simulink model "SIM_EXO_DAL_MN"  (R2021b)
(part 16 of 24)

t3493 = ct{698};
t3496 = ct{699};
t3498 = ct{700};
t3499 = ct{701};
t3500 = ct{702};
t3501 = ct{703};
t3504 = ct{704};
t3506 = ct{705};
t3507 = ct{706};
t3510 = ct{707};
t3511 = ct{708};
t3513 = ct{709};
t3514 = ct{710};
t3515 = ct{711};
t3517 = ct{712};
t3518 = ct{713};
t3521 = ct{714};
t3522 = ct{715};
t3523 = ct{716};
t3526 = ct{717};
t3530 = ct{718};
t3531 = ct{719};
t3532 = ct{720};
t3535 = ct{721};
t3536 = ct{722};
t3539 = ct{723};
t3540 = ct{724};
t3542 = ct{725};
t3543 = ct{726};
t3547 = ct{727};
t3554 = ct{728};
t3556 = ct{729};
t3557 = ct{730};
t356 = ct{731};
t3562 = ct{732};
t3568 = ct{733};
t3569 = ct{734};
t357 = ct{735};
t3571 = ct{736};
t3574 = ct{737};
t3577 = ct{738};
t3578 = ct{739};
t358 = ct{740};
t3582 = ct{741};
t3583 = ct{742};
t3584 = ct{743};
t3585 = ct{744};
t3592 = ct{745};
t3593 = ct{746};
t3605 = ct{747};
t3606 = ct{748};
t3607 = ct{749};
t361 = ct{750};
t3610 = ct{751};
t3611 = ct{752};
t3612 = ct{753};
t3618 = ct{754};
t3634 = ct{755};
t3635 = ct{756};
t3637 = ct{757};
t3642 = ct{758};
t3644 = ct{759};
t3656 = ct{760};
t3658 = ct{761};
t3659 = ct{762};
t3662 = ct{763};
t3666 = ct{764};
t3667 = ct{765};
t3668 = ct{766};
t3673 = ct{767};
t3678 = ct{768};
t3682 = ct{769};
t3694 = ct{770};
t3702 = ct{771};
t3706 = ct{772};
t3708 = ct{773};
t371 = ct{774};
t3719 = ct{775};
t372 = ct{776};
t3725 = ct{777};
t3726 = ct{778};
t373 = ct{779};
t3732 = ct{780};
t3733 = ct{781};
t3734 = ct{782};
t3738 = ct{783};
t374 = ct{784};
t3743 = ct{785};
t3746 = ct{786};
t3753 = ct{787};
t3755 = ct{788};
t3757 = ct{789};
t3759 = ct{790};
t3761 = ct{791};
t3763 = ct{792};
t3765 = ct{793};
t3767 = ct{794};
t377 = ct{795};
t3772 = ct{796};
t378 = ct{797};
t3783 = ct{798};
t3785 = ct{799};
t3788 = ct{800};
t379 = ct{801};
t3792 = ct{802};
t3819 = ct{803};
t3821 = ct{804};
t3822 = ct{805};
t3824 = ct{806};
t3831 = ct{807};
t3843 = ct{808};
t3845 = ct{809};
t3851 = ct{810};
t3852 = ct{811};
t3863 = ct{812};
t3869 = ct{813};
t3871 = ct{814};
t3873 = ct{815};
t3874 = ct{816};
t3875 = ct{817};
t3876 = ct{818};
t3882 = ct{819};
t3884 = ct{820};
t3889 = ct{821};
t3890 = ct{822};
t3891 = ct{823};
t3907 = ct{824};
t391 = ct{825};
t3910 = ct{826};
t3913 = ct{827};
t3921 = ct{828};
t3922 = ct{829};
t3923 = ct{830};
t3944 = ct{831};
t395 = ct{832};
t3951 = ct{833};
t3954 = ct{834};
t3956 = ct{835};
t3957 = ct{836};
t3959 = ct{837};
t3960 = ct{838};
t3968 = ct{839};
t3969 = ct{840};
t3971 = ct{841};
t3972 = ct{842};
t3976 = ct{843};
t3978 = ct{844};
t3979 = ct{845};
t3992 = ct{846};
t3993 = ct{847};
t3995 = ct{848};
t3997 = ct{849};
t4 = ct{850};
t4000 = ct{851};
t4004 = ct{852};
t401 = ct{853};
t4010 = ct{854};
t4011 = ct{855};
t4014 = ct{856};
t4015 = ct{857};
t402 = ct{858};
t403 = ct{859};
t406 = ct{860};
t4089 = ct{861};
t4099 = ct{862};
t410 = ct{863};
t4100 = ct{864};
t4103 = ct{865};
t4108 = ct{866};
t411 = ct{867};
t4113 = ct{868};
t4115 = ct{869};
t4118 = ct{870};
t4119 = ct{871};
t4121 = ct{872};
t4123 = ct{873};
t4126 = ct{874};
t413 = ct{875};
t4132 = ct{876};
t4134 = ct{877};
t4138 = ct{878};
t414 = ct{879};
t4143 = ct{880};
t4146 = ct{881};
t4148 = ct{882};
t4152 = ct{883};
t4153 = ct{884};
t4158 = ct{885};
t4166 = ct{886};
t4173 = ct{887};
t4178 = ct{888};
t4179 = ct{889};
t418 = ct{890};
t4181 = ct{891};
t4183 = ct{892};
t4185 = ct{893};
t4190 = ct{894};
t4196 = ct{895};
t4197 = ct{896};
t4206 = ct{897};
t4208 = ct{898};
t4210 = ct{899};
t4217 = ct{900};
t422 = ct{901};
t4221 = ct{902};
t4223 = ct{903};
t4226 = ct{904};
t4228 = ct{905};
t423 = ct{906};
t4230 = ct{907};
t4232 = ct{908};
t4234 = ct{909};
t424 = ct{910};
t4243 = ct{911};
t4249 = ct{912};
t425 = ct{913};
t4251 = ct{914};
t4254 = ct{915};
t4255 = ct{916};
t4259 = ct{917};
t4261 = ct{918};
t4263 = ct{919};
t427 = ct{920};
t4274 = ct{921};
t4276 = ct{922};
t4278 = ct{923};
t4279 = ct{924};
t428 = ct{925};
t4285 = ct{926};
t4286 = ct{927};
t429 = ct{928};
t4293 = ct{929};
t4298 = ct{930};
t4301 = ct{931};
t4304 = ct{932};
t4306 = ct{933};
t431 = ct{934};
t4317 = ct{935};
t4318 = ct{936};
t432 = ct{937};
t4327 = ct{938};
t4329 = ct{939};
t433 = ct{940};
t4332 = ct{941};
t4335 = ct{942};
t4337 = ct{943};
t4339 = ct{944};
t434 = ct{945};
t4342 = ct{946};
t4344 = ct{947};
t4345 = ct{948};
t4347 = ct{949};
t4348 = ct{950};
t4349 = ct{951};
t435 = ct{952};
t4350 = ct{953};
t436 = ct{954};
t4369 = ct{955};
t4370 = ct{956};
t4378 = ct{957};
t4380 = ct{958};
t4382 = ct{959};
t4385 = ct{960};
t4388 = ct{961};
t4392 = ct{962};
t4394 = ct{963};
t4395 = ct{964};
t4396 = ct{965};
t4397 = ct{966};
t440 = ct{967};
t4402 = ct{968};
t4403 = ct{969};
t4405 = ct{970};
t4406 = ct{971};
t4407 = ct{972};
t441 = ct{973};
t4410 = ct{974};
t4412 = ct{975};
t4413 = ct{976};
t4414 = ct{977};
t4416 = ct{978};
t4417 = ct{979};
t4418 = ct{980};
t4419 = ct{981};
t442 = ct{982};
t4420 = ct{983};
t4423 = ct{984};
t4425 = ct{985};
t4426 = ct{986};
t4428 = ct{987};
t4429 = ct{988};
t4431 = ct{989};
t4436 = ct{990};
t4437 = ct{991};
t444 = ct{992};
t4440 = ct{993};
t4444 = ct{994};
t4446 = ct{995};
t4447 = ct{996};
t4449 = ct{997};
t445 = ct{998};
t4450 = ct{999};
t4453 = ct{1000};
t4462 = ct{1001};
t4467 = ct{1002};
t4468 = ct{1003};
t4469 = ct{1004};
t4471 = ct{1005};
t4473 = ct{1006};
t4475 = ct{1007};
t4478 = ct{1008};
t4479 = ct{1009};
t448 = ct{1010};
t4482 = ct{1011};
t4483 = ct{1012};
t4485 = ct{1013};
t4486 = ct{1014};
t4487 = ct{1015};
t4488 = ct{1016};
t4489 = ct{1017};
t449 = ct{1018};
t4490 = ct{1019};
t4494 = ct{1020};
t4495 = ct{1021};
t4498 = ct{1022};
t4499 = ct{1023};
t450 = ct{1024};
t4500 = ct{1025};
t4501 = ct{1026};
t4502 = ct{1027};
t4505 = ct{1028};
t4506 = ct{1029};
t4509 = ct{1030};
t4510 = ct{1031};
t4515 = ct{1032};
t4518 = ct{1033};
t4519 = ct{1034};
t452 = ct{1035};
t4520 = ct{1036};
t4521 = ct{1037};
t4522 = ct{1038};
t4523 = ct{1039};
t4526 = ct{1040};
t4527 = ct{1041};
t4528 = ct{1042};
t453 = ct{1043};
t4530 = ct{1044};
t4534 = ct{1045};
t4536 = ct{1046};
t4538 = ct{1047};
t454 = ct{1048};
t4541 = ct{1049};
t4543 = ct{1050};
t4545 = ct{1051};
t4546 = ct{1052};
t4549 = ct{1053};
t4551 = ct{1054};
t4552 = ct{1055};
t4553 = ct{1056};
t4556 = ct{1057};
t4557 = ct{1058};
t4558 = ct{1059};
t4559 = ct{1060};
t4565 = ct{1061};
t4568 = ct{1062};
t457 = ct{1063};
t4570 = ct{1064};
t4572 = ct{1065};
t4575 = ct{1066};
t4577 = ct{1067};
t4578 = ct{1068};
t458 = ct{1069};
t4581 = ct{1070};
t4582 = ct{1071};
t4586 = ct{1072};
t4587 = ct{1073};
t4588 = ct{1074};
t4589 = ct{1075};
t459 = ct{1076};
t4590 = ct{1077};
t4591 = ct{1078};
t4592 = ct{1079};
t4593 = ct{1080};
t4595 = ct{1081};
t4596 = ct{1082};
t4598 = ct{1083};
t460 = ct{1084};
t4600 = ct{1085};
t4601 = ct{1086};
t4602 = ct{1087};
t4604 = ct{1088};
t4605 = ct{1089};
t4606 = ct{1090};
t4607 = ct{1091};
t4608 = ct{1092};
t4614 = ct{1093};
t4616 = ct{1094};
t4619 = ct{1095};
t4621 = ct{1096};
t4622 = ct{1097};
t4623 = ct{1098};
t4624 = ct{1099};
t4625 = ct{1100};
t4626 = ct{1101};
t4629 = ct{1102};
t463 = ct{1103};
t4633 = ct{1104};
t4634 = ct{1105};
t4636 = ct{1106};
t4644 = ct{1107};
t4645 = ct{1108};
t4647 = ct{1109};
t4648 = ct{1110};
t4654 = ct{1111};
t4656 = ct{1112};
t4659 = ct{1113};
t4660 = ct{1114};
t4666 = ct{1115};
t4667 = ct{1116};
t4669 = ct{1117};
t4673 = ct{1118};
t4674 = ct{1119};
t4675 = ct{1120};
t4678 = ct{1121};
t468 = ct{1122};
t4682 = ct{1123};
t469 = ct{1124};
t4694 = ct{1125};
t4695 = ct{1126};
t4696 = ct{1127};
t4697 = ct{1128};
t470 = ct{1129};
t4707 = ct{1130};
t4708 = ct{1131};
t472 = ct{1132};
t4724 = ct{1133};
t4727 = ct{1134};
t4728 = ct{1135};
t4731 = ct{1136};
t4732 = ct{1137};
t4733 = ct{1138};
t4737 = ct{1139};
t4738 = ct{1140};
t4739 = ct{1141};
t4742 = ct{1142};
t4743 = ct{1143};
t4745 = ct{1144};
t4747 = ct{1145};
t4748 = ct{1146};
t475 = ct{1147};
t4755 = ct{1148};
t4756 = ct{1149};
t4762 = ct{1150};
t477 = ct{1151};
t4773 = ct{1152};
t4775 = ct{1153};
t4780 = ct{1154};
t4781 = ct{1155};
t4782 = ct{1156};
t4783 = ct{1157};
t4785 = ct{1158};
t4786 = ct{1159};
t479 = ct{1160};
t480 = ct{1161};
t481 = ct{1162};
t4810 = ct{1163};
t482 = ct{1164};
t4824 = ct{1165};
t483 = ct{1166};
t4838 = ct{1167};
t4842 = ct{1168};
t485 = ct{1169};
t486 = ct{1170};
t4864 = ct{1171};
t4866 = ct{1172};
t4869 = ct{1173};
t4870 = ct{1174};
t488 = ct{1175};
t4884 = ct{1176};
t489 = ct{1177};
t4903 = ct{1178};
t4904 = ct{1179};
t491 = ct{1180};
t4911 = ct{1181};
t4914 = ct{1182};
t4919 = ct{1183};
t492 = ct{1184};
t493 = ct{1185};
t4934 = ct{1186};
t4936 = ct{1187};
t494 = ct{1188};
t4950 = ct{1189};
t4953 = ct{1190};
t4957 = ct{1191};
t496 = ct{1192};
t4973 = ct{1193};
t498 = ct{1194};
t4981 = ct{1195};
t4983 = ct{1196};
t4984 = ct{1197};
t4987 = ct{1198};
t4990 = ct{1199};
t4993 = ct{1200};
t4994 = ct{1201};
t4995 = ct{1202};
t4996 = ct{1203};
t5 = ct{1204};
t50 = ct{1205};
t500 = ct{1206};
t5000 = ct{1207};
t5002 = ct{1208};
t5007 = ct{1209};
t5008 = ct{1210};
t5009 = ct{1211};
t5021 = ct{1212};
t5022 = ct{1213};
t5023 = ct{1214};
t5026 = ct{1215};
t5027 = ct{1216};
t5032 = ct{1217};
t5039 = ct{1218};
t5058 = ct{1219};
t5061 = ct{1220};
t5063 = ct{1221};
t5065 = ct{1222};
t5075 = ct{1223};
t5076 = ct{1224};
t508 = ct{1225};
t5080 = ct{1226};
t5084 = ct{1227};
t509 = ct{1228};
t5097 = ct{1229};
t5099 = ct{1230};
t510 = ct{1231};
t5102 = ct{1232};
t5107 = ct{1233};
t5112 = ct{1234};
t5114 = ct{1235};
t512 = ct{1236};
t5121 = ct{1237};
t5123 = ct{1238};
t513 = ct{1239};
t5132 = ct{1240};
t5136 = ct{1241};
t514 = ct{1242};
t5147 = ct{1243};
t5150 = ct{1244};
t5151 = ct{1245};
t516 = ct{1246};
t5164 = ct{1247};
t5166 = ct{1248};
t517 = ct{1249};
t518 = ct{1250};
t5184 = ct{1251};
t5195 = ct{1252};
t520 = ct{1253};
t5203 = ct{1254};
t5204 = ct{1255};
t5206 = ct{1256};
t521 = ct{1257};
t5210 = ct{1258};
t5215 = ct{1259};
t5217 = ct{1260};
t5219 = ct{1261};
t522 = ct{1262};
t5227 = ct{1263};
t5228 = ct{1264};
t523 = ct{1265};
t5232 = ct{1266};
t5233 = ct{1267};
t5236 = ct{1268};
t5238 = ct{1269};
t524 = ct{1270};
t5242 = ct{1271};
t5244 = ct{1272};
t5249 = ct{1273};
t525 = ct{1274};
t5251 = ct{1275};
t5255 = ct{1276};
t5258 = ct{1277};
t5259 = ct{1278};
t5262 = ct{1279};
t5269 = ct{1280};
t527 = ct{1281};
t5275 = ct{1282};
t5279 = ct{1283};
t5280 = ct{1284};
t5285 = ct{1285};
t529 = ct{1286};
t5297 = ct{1287};
t53 = ct{1288};
t531 = ct{1289};
t5316 = ct{1290};
t5318 = ct{1291};
t532 = ct{1292};
t5320 = ct{1293};
t5323 = ct{1294};
t5324 = ct{1295};
t533 = ct{1296};
t5333 = ct{1297};
t5339 = ct{1298};
t534 = ct{1299};
t5344 = ct{1300};
t535 = ct{1301};
t5354 = ct{1302};
t536 = ct{1303};
t5370 = ct{1304};
t539 = ct{1305};
t540 = ct{1306};
t543 = ct{1307};
t5443 = ct{1308};
t545 = ct{1309};
t5450 = ct{1310};
t5457 = ct{1311};
t5459 = ct{1312};
t5464 = ct{1313};
t5465 = ct{1314};
t5466 = ct{1315};
t547 = ct{1316};
t548 = ct{1317};
t5480 = ct{1318};
t5482 = ct{1319};
t5483 = ct{1320};
t5484 = ct{1321};
t5486 = ct{1322};
t5487 = ct{1323};
t5488 = ct{1324};
t549 = ct{1325};
t5507 = ct{1326};
t552 = ct{1327};
t5521 = ct{1328};
t553 = ct{1329};
t559 = ct{1330};
t560 = ct{1331};
t5602 = ct{1332};
t5605 = ct{1333};
t561 = ct{1334};
t5621 = ct{1335};
t5622 = ct{1336};
t563 = ct{1337};
t5633 = ct{1338};
t5634 = ct{1339};
t5636 = ct{1340};
t564 = ct{1341};
t5647 = ct{1342};
t5648 = ct{1343};
t5657 = ct{1344};
t5658 = ct{1345};
t5662 = ct{1346};
t5665 = ct{1347};
t5666 = ct{1348};
t567 = ct{1349};
t5670 = ct{1350};
t5676 = ct{1351};
t5679 = ct{1352};
t568 = ct{1353};
t5683 = ct{1354};
t5684 = ct{1355};
t5688 = ct{1356};
t5691 = ct{1357};
t5699 = ct{1358};
t5700 = ct{1359};
t5702 = ct{1360};
t5704 = ct{1361};
t5706 = ct{1362};
t5708 = ct{1363};
t5709 = ct{1364};
t5710 = ct{1365};
t5717 = ct{1366};
t5718 = ct{1367};
t572 = ct{1368};
t5729 = ct{1369};
t5730 = ct{1370};
t5735 = ct{1371};
t5738 = ct{1372};
t5739 = ct{1373};
t5740 = ct{1374};
t5742 = ct{1375};
t5744 = ct{1376};
t5756 = ct{1377};
t5757 = ct{1378};
t5766 = ct{1379};
t5767 = ct{1380};
t5769 = ct{1381};
t5770 = ct{1382};
t5772 = ct{1383};
t5774 = ct{1384};
t5775 = ct{1385};
t5776 = ct{1386};
t5778 = ct{1387};
t578 = ct{1388};
t5784 = ct{1389};
t5786 = ct{1390};
t5787 = ct{1391};
t5790 = ct{1392};
t5791 = ct{1393};
t5792 = ct{1394};
t5794 = ct{1395};
t5795 = ct{1396};
t5797 = ct{1397};
t580 = ct{1398};
t5808 = ct{1399};
t581 = ct{1400};
t5810 = ct{1401};
t582 = ct{1402};
t5822 = ct{1403};
t5823 = ct{1404};
t5824 = ct{1405};
t5825 = ct{1406};
t5826 = ct{1407};
t5831 = ct{1408};
t5838 = ct{1409};
t5839 = ct{1410};
t584 = ct{1411};
t5840 = ct{1412};
t5841 = ct{1413};
t5842 = ct{1414};
t5844 = ct{1415};
t5845 = ct{1416};
t5846 = ct{1417};
t5847 = ct{1418};
t5848 = ct{1419};
t5849 = ct{1420};
t5850 = ct{1421};
t5851 = ct{1422};
t5852 = ct{1423};
t586 = ct{1424};
t5861 = ct{1425};
t587 = ct{1426};
t5872 = ct{1427};
t5878 = ct{1428};
t5881 = ct{1429};
t5882 = ct{1430};
t5883 = ct{1431};
t5888 = ct{1432};
t5889 = ct{1433};
t589 = ct{1434};
t5892 = ct{1435};
t5894 = ct{1436};
t5895 = ct{1437};
t5897 = ct{1438};
t5898 = ct{1439};
t5899 = ct{1440};
t590 = ct{1441};
t5900 = ct{1442};
t5905 = ct{1443};
t5907 = ct{1444};
t5909 = ct{1445};
t591 = ct{1446};
t5915 = ct{1447};
t5916 = ct{1448};
t5917 = ct{1449};
t5918 = ct{1450};
t5919 = ct{1451};
t592 = ct{1452};
t5921 = ct{1453};
t5922 = ct{1454};
t5923 = ct{1455};
t5924 = ct{1456};
t5925 = ct{1457};
t5926 = ct{1458};
t5928 = ct{1459};
t5930 = ct{1460};
t5934 = ct{1461};
t5935 = ct{1462};
t5936 = ct{1463};
t5937 = ct{1464};
t5938 = ct{1465};
t5939 = ct{1466};
t594 = ct{1467};
t5940 = ct{1468};
t5941 = ct{1469};
t5942 = ct{1470};
t5943 = ct{1471};
t5944 = ct{1472};
t5947 = ct{1473};
t5949 = ct{1474};
t5950 = ct{1475};
t5951 = ct{1476};
t5952 = ct{1477};
t5953 = ct{1478};
t5954 = ct{1479};
t5956 = ct{1480};
t5958 = ct{1481};
t5959 = ct{1482};
t596 = ct{1483};
t5960 = ct{1484};
t5961 = ct{1485};
t5964 = ct{1486};
t5966 = ct{1487};
t5967 = ct{1488};
t5968 = ct{1489};
t597 = ct{1490};
t5970 = ct{1491};
t5971 = ct{1492};
t5972 = ct{1493};
t5973 = ct{1494};
t5974 = ct{1495};
t5975 = ct{1496};
t5976 = ct{1497};
t5977 = ct{1498};
t5978 = ct{1499};
t5979 = ct{1500};
t5980 = ct{1501};
t5981 = ct{1502};
t5982 = ct{1503};
t5984 = ct{1504};
t5985 = ct{1505};
t5986 = ct{1506};
t5988 = ct{1507};
t5996 = ct{1508};
t5998 = ct{1509};
t5999 = ct{1510};
t6 = ct{1511};
t600 = ct{1512};
t6001 = ct{1513};
t6002 = ct{1514};
t6003 = ct{1515};
t6004 = ct{1516};
t6005 = ct{1517};
t6007 = ct{1518};
t6008 = ct{1519};
t6009 = ct{1520};
t6011 = ct{1521};
t6012 = ct{1522};
t6013 = ct{1523};
t6014 = ct{1524};
t6017 = ct{1525};
t6019 = ct{1526};
t602 = ct{1527};
t6024 = ct{1528};
t6026 = ct{1529};
t6029 = ct{1530};
t603 = ct{1531};
t6030 = ct{1532};
t6032 = ct{1533};
t6035 = ct{1534};
t6037 = ct{1535};
t604 = ct{1536};
t6040 = ct{1537};
t6041 = ct{1538};
t6042 = ct{1539};
t6043 = ct{1540};
t6044 = ct{1541};
t6045 = ct{1542};
t6046 = ct{1543};
t6047 = ct{1544};
t6048 = ct{1545};
t605 = ct{1546};
t6051 = ct{1547};
t6052 = ct{1548};
t6053 = ct{1549};
t6056 = ct{1550};
t6057 = ct{1551};
t6060 = ct{1552};
t6064 = ct{1553};
t6065 = ct{1554};
t6069 = ct{1555};
t6074 = ct{1556};
t6081 = ct{1557};
t609 = ct{1558};
t6095 = ct{1559};
t610 = ct{1560};
t6103 = ct{1561};
t6108 = ct{1562};
t6109 = ct{1563};
t611 = ct{1564};
t6118 = ct{1565};
t6119 = ct{1566};
t612 = ct{1567};
t6121 = ct{1568};
t6123 = ct{1569};
t6125 = ct{1570};
t6127 = ct{1571};
t6128 = ct{1572};
t613 = ct{1573};
t6130 = ct{1574};
t6131 = ct{1575};
t6136 = ct{1576};
t6137 = ct{1577};
t6138 = ct{1578};
t614 = ct{1579};
t6141 = ct{1580};
t6142 = ct{1581};
t6143 = ct{1582};
t6144 = ct{1583};
t6145 = ct{1584};
t6146 = ct{1585};
t6147 = ct{1586};
t615 = ct{1587};
t6150 = ct{1588};
t6151 = ct{1589};
t6152 = ct{1590};
t6154 = ct{1591};
t6155 = ct{1592};
t6157 = ct{1593};
t6158 = ct{1594};
t6159 = ct{1595};
t616 = ct{1596};
t6160 = ct{1597};
t6161 = ct{1598};
t6162 = ct{1599};
t6164 = ct{1600};
t6165 = ct{1601};
t6167 = ct{1602};
t6170 = ct{1603};
t6171 = ct{1604};
t6172 = ct{1605};
t6173 = ct{1606};
t6175 = ct{1607};
t6176 = ct{1608};
t6177 = ct{1609};
t6179 = ct{1610};
t618 = ct{1611};
t6182 = ct{1612};
t6183 = ct{1613};
t6185 = ct{1614};
t6186 = ct{1615};
t6188 = ct{1616};
t6189 = ct{1617};
t619 = ct{1618};
t6190 = ct{1619};
t6191 = ct{1620};
t6194 = ct{1621};
t6195 = ct{1622};
t6196 = ct{1623};
t6197 = ct{1624};
t620 = ct{1625};
t6201 = ct{1626};
t6202 = ct{1627};
t6203 = ct{1628};
t6204 = ct{1629};
t6205 = ct{1630};
t6206 = ct{1631};
t6207 = ct{1632};
t6208 = ct{1633};
t6209 = ct{1634};
t621 = ct{1635};
t6210 = ct{1636};
t6211 = ct{1637};
t6212 = ct{1638};
t6213 = ct{1639};
t6215 = ct{1640};
t6216 = ct{1641};
t6218 = ct{1642};
t622 = ct{1643};
t6220 = ct{1644};
t6222 = ct{1645};
t6225 = ct{1646};
t6226 = ct{1647};
t6228 = ct{1648};
t6229 = ct{1649};
t623 = ct{1650};
t6230 = ct{1651};
t6231 = ct{1652};
t6232 = ct{1653};
t6235 = ct{1654};
t6239 = ct{1655};
t624 = ct{1656};
t6241 = ct{1657};
t6242 = ct{1658};
t6243 = ct{1659};
t6244 = ct{1660};
t6245 = ct{1661};
t6248 = ct{1662};
t6249 = ct{1663};
t625 = ct{1664};
t6251 = ct{1665};
t6252 = ct{1666};
t6255 = ct{1667};
t6256 = ct{1668};
t6260 = ct{1669};
t6267 = ct{1670};
t6268 = ct{1671};
t6270 = ct{1672};
t6271 = ct{1673};
t6272 = ct{1674};
t6274 = ct{1675};
t6275 = ct{1676};
t6276 = ct{1677};
t6278 = ct{1678};
t6280 = ct{1679};
t6281 = ct{1680};
t6282 = ct{1681};
t6283 = ct{1682};
t6284 = ct{1683};
t6285 = ct{1684};
t6288 = ct{1685};
t6289 = ct{1686};
t6290 = ct{1687};
t6292 = ct{1688};
t6293 = ct{1689};
t6294 = ct{1690};
t6295 = ct{1691};
t6296 = ct{1692};
t6297 = ct{1693};
t6299 = ct{1694};
t6300 = ct{1695};
t6303 = ct{1696};
t6306 = ct{1697};
t6307 = ct{1698};
t6309 = ct{1699};
t6311 = ct{1700};
t6312 = ct{1701};
t6313 = ct{1702};
t6316 = ct{1703};
t6317 = ct{1704};
t6318 = ct{1705};
t632 = ct{1706};
t6322 = ct{1707};
t6324 = ct{1708};
t6327 = ct{1709};
t6328 = ct{1710};
t6329 = ct{1711};
t6330 = ct{1712};
t6331 = ct{1713};
t6332 = ct{1714};
t6345 = ct{1715};
t6349 = ct{1716};
t6350 = ct{1717};
t6351 = ct{1718};
t6352 = ct{1719};
t6359 = ct{1720};
t6360 = ct{1721};
t6361 = ct{1722};
t6362 = ct{1723};
t6370 = ct{1724};
t6378 = ct{1725};
t638 = ct{1726};
t6380 = ct{1727};
t6382 = ct{1728};
t6385 = ct{1729};
t6386 = ct{1730};
t6391 = ct{1731};
t6393 = ct{1732};
t6395 = ct{1733};
t6396 = ct{1734};
t6397 = ct{1735};
t6399 = ct{1736};
t640 = ct{1737};
t6400 = ct{1738};
t6401 = ct{1739};
t6402 = ct{1740};
t6404 = ct{1741};
t6405 = ct{1742};
t6406 = ct{1743};
t6407 = ct{1744};
t6408 = ct{1745};
t6412 = ct{1746};
t6414 = ct{1747};
t6422 = ct{1748};
t6426 = ct{1749};
t6427 = ct{1750};
t6431 = ct{1751};
t6432 = ct{1752};
t6433 = ct{1753};
t6434 = ct{1754};
t6435 = ct{1755};
t6442 = ct{1756};
t6443 = ct{1757};
t6444 = ct{1758};
t6445 = ct{1759};
t6446 = ct{1760};
t6449 = ct{1761};
t6451 = ct{1762};
t6454 = ct{1763};
t6462 = ct{1764};
t6463 = ct{1765};
t6465 = ct{1766};
t6468 = ct{1767};
t6470 = ct{1768};
t6471 = ct{1769};
t6473 = ct{1770};
t6476 = ct{1771};
t6477 = ct{1772};
t6482 = ct{1773};
t6486 = ct{1774};
t6487 = ct{1775};
t6488 = ct{1776};
t6489 = ct{1777};
t6492 = ct{1778};
t6498 = ct{1779};
t6501 = ct{1780};
t6503 = ct{1781};
t6504 = ct{1782};
t6507 = ct{1783};
t6513 = ct{1784};
t6521 = ct{1785};
t6536 = ct{1786};
t6537 = ct{1787};
t6544 = ct{1788};
t6546 = ct{1789};
t6547 = ct{1790};
t6548 = ct{1791};
t6549 = ct{1792};
t6551 = ct{1793};
t6555 = ct{1794};
t6556 = ct{1795};
t6557 = ct{1796};
t6560 = ct{1797};
t6561 = ct{1798};
t6562 = ct{1799};
t6563 = ct{1800};
t6564 = ct{1801};
t6566 = ct{1802};
t6567 = ct{1803};
t6569 = ct{1804};
t6571 = ct{1805};
t6574 = ct{1806};
t6576 = ct{1807};
t6578 = ct{1808};
t6579 = ct{1809};
t6580 = ct{1810};
t6582 = ct{1811};
t6585 = ct{1812};
t6586 = ct{1813};
t6593 = ct{1814};
t6594 = ct{1815};
t6595 = ct{1816};
t6599 = ct{1817};
t6600 = ct{1818};
t6601 = ct{1819};
t6602 = ct{1820};
t6603 = ct{1821};
t6604 = ct{1822};
t6605 = ct{1823};
t6606 = ct{1824};
t6607 = ct{1825};
t6608 = ct{1826};
t6610 = ct{1827};
t6616 = ct{1828};
t6620 = ct{1829};
t6621 = ct{1830};
t6631 = ct{1831};
t6632 = ct{1832};
t6642 = ct{1833};
t6646 = ct{1834};
t6648 = ct{1835};
t6649 = ct{1836};
t6650 = ct{1837};
t6654 = ct{1838};
t6656 = ct{1839};
t6657 = ct{1840};
t6659 = ct{1841};
t6660 = ct{1842};
t6663 = ct{1843};
t6664 = ct{1844};
t6665 = ct{1845};
t6669 = ct{1846};
t6672 = ct{1847};
t6676 = ct{1848};
t6677 = ct{1849};
t6694 = ct{1850};
t6695 = ct{1851};
t6699 = ct{1852};
t6709 = ct{1853};
t6710 = ct{1854};
t6711 = ct{1855};
t6712 = ct{1856};
t6713 = ct{1857};
t6714 = ct{1858};
t6715 = ct{1859};
t6717 = ct{1860};
t6718 = ct{1861};
t6719 = ct{1862};
t6720 = ct{1863};
t6721 = ct{1864};
t6724 = ct{1865};
t6727 = ct{1866};
t6728 = ct{1867};
t6729 = ct{1868};
t6730 = ct{1869};
t6733 = ct{1870};
t6738 = ct{1871};
t6741 = ct{1872};
t6742 = ct{1873};
t6743 = ct{1874};
t6744 = ct{1875};
t6745 = ct{1876};
t6746 = ct{1877};
t6747 = ct{1878};
t6749 = ct{1879};
t6750 = ct{1880};
t6751 = ct{1881};
t6752 = ct{1882};
t6753 = ct{1883};
t6756 = ct{1884};
t6758 = ct{1885};
t6759 = ct{1886};
t6761 = ct{1887};
t6763 = ct{1888};
t6765 = ct{1889};
t6771 = ct{1890};
t6772 = ct{1891};
t6774 = ct{1892};
t6776 = ct{1893};
t6783 = ct{1894};
t6787 = ct{1895};
t6789 = ct{1896};
t6807 = ct{1897};
t681 = ct{1898};
t6818 = ct{1899};
t6821 = ct{1900};
t6826 = ct{1901};
t6831 = ct{1902};
t6832 = ct{1903};
t6837 = ct{1904};
t6838 = ct{1905};
t6839 = ct{1906};
t684 = ct{1907};
t6840 = ct{1908};
t6841 = ct{1909};
t6842 = ct{1910};
t6844 = ct{1911};
t6845 = ct{1912};
t6847 = ct{1913};
t6848 = ct{1914};
t6849 = ct{1915};
t6850 = ct{1916};
t6851 = ct{1917};
t6855 = ct{1918};
t6856 = ct{1919};
t6857 = ct{1920};
t6858 = ct{1921};
t6859 = ct{1922};
t6860 = ct{1923};
t6862 = ct{1924};
t6863 = ct{1925};
t6865 = ct{1926};
t6866 = ct{1927};
t6867 = ct{1928};
t6868 = ct{1929};
t6869 = ct{1930};
t6870 = ct{1931};
t6871 = ct{1932};
t6872 = ct{1933};
t6873 = ct{1934};
t6879 = ct{1935};
t6880 = ct{1936};
t6881 = ct{1937};
t6882 = ct{1938};
t6883 = ct{1939};
t6884 = ct{1940};
t6885 = ct{1941};
t6888 = ct{1942};
t6889 = ct{1943};
t6890 = ct{1944};
t6891 = ct{1945};
t6892 = ct{1946};
t6893 = ct{1947};
t6894 = ct{1948};
t6896 = ct{1949};
t6897 = ct{1950};
t6898 = ct{1951};
t6900 = ct{1952};
t6901 = ct{1953};
t6902 = ct{1954};
t6903 = ct{1955};
t6904 = ct{1956};
t6906 = ct{1957};
t6907 = ct{1958};
t6908 = ct{1959};
t6909 = ct{1960};
t6910 = ct{1961};
t6911 = ct{1962};
t6913 = ct{1963};
t6914 = ct{1964};
t6915 = ct{1965};
t6916 = ct{1966};
t6917 = ct{1967};
t6918 = ct{1968};
t6919 = ct{1969};
t6920 = ct{1970};
t6921 = ct{1971};
t6922 = ct{1972};
t6923 = ct{1973};
t6924 = ct{1974};
t6925 = ct{1975};
t6926 = ct{1976};
t6927 = ct{1977};
t6928 = ct{1978};
t6930 = ct{1979};
t6933 = ct{1980};
t6935 = ct{1981};
t6936 = ct{1982};
t6937 = ct{1983};
t6939 = ct{1984};
t6941 = ct{1985};
t6942 = ct{1986};
t6943 = ct{1987};
t6944 = ct{1988};
t6945 = ct{1989};
t6946 = ct{1990};
t6947 = ct{1991};
t6951 = ct{1992};
t6952 = ct{1993};
t6953 = ct{1994};
t6954 = ct{1995};
t6955 = ct{1996};
t6956 = ct{1997};
t6957 = ct{1998};
t6958 = ct{1999};
t6959 = ct{2000};
t6960 = ct{2001};
t6961 = ct{2002};
t6963 = ct{2003};
t6965 = ct{2004};
t6968 = ct{2005};
t6971 = ct{2006};
t6973 = ct{2007};
t6974 = ct{2008};
t6975 = ct{2009};
t6976 = ct{2010};
t6977 = ct{2011};
t6978 = ct{2012};
t6982 = ct{2013};
t6983 = ct{2014};
t6984 = ct{2015};
t6985 = ct{2016};
t6986 = ct{2017};
t6987 = ct{2018};
t6988 = ct{2019};
t6989 = ct{2020};
t6990 = ct{2021};
t6991 = ct{2022};
t6992 = ct{2023};
t6994 = ct{2024};
t6995 = ct{2025};
t6997 = ct{2026};
t7 = ct{2027};
t7000 = ct{2028};
t7001 = ct{2029};
t7003 = ct{2030};
t7004 = ct{2031};
t7006 = ct{2032};
t7007 = ct{2033};
t7008 = ct{2034};
t7009 = ct{2035};
t7010 = ct{2036};
t7011 = ct{2037};
t7012 = ct{2038};
t7013 = ct{2039};
t7015 = ct{2040};
t7016 = ct{2041};
t7017 = ct{2042};
t7018 = ct{2043};
t7020 = ct{2044};
t7022 = ct{2045};
t7023 = ct{2046};
t7024 = ct{2047};
t7025 = ct{2048};
t7026 = ct{2049};
t7027 = ct{2050};
t7028 = ct{2051};
t7029 = ct{2052};
t7030 = ct{2053};
t7031 = ct{2054};
t7032 = ct{2055};
t7033 = ct{2056};
t7034 = ct{2057};
t7035 = ct{2058};
t7036 = ct{2059};
t7039 = ct{2060};
t7040 = ct{2061};
t7041 = ct{2062};
t7042 = ct{2063};
t7044 = ct{2064};
t7045 = ct{2065};
t7048 = ct{2066};
t7051 = ct{2067};
t7052 = ct{2068};
t7053 = ct{2069};
t7054 = ct{2070};
t7055 = ct{2071};
t7056 = ct{2072};
t7057 = ct{2073};
t7059 = ct{2074};
t7060 = ct{2075};
t7061 = ct{2076};
t7064 = ct{2077};
t7066 = ct{2078};
t7067 = ct{2079};
t7068 = ct{2080};
t7069 = ct{2081};
t7070 = ct{2082};
t7071 = ct{2083};
t7072 = ct{2084};
t7073 = ct{2085};
t7074 = ct{2086};
t7075 = ct{2087};
t7076 = ct{2088};
t7077 = ct{2089};
t7078 = ct{2090};
t7081 = ct{2091};
t7082 = ct{2092};
t7083 = ct{2093};
t7084 = ct{2094};
t7085 = ct{2095};
t7086 = ct{2096};
t7087 = ct{2097};
t7088 = ct{2098};
t7089 = ct{2099};
t7090 = ct{2100};
t7091 = ct{2101};
t7092 = ct{2102};
t7093 = ct{2103};
t7094 = ct{2104};
t7095 = ct{2105};
t7096 = ct{2106};
t7097 = ct{2107};
t7098 = ct{2108};
t7099 = ct{2109};
t7100 = ct{2110};
t7101 = ct{2111};
t7102 = ct{2112};
t7103 = ct{2113};
t7104 = ct{2114};
t7108 = ct{2115};
t7110 = ct{2116};
t7111 = ct{2117};
t7113 = ct{2118};
t7114 = ct{2119};
t7115 = ct{2120};
t7116 = ct{2121};
t712 = ct{2122};
t7120 = ct{2123};
t7121 = ct{2124};
t7122 = ct{2125};
t7123 = ct{2126};
t7124 = ct{2127};
t7126 = ct{2128};
t7127 = ct{2129};
t7128 = ct{2130};
t7129 = ct{2131};
t7130 = ct{2132};
t7131 = ct{2133};
t7133 = ct{2134};
t7134 = ct{2135};
t7135 = ct{2136};
t7137 = ct{2137};
t7139 = ct{2138};
t7140 = ct{2139};
t7141 = ct{2140};
t7142 = ct{2141};
t7143 = ct{2142};
t7144 = ct{2143};
t7145 = ct{2144};
t7146 = ct{2145};
t7147 = ct{2146};
t7148 = ct{2147};
t7149 = ct{2148};
t7150 = ct{2149};
t7155 = ct{2150};
t7156 = ct{2151};
t7160 = ct{2152};
t7164 = ct{2153};
t7165 = ct{2154};
t7166 = ct{2155};
t7168 = ct{2156};
t7169 = ct{2157};
t7170 = ct{2158};
t7171 = ct{2159};
t7173 = ct{2160};
t7174 = ct{2161};
t7175 = ct{2162};
t7176 = ct{2163};
t7179 = ct{2164};
t7180 = ct{2165};
t7182 = ct{2166};
t7183 = ct{2167};
t7185 = ct{2168};
t7187 = ct{2169};
t7191 = ct{2170};
t7192 = ct{2171};
t7193 = ct{2172};
t7194 = ct{2173};
t7195 = ct{2174};
t7196 = ct{2175};
t72 = ct{2176};
t7200 = ct{2177};
t7208 = ct{2178};
t7209 = ct{2179};
t7210 = ct{2180};
t7215 = ct{2181};
t7217 = ct{2182};
t7218 = ct{2183};
t7219 = ct{2184};
t7221 = ct{2185};
t7223 = ct{2186};
t7224 = ct{2187};
t7225 = ct{2188};
t7226 = ct{2189};
t7231 = ct{2190};
t7233 = ct{2191};
t7235 = ct{2192};
t7237 = ct{2193};
t7238 = ct{2194};
t7239 = ct{2195};
t724 = ct{2196};
t7240 = ct{2197};
t7241 = ct{2198};
t7243 = ct{2199};
t7244 = ct{2200};
t7247 = ct{2201};
t7248 = ct{2202};
t7249 = ct{2203};
t7255 = ct{2204};
t7256 = ct{2205};
t7257 = ct{2206};
t7258 = ct{2207};
t7259 = ct{2208};
t7260 = ct{2209};
t7261 = ct{2210};
t7262 = ct{2211};
t7263 = ct{2212};
t7265 = ct{2213};
t7266 = ct{2214};
t7267 = ct{2215};
t7269 = ct{2216};
t7270 = ct{2217};
t7271 = ct{2218};
t7272 = ct{2219};
t7273 = ct{2220};
t7274 = ct{2221};
t7275 = ct{2222};
t7276 = ct{2223};
t7280 = ct{2224};
t7281 = ct{2225};
t7284 = ct{2226};
t7285 = ct{2227};
t7289 = ct{2228};
t7290 = ct{2229};
t7291 = ct{2230};
t7294 = ct{2231};
t7296 = ct{2232};
t7297 = ct{2233};
t7298 = ct{2234};
t7299 = ct{2235};
t73 = ct{2236};
t7300 = ct{2237};
t7301 = ct{2238};
t7302 = ct{2239};
t7303 = ct{2240};
t7304 = ct{2241};
t7305 = ct{2242};
t7307 = ct{2243};
t7308 = ct{2244};
t7309 = ct{2245};
t7310 = ct{2246};
t7311 = ct{2247};
t7314 = ct{2248};
t7315 = ct{2249};
t7319 = ct{2250};
t7320 = ct{2251};
t7321 = ct{2252};
t7322 = ct{2253};
t7323 = ct{2254};
t7324 = ct{2255};
t7326 = ct{2256};
t7327 = ct{2257};
t7331 = ct{2258};
t7334 = ct{2259};
t7335 = ct{2260};
t7337 = ct{2261};
t7339 = ct{2262};
t7341 = ct{2263};
t7342 = ct{2264};
t7343 = ct{2265};
t7347 = ct{2266};
t7351 = ct{2267};
t7354 = ct{2268};
t7355 = ct{2269};
t7357 = ct{2270};
t7358 = ct{2271};
t7360 = ct{2272};
t7362 = ct{2273};
t7363 = ct{2274};
t7364 = ct{2275};
t7366 = ct{2276};
t7367 = ct{2277};
t7374 = ct{2278};
t7375 = ct{2279};
t738 = ct{2280};
t7386 = ct{2281};
t7387 = ct{2282};
t7388 = ct{2283};
t739 = ct{2284};
t7397 = ct{2285};
t7400 = ct{2286};
t7405 = ct{2287};
t7408 = ct{2288};
t741 = ct{2289};
t7411 = ct{2290};
t7414 = ct{2291};
t7415 = ct{2292};
t742 = ct{2293};
t7421 = ct{2294};
t7437 = ct{2295};
t7438 = ct{2296};
t7450 = ct{2297};
t7454 = ct{2298};
t7455 = ct{2299};
t7458 = ct{2300};
t7467 = ct{2301};
t7478 = ct{2302};
t7481 = ct{2303};
t7517 = ct{2304};
t7519 = ct{2305};
t7523 = ct{2306};
t7524 = ct{2307};
t7528 = ct{2308};
t753 = ct{2309};
t7531 = ct{2310};
t7544 = ct{2311};
t7549 = ct{2312};
t7550 = ct{2313};
t7551 = ct{2314};
t7553 = ct{2315};
t7557 = ct{2316};
t7558 = ct{2317};
t7560 = ct{2318};
t7564 = ct{2319};
t7565 = ct{2320};
t7567 = ct{2321};
t7568 = ct{2322};
t7569 = ct{2323};
t7570 = ct{2324};
t7571 = ct{2325};
t7573 = ct{2326};
t7574 = ct{2327};
t7575 = ct{2328};
t7576 = ct{2329};
t7577 = ct{2330};
t7578 = ct{2331};
t7579 = ct{2332};
t7580 = ct{2333};
t7581 = ct{2334};
t760 = ct{2335};
t781 = ct{2336};
t792 = ct{2337};
t796 = ct{2338};
t797 = ct{2339};
t8 = ct{2340};
t803 = ct{2341};
t81 = ct{2342};
t825 = ct{2343};
t826 = ct{2344};
t827 = ct{2345};
t830 = ct{2346};
t832 = ct{2347};
t845 = ct{2348};
t847 = ct{2349};
t848 = ct{2350};
t852 = ct{2351};
t856 = ct{2352};
t86 = ct{2353};
t861 = ct{2354};
t866 = ct{2355};
t868 = ct{2356};
t869 = ct{2357};
t874 = ct{2358};
t875 = ct{2359};
t877 = ct{2360};
t878 = ct{2361};
t881 = ct{2362};
t893 = ct{2363};
t899 = ct{2364};
t9 = ct{2365};
t90 = ct{2366};
t902 = ct{2367};
t903 = ct{2368};
t905 = ct{2369};
t908 = ct{2370};
t909 = ct{2371};
t91 = ct{2372};
t910 = ct{2373};
t911 = ct{2374};
t912 = ct{2375};
t915 = ct{2376};
t917 = ct{2377};
t919 = ct{2378};
t922 = ct{2379};
t925 = ct{2380};
t926 = ct{2381};
t928 = ct{2382};
t929 = ct{2383};
t930 = ct{2384};
t931 = ct{2385};
t932 = ct{2386};
t934 = ct{2387};
t940 = ct{2388};
t944 = ct{2389};
t945 = ct{2390};
t947 = ct{2391};
t95 = ct{2392};
t952 = ct{2393};
t954 = ct{2394};
t955 = ct{2395};
t957 = ct{2396};
t958 = ct{2397};
t968 = ct{2398};
t970 = ct{2399};
t971 = ct{2400};
t972 = ct{2401};
t975 = ct{2402};
t976 = ct{2403};
t984 = ct{2404};
t985 = ct{2405};
t986 = ct{2406};
t989 = ct{2407};
t99 = ct{2408};
t991 = ct{2409};
t998 = ct{2410};
t7389 = (t9.*t5657.*(-t5744+t6232+t6248+t6303+t6322+t6952+t6960+t6983+t6991))./2.0;
t7393 = (t5776.*(-t5744+t6232+t6248+t6303+t6322+t6952+t6960+t6983+t6991))./2.0;
t7395 = (t5840.*(-t5744+t6232+t6248+t6303+t6322+t6952+t6960+t6983+t6991))./2.0;
t7398 = (t6463.*t7362)./2.0;
t7401 = -t7400;
t7402 = t5941+t6173+t6186+t6599+t6603+t6848+t6866+t6897+t6920;
t7406 = -t7405;
t7407 = t8.*t9.*(-t5942+t6171+t6183-t6604+t6831.*1.40259855e-11-t6851+t6903+t6924+t6216.*(t5670+t4.*(t1458-t5665)).*1.45270122047331e-4).*(-3.0./1.0e+3);
t7409 = (t7082.*t7305)./2.0;
t7410 = (t5.*t7408)./2.0;
t7412 = (t7085.*t7304)./2.0;
t7413 = (t9.*t7411)./2.0;
t7416 = (t5872.*t7408)./2.0;
t7418 = t7411.*(t4148+t5.*(t2421-t4158)).*(-1.0./2.0);
t7419 = (t7411.*(t4148+t5.*(t2421-t4158)))./2.0;
t7420 = t5706+t5735+t6228+t6241+t6283+t6292+t6297+t6311+t6942+t6943+t6973+t6974;
t7425 = t6462.*(-t5942+t6171+t6183-t6604+t6831.*1.40259855e-11-t6851+t6903+t6924+t6216.*(t5670+t4.*(t1458-t5665)).*1.45270122047331e-4).*(-1.0./2.0);
et140 = t6008+t6123-t6672+(t5684.*t6468.*(t29-t30))./1.316403645856965e+67-(t5.*t91.*t5824.*t6216)./1.316403645856965e+67;
et141 = (t5.*t5824.*t6230.*(t29-t30))./1.316403645856965e+67;
t7428 = ((et140+et141).*(t5709-t6255+t6282+t6296-t7003+t6216.*(t6218+t5.*(t3136-t5691)).*1.40259855e-11))./2.0;
t7430 = ((t5709-t6255+t6282+t6296-t7003+t6216.*(t6218+t5.*(t3136-t5691)).*1.40259855e-11).*(t6109+t6571+t6574-t6610+t4528.*(t4148+t5.*(t2421-t4158))+(t4838.*t6468.*(t29-t30))./1.316403645856965e+67))./2.0;
t7431 = (t7191.*t7244)./2.0;
t7435 = (t5872.*t7421)./2.0;
t7452 = t313+t509+t536+t560+t591+t6052+t6069+t6130+t6131+t6576+t6579+t6582+t6586+t6620+t6621+t6631+t6632;
t7460 = t7450.*(t4148+t5.*(t2421-t4158)).*(-1.0./2.0);
t7461 = (t7450.*(t4148+t5.*(t2421-t4158)))./2.0;
t7462 = t7362.*(t6313+(t91.*t5824.*(t6218+t5.*(t3136-t5691)))./1.316403645856965e+67+(t5824.*t6470.*(t29-t30))./1.316403645856965e+67).*(-1.0./2.0);
t7465 = (t7244.*t7263)./2.0;
t7470 = t7269.*(t5984+t5988-t6694-t6695+t6230.*(t5878+t9.*(t7.*(t3719-t3788)+(t3.*t34.*t191.*(t29-t30))./8.112963841460668e+31))+t4.*t6465.*(t3136-t5691)).*(-1.0./2.0);
t7471 = (t7269.*(t5984+t5988-t6694-t6695+t6230.*(t5878+t9.*(t7.*(t3719-t3788)+(t3.*t34.*t191.*(t29-t30))./8.112963841460668e+31))+t4.*t6465.*(t3136-t5691)))./2.0;
t7473 = (t7244.*t7305)./2.0;
t7474 = (t7248.*t7304)./2.0;
t7480 = t6275+t6278+t6370+t6378+t6659+t6660+t6663+t6665+t6771+t6772+t6787+t6789;
t7482 = -t7481;
t7484 = t5730+t5740+t5967+t6244+t6249+t6289+t6293+t6307+t6312+t6648+t6656+t6946+t6953+t6977+t6984;
t7485 = (t4.*t9.*(t5676.*(-1.246862701090643e-6)+t5730+t5967+t6244+t6249+t6289+t6293+t6307+t6312+t6648+t6656+t6946+t6953+t6977+t6984))./2.0;
t7486 = t5729+t5739+t5970+t6242+t6251+t6288+t6295+t6306+t6316+t6650+t6657+t6945+t6951+t6976+t6982;
t7491 = (t1429.*(t5676.*(-1.246862701090643e-6)+t5730+t5967+t6244+t6249+t6289+t6293+t6307+t6312+t6648+t6656+t6946+t6953+t6977+t6984))./2.0;
t7494 = (t7129.*t7408)./2.0;
t7495 = (t7130.*t7411)./2.0;
t7497 = (t5872.*(t5676.*(-1.246862701090643e-6)+t5730+t5967+t6244+t6249+t6289+t6293+t6307+t6312+t6648+t6656+t6946+t6953+t6977+t6984))./2.0;
t7500 = t6137+t6138+t6141+t6154+t6837+t6839+t6855+t6857+t6881+t6882+t6906+t6907;
t7501 = (t7191.*(-t5744+t6232+t6248+t6303+t6322+t6952+t6960+t6983+t6991))./2.0;
t7504 = (t7129.*t7421)./2.0;
et142 = t284-t311+t391-t463+t534+t5947-t6009.*1.40259855e-11+t6013.*7.26350610236655e-5-t6194+t6449+t6454-t6513+t6544+t6551;
et143 = t91.*t5684.*(t6218+t5.*(t3136-t5691)).*1.065477564130357e-78-t4.*t7.*t9.*1.07175327657342e-6;
et144 = t5824.*t6222.*(t29-t30).*5.517689141340903e-72;
et145 = t5684.*t6470.*(t29-t30).*1.065477564130357e-78;
t7506 = t7130.*(et142+et143+et144+et145).*(-1.0./2.0);
t7510 = t5907+t6024+t6030+t6041+t6045+t6482+t6498+t6710+t6713+t6718+t6720+t6742+t6745+t6750+t6752;
t7511 = t5909+t6029+t6032+t6040+t6043+t6488+t6501+t6709+t6712+t6717+t6719+t6741+t6744+t6749+t6751;
t7514 = t5905+t6051+t6056+t6057+t6065+t6476+t6487+t6728+t6730+t6733+t6738+t6759+t6761+t6763+t6765;
t7521 = (t7263.*(-t5744+t6232+t6248+t6303+t6322+t6952+t6960+t6983+t6991))./2.0;
t7530 = (t7305.*(-t5744+t6232+t6248+t6303+t6322+t6952+t6960+t6983+t6991))./2.0;
t7533 = t5.*(-t5944+t6118.*1.246862701090643e-6+t6145+t6146+t6152-t6607+t6831.*3.383302988283333e-6-t6838-t6844-t6856+t6884+t6890+t6909+t6914+t6216.*(t5670+t4.*(t1458-t5665)).*6.293113355513489e-13).*(-1.0./2.0);
t7534 = t5949+t6143+t6144+t6159+t6161+t6606+t6608+t6840+t6845+t6858+t6863+t6883+t6889+t6908+t6913;
t7535 = t4.*t9.*(-t5944+t6118.*1.246862701090643e-6+t6145+t6146+t6152-t6607+t6831.*3.383302988283333e-6-t6838-t6844-t6856+t6884+t6890+t6909+t6914+t6216.*(t5670+t4.*(t1458-t5665)).*6.293113355513489e-13).*(-1.0./2.0);
t7540 = t8.*(-t5943+t6170-t6177+t6179+t6189-t6605+t6831.*3.146556677756745e-13+t6847-t6849+t6865+t6898+t6921-t6922+t6216.*(t5670+t4.*(t1458-t5665)).*8.40184101230148e-6+t6465.*(t5670+t4.*(t1458-t5665)).*4.126305279697715e-13).*(-1.0./2.0);
t7541 = (t7129.*(t5676.*(-1.246862701090643e-6)+t5730+t5967+t6244+t6249+t6289+t6293+t6307+t6312+t6648+t6656+t6946+t6953+t6977+t6984))./2.0;
t7543 = t5657.*(-t5943+t6170-t6177+t6179+t6189-t6605+t6831.*3.146556677756745e-13+t6847-t6849+t6865+t6898+t6921-t6922+t6216.*(t5670+t4.*(t1458-t5665)).*8.40184101230148e-6+t6465.*(t5670+t4.*(t1458-t5665)).*4.126305279697715e-13).*(-1.0./2.0);
t7545 = t5872.*(-t5944+t6118.*1.246862701090643e-6+t6145+t6146+t6152-t6607+t6831.*3.383302988283333e-6-t6838-t6844-t6856+t6884+t6890+t6909+t6914+t6216.*(t5670+t4.*(t1458-t5665)).*6.293113355513489e-13).*(-1.0./2.0);
t7546 = (t5872.*(-t5944+t6118.*1.246862701090643e-6+t6145+t6146+t6152-t6607+t6831.*3.383302988283333e-6-t6838-t6844-t6856+t6884+t6890+t6909+t6914+t6216.*(t5670+t4.*(t1458-t5665)).*6.293113355513489e-13))./2.0;
t7552 = t6821.*(-t5943+t6170-t6177+t6179+t6189-t6605+t6831.*3.146556677756745e-13+t6847-t6849+t6865+t6898+t6921-t6922+t6216.*(t5670+t4.*(t1458-t5665)).*8.40184101230148e-6+t6465.*(t5670+t4.*(t1458-t5665)).*4.126305279697715e-13).*(-1.0./2.0);
t7561 = t7129.*(-t5944+t6118.*1.246862701090643e-6+t6145+t6146+t6152-t6607+t6831.*3.383302988283333e-6-t6838-t6844-t6856+t6884+t6890+t6909+t6914+t6216.*(t5670+t4.*(t1458-t5665)).*6.293113355513489e-13).*(-1.0./2.0);
t7562 = (t7129.*(-t5944+t6118.*1.246862701090643e-6+t6145+t6146+t6152-t6607+t6831.*3.383302988283333e-6-t6838-t6844-t6856+t6884+t6890+t6909+t6914+t6216.*(t5670+t4.*(t1458-t5665)).*6.293113355513489e-13))./2.0;
t7572 = t5602+t5621+t5790+t5791+t5792+t5794+t5838+t5844+t5846+t5847+t5849+t5895+t5897+t5968+t5977+t5982+t5996+t6280+t6361+t6362+t6380+t6385+t6442+t6446+t6451+t6560+t6561+t6563+t6564+t6880+t7007+t7009+t7024+t7025;
t7132 = -t7131;
t7136 = -t7135;
t7151 = -t7150;
t7157 = -t7156;
t7158 = (t6349.*t7123)./2.0;
t7161 = (t6352.*t7123)./2.0;
t7167 = (t6463.*t7123)./2.0;
t7188 = -t7187;
t7189 = (t6826.*t7123)./2.0;
t7197 = (t6933.*t7123)./2.0;
t7201 = -t7200;
t7202 = (t3515.*t7192)./2.0;
t7204 = t5700+t6281+t6290+t7133;
t7205 = t5717+t6284+t6299+t7134;
t7211 = -t7210;
t7212 = (t7020.*t7123)./2.0;
t7222 = -t7221;
t7232 = -t7231;
t7234 = -t7233;
t7236 = -t7235;
t7250 = -t7249;
t7251 = (t7061.*t7123)./2.0;
t7268 = (t9.*t7267)./2.0;
t7278 = t9.*t5657.*t7267.*(-1.0./2.0);
t7279 = t5657.*t7270;
t7282 = (t5776.*t7267)./2.0;
t7286 = -t7285;
t7287 = (t5840.*t7267)./2.0;
t7292 = t7267.*(t4148+t5.*(t2421-t4158)).*(-1.0./2.0);
t7293 = (t7267.*(t4148+t5.*(t2421-t4158)))./2.0;
t7295 = -t7294;
t7312 = -t7311;
t7316 = (t5657.*t7309)./2.0;
t7325 = -t7324;
t7328 = t6225+t6229+t6947+t6955+t6978+t6986;
t7329 = t6231+t6245+t6957+t6959+t6988+t6990;
t7330 = t6235+t6243+t6956+t6958+t6987+t6989;
t7332 = (t5925.*t7327)./2.0;
t7336 = (t5939.*t7327)./2.0;
t7338 = -t7337;
t7340 = (t5979.*t7327)./2.0;
t7344 = (t7085.*t7192)./2.0;
t7346 = t5767+t5964+t6267+t6318+t6328+t6642+t6649+t6961+t6992;
t7350 = t8.*t9.*t7347.*(3.0./1.0e+3);
t7352 = -t7351;
t7359 = -t7358;
t7361 = -t7360;
t7368 = -t7367;
t7369 = (t5.*t8.*t7366)./2.0;
t7370 = t5710+t6256+t6268+t6285+t6300+t6968+t6971+t7001+t7004;
t7376 = -t7374;
t7377 = (t432.*t7366)./2.0;
t7378 = (t498.*t7366)./2.0;
t7382 = (t6462.*t7347)./2.0;
t7390 = -t7389;
t7391 = (t5.*t5657.*t7366)./2.0;
t7394 = (t5775.*t7366)./2.0;
t7396 = (t5839.*t7366)./2.0;
t7399 = (t6462.*t7363)./2.0;
t7403 = t5.*t8.*t7402.*(3.0./1.0e+3);
t7404 = t5942+t6176+t6188+t6600+t6604+t6851+t6870+t6904+t6925;
t7417 = -t7416;
t7422 = (t6463.*t7402)./2.0;
t7432 = (t6136.*t7420)./2.0;
t7434 = (t7192.*t7248)./2.0;
t7436 = -t7435;
t7440 = t7327.*(-t5881+t5918+t6412+t6414+(t4.*t5824.*t5861.*(t29-t30))./1.316403645856965e+67+(t4.*t91.*t5824.*(t3136-t5691))./1.316403645856965e+67).*(-1.0./2.0);
t7441 = (t7327.*(-t5881+t5918+t6412+t6414+(t4.*t5824.*t5861.*(t29-t30))./1.316403645856965e+67+(t4.*t91.*t5824.*(t3136-t5691))./1.316403645856965e+67))./2.0;
t7442 = (t7191.*t7267)./2.0;
t7444 = (t7192.*t7269)./2.0;
t7446 = t7347.*(-t6729+t5784.*(t4148+t5.*(t2421-t4158))+(t5824.*t6468.*(t29-t30))./1.316403645856965e+67).*(-1.0./2.0);
t7448 = (t7347.*(-t6729+t5784.*(t4148+t5.*(t2421-t4158))+(t5824.*t6468.*(t29-t30))./1.316403645856965e+67))./2.0;
t7456 = (t5657.*t7452)./2.0;
t7463 = t7363.*(-t6729+t5784.*(t4148+t5.*(t2421-t4158))+(t5824.*t6468.*(t29-t30))./1.316403645856965e+67).*(-1.0./2.0);
t7464 = (t7363.*(-t6729+t5784.*(t4148+t5.*(t2421-t4158))+(t5824.*t6468.*(t29-t30))./1.316403645856965e+67))./2.0;
t7466 = -t7465;
t7468 = (t7176.*t7327)./2.0;
t7469 = (t7263.*t7267)./2.0;
t7475 = -t7474;
t7476 = t7420.*(t6005-t6486+(t5824.*t6230.*(t29-t30))./1.316403645856965e+67).*(-1.0./2.0);
t7477 = (t7420.*(t6005-t6486+(t5824.*t6230.*(t29-t30))./1.316403645856965e+67))./2.0;
t7479 = (t6821.*t7452)./2.0;
t7483 = (t5657.*t7480)./2.0;
t7487 = (t4.*t5.*t7486)./2.0;
t7489 = t5756+t5766+t5966+t6260+t6270+t6309+t6317+t6324+t6327+t6646+t6654+t6963+t6965+t6995+t6997;
t7492 = (t1427.*t7486)./2.0;
t7498 = -t7497;
t7499 = t7486.*(t4148+t5.*(t2421-t4158)).*(-1.0./2.0);
t7502 = (t7192.*t7366)./2.0;
t7505 = -t7504;
t7507 = (t6136.*t7500)./2.0;
t7512 = (t5.*t7510)./2.0;
t7513 = (t9.*t7511)./2.0;
t7515 = (t1429.*t7510)./2.0;
t7516 = (t1427.*t7511)./2.0;
t7522 = t7366.*(t5984+t5988-t6694-t6695+t6230.*(t5878+t9.*(t7.*(t3719-t3788)+(t3.*t34.*t191.*(t29-t30))./8.112963841460668e+31))+t4.*t6465.*(t3136-t5691)).*(-1.0./2.0);
t7525 = (t5872.*t7510)./2.0;
t7527 = t7511.*(t4148+t5.*(t2421-t4158)).*(-1.0./2.0);
t7529 = (t7304.*t7366)./2.0;
t7532 = t5944+t6150+t6151+t6157+t6160+t6602+t6607+t6838+t6844+t6856+t6862+t6885+t6893+t6910+t6917;
t7536 = (t9.*t7534)./2.0;
t7538 = (t4.*t5.*t7534)./2.0;
t7539 = t5943+t6172+t6177+t6185+t6190+t6601+t6605+t6849+t6850+t6867+t6869+t6900+t6901+t6922+t6923;
t7542 = (t7130.*t7486)./2.0;
t7547 = t7534.*(t4148+t5.*(t2421-t4158)).*(-1.0./2.0);
t7548 = (t7534.*(t4148+t5.*(t2421-t4158)))./2.0;
t7554 = (t7129.*t7510)./2.0;
t7555 = (t7130.*t7511)./2.0;
t7563 = (t7130.*t7534)./2.0;
t7582 = t1651+t1736+t1745+t1800+t1913+t2006+t2060+t2066+t2085+t2110+t2118+t2220+t3593+t3678+t3708+t3743+t3759+t3767+t3785+t3824+t3882+t3910+t3913+t3976+t4206+t4226+t4301+t4329+t4332+t4335+t4385+t4526+t7185+t7290+t7291+t7549;
t7590 = t1574+t1602+t1609+t1614+t1616+t1617+t1667+t1783+t1805+t1806+t1863+t1884+t1900+t2568+t2795+t2973+t4210+t4228+t4274+t4344+t4403+t4414+t4418+t4431+t4490+t4495+t4502+t4546+t4552+t5007+t5058+t5238+t5333+t5339+t5370+t5647+t5648+t7051+t7054+t7057+t7064+t7068+t7070+t7088+t7092+t7108+t7115+t7116+t7173+t7175+t7262+t7322+t7323;
t7592 = t7040+t7041+t7095+t7097+t7101+t7103+t7155+t7182+t7183+t7193+t7195+t7260+t7265+t7266+t7409+t7412;
t7190 = -t7189;
t7198 = -t7197;
t7203 = -t7202;
t7206 = t4.*t5.*t7204.*(3.0./1.0e+3);
t7213 = -t7212;
t7242 = (t6350.*t7204)./2.0;
t7245 = (t6351.*t7204)./2.0;
t7252 = -t7251;
t7253 = (t6395.*t7204)./2.0;
t7277 = t5657.*t7268;
t7283 = -t7282;
t7288 = -t7287;
t7317 = -t7316;
t7345 = -t7344;
t7348 = t5.*t8.*t7346.*(3.0./1.0e+3);
t7371 = (t4.*t7370)./2.0;
t7373 = t3.*t4.*t7370.*4.297799892626299e-1;
t7379 = (t349.*t7370)./2.0;
t7381 = (t6463.*t7346)./2.0;
t7384 = t4.*t4119.*t7370.*(-1.0./2.0);
t7385 = (t5622.*t7370)./2.0;
t7392 = t7370.*(t2421-t4158).*(-1.0./2.0);
t7423 = -t7422;
t7426 = (t7204.*t7215)./2.0;
t7429 = (t7204.*t7219)./2.0;
t7433 = -t7432;
t7439 = (t7053.*t7370)./2.0;
t7443 = -t7442;
t7445 = -t7444;
t7447 = t7346.*(t6313+(t91.*t5824.*(t6218+t5.*(t3136-t5691)))./1.316403645856965e+67+(t5824.*t6470.*(t29-t30))./1.316403645856965e+67).*(-1.0./2.0);
t7453 = (t7072.*t7370)./2.0;
t7457 = -t7456;
t7459 = (t7077.*t7370)./2.0;
t7488 = -t7487;
t7490 = (t8.*t7489)./2.0;
t7493 = (t318.*t7489)./2.0;
t7496 = (t5657.*t7489)./2.0;
t7503 = -t7502;
t7508 = (t6821.*t7489)./2.0;
t7526 = -t7525;
t7537 = -t7536;
t7583 = t742+t845+t866+t869+t877+t881+t919+t932+t947+t985+t998+t1031+t1075+t1184+t1213+t1227+t1661+t1831+t1858+t2132+t3321+t3407+t3409+t3430+t3450+t3463+t3468+t3475+t3485+t3490+t3496+t3499+t3507+t3513+t3522+t3526+t3531+t3543+t3569+t3583+t3585+t3618+t3658+t3734+t3738+t3843+t3869+t3871+t3992+t4232+t4369+t4436+t4556+t7142+t7226+t7234+t7237+t7386+t7388;
t7586 = t1530+t1550+t1578+t1581+t1582+t1600+t1674+t1706+t1708+t1754+t1766+t1772+t1793+t1795+t1812+t1823+t1868+t1878+t1892+t1899+t1909+t1941+t1942+t1951+t1952+t1989+t1993+t2026+t2091+t2186+t2199+t2214+t2291+t2298+t2330+t2342+t2466+t2494+t2567+t2571+t2575+t2579+t2589+t2597+t2598+t2611+t2612+t2656+t2684+t2686+t2706+t2741+t2764+t2802+t2893+t2941+t2944+t2965+t3047+t3266+t4178+t4243+t4407+t4446+t4475+t4486+t4487+t4498+t4515+t4538+t4578+t4647+t4781+t5061+t5114+t5121+t5227+t5249+t5258+t5324+t5486+t7052+t7056+t7071+t7090+t7094+t7111+t7121+t7169+t7171+t7209+t7325+t7326;
t7588 = t684+t781+t792+t803+t826+t832+t875+t893+t912+t915+t1088+t1201+t1612+t1734+t1740+t1814+t1833+t1968+t1997+t2004+t2069+t2115+t2133+t2267+t3338+t3375+t3390+t3392+t3400+t3420+t3422+t3435+t3437+t3439+t3446+t3458+t3474+t3483+t3491+t3547+t3556+t3610+t3662+t3706+t3755+t3763+t3792+t3822+t3831+t3852+t3873+t3951+t3957+t3979+t3993+t4249+t4304+t4347+t4447+t4527+t4587+t7259+t7341+t7342+t7406+t7431+t7434;
t7589 = t742+t845+t866+t869+t877+t881+t919+t932+t947+t985+t998+t1031+t1075+t1184+t1213+t1227+t1661+t1758+t1798+t1831+t1858+t1995+t2038+t2068+t2083+t2113+t2132+t2266+t3321+t3407+t3409+t3430+t3450+t3463+t3468+t3475+t3485+t3490+t3496+t3499+t3507+t3513+t3522+t3526+t3531+t3543+t3569+t3583+t3585+t3592+t3618+t3635+t3658+t3734+t3738+t3753+t3761+t3783+t3819+t3843+t3869+t3871+t3956+t3978+t3992+t4183+t4208+t4232+t4259+t4327+t4337+t4369+t4382+t4388+t4436+t4473+t4556+t7296+t7338+t7339+t7387+t7466+t7467;
t7591 = t1584+t1594+t1622+t1697+t1699+t1705+t1707+t1715+t1718+t1748+t1759+t1770+t1777+t1815+t1821+t1839+t1856+t1860+t1886+t1974+t1984+t2008+t2015+t2043+t2050+t2076+t2119+t2134+t2145+t2184+t2191+t2197+t2203+t2224+t2236+t2243+t2253+t2300+t2326+t2333+t2341+t2416+t2694+t2724+t2743+t2753+t2759+t2791+t2800+t2816+t2861+t2906+t2916+t2987+t4153+t4179+t4190+t4217+t4276+t4317+t4318+t4419+t4420+t4437+t4440+t4467+t4468+t4485+t4489+t4494+t4499+t4500+t4505+t4506+t4519+t4521+t4530+t4534+t4536+t4549+t4565+t4577+t4593+t4595+t4602+t4604+t4608+t4623+t4624+t4644+t4645+t4654+t4659+t4660+t4673+t4678+t4682+t4696+t4727+t4738+t4748+t4824+t4842+t4866+t4934+t4950+t4987+t4990+t4995+t5008+t5021+t5039+t5063+t5080+t5084+t5099+t5151+t5166+t5210+t7303+t7359+t7361+t7401+t7473+t7475;
t7594 = t5769+t5923+t5924+t5959+t5960+t5972+t5976+t6121+t6201+t6204+t6211+t6212+t6329+t6331+t6407+t6408+t6444+t6477+t6492+t6594+t6595+t7013+t7017+t7018+t7028+t7029+t7102+t7157+t7158+t7218+t7278+t7280+t7301+t7302+t7320+t7436+t7438+t7454;
t7207 = -t7206;
t7246 = -t7245;
t7254 = -t7253;
t7349 = -t7348;
t7372 = -t7371;
t7380 = -t7379;
t7383 = t4119.*t7371;
t7427 = -t7426;
t7509 = -t7508;
t7584 = t2720+t2737+t2757+t2761+t2771+t2827+t2833+t2851+t2895+t2913+t2922+t2999+t3209+t3224+t4864+t4870+t4953+t4981+t5000+t5009+t5023+t5027+t5075+t5097+t5132+t5136+t5204+t5219+t5236+t5242+t5262+t5279+t5443+t5450+t5457+t5480+t5507+t5521+t6404+t6567+t6569+t7126+t7188+t7190+t7570;
t7585 = t5232+t5275+t5718+t5738+t7035+t7036+t7084+t7086+t7139+t7232+t7236+t7271+t7343+t7345;
t7587 = t1537+t1540+t1584+t1594+t1699+t1705+t1839+t2076+t2145+t2191+t2197+t2300+t2546+t2552+t2576+t2599+t2617+t2655+t2694+t2724+t2743+t2749+t2753+t2759+t2791+t2800+t2816+t2861+t2906+t2916+t2987+t4824+t4866+t4950+t4973+t4987+t4990+t5008+t5021+t5032+t5063+t5084+t5099+t5112+t5166+t5203+t5210+t5215+t5251+t7016+t7145+t7146+t7240+t7241+t7250+t7252+t7293+t7294+t7317;
t7593 = t1494+t1520+t1534+t1706+t4196+t4407+t4487+t4903+t5123+t5605+t5699+t5708+t5774+t5841+t5898+t5900+t5919+t5936+t5952+t5953+t5980+t5981+t5998+t5999+t6004+t6007+t6014+t6064+t6108+t6207+t6208+t6432+t6435+t7099+t7160+t7161+t7180+t7282+t7286+t7298+t7299+t7315+t7417+t7418+t7457;
t7595 = t1526+t1541+t1577+t1590+t1592+t1620+t1625+t1630+t1647+t1656+t1701+t1724+t1762+t1861+t1906+t2027+t2039+t2047+t2077+t2136+t2299+t2549+t2563+t2564+t2565+t2566+t2569+t2574+t2578+t2588+t2615+t2640+t2666+t2748+t2778+t2793+t2812+t2857+t2872+t2918+t2932+t2956+t2973+t3200+t3213+t3247+t4884+t4911+t4957+t4994+t4996+t5076+t5107+t5147+t5150+t5195+t5217+t5233+t5244+t5255+t5269+t5297+t5320+t5344+t5459+t5464+t5466+t5483+t5484+t5488+t5958+t5974+t5978+t6202+t6203+t6507+t6871+t6873+t6896+t6902+t7151+t7196+t7198+t7275+t7277+t7279+t7321+t7355+t7357+t7435+t7437+t7455;
t7596 = t1517+t1530+t1538+t1578+t1582+t1655+t1674+t1708+t1754+t1766+t1772+t1781+t1812+t1823+t1878+t1899+t1917+t1941+t1951+t1989+t1993+t2026+t2091+t2186+t2199+t2214+t2234+t2291+t2298+t2342+t2396+t2466+t2490+t2555+t2567+t2571+t2575+t2579+t2589+t2597+t2598+t2611+t2612+t2641+t2656+t2684+t2686+t2692+t2706+t2722+t2726+t2741+t2755+t2764+t2799+t2802+t2818+t2824+t2825+t2835+t2877+t2893+t2896+t2911+t2921+t2941+t2958+t2977+t3083+t3222+t3239+t3268+t4234+t4410+t4482+t4869+t4914+t4936+t4993+t5002+t5022+t5026+t5061+t5065+t5102+t5114+t5121+t5164+t5184+t5206+t5249+t5280+t5285+t5318+t5465+t5482+t5487+t5917+t6001+t6002+t6003+t6011+t6012+t6471+t6555+t6556+t6566+t6868+t6872+t7132+t7211+t7213+t7225+t7283+t7285+t7314+t7352+t7354+t7416+t7419+t7456;
t7597 = t5797+t5926+t5928+t5937+t5938+t6271+t7242+t7243+t7336+t7381+t7382+t7390+t7391+t7392+t7433+t7496+t7498+t7499;
t7598 = t5848+t5951+t5956+t5971+t5975+t6276+t6547+t6549+t6557+t6562+t7246+t7247+t7332+t7384+t7393+t7394+t7398+t7399+t7482+t7524+t7526+t7527;
t7599 = t6427+t7144+t7147+t7164+t7165+t7166+t7167+t7254+t7255+t7292+t7295+t7316+t7340+t7385+t7395+t7396+t7423+t7425+t7507+t7543+t7546+t7548;
et146 = t4.*(-1.646190906295504e-7);
et147 = t8.*(-2.11749498538388e-7)+t796-t847+t856+t861-t945+t1146+t1598+t1606+t1716+t1829+t1836+t1882+t1967+t1999+t2003+t2053+t2070+t2098+t2142+t2189+t2217+t2257+t2304+t2443+t2483+t2497+t2502+t2544-t3368+t3387+t3405+t3434+t3441-t3453+t3517+t3539+t3642;
et148 = -t3668+t3673+t3702+t3746+t3765+t3821+t3851+t3876+t3889+t3890+t3907+t3923+t3944+t3954+t3959+t3969+t4000+t4113+t4118+t4121+t4138+t4146+t4251+t4306+t4350+t4380+t4471+t4479+t4510+t4570+t4582+t4762+t4773+t4775+t4.*t190.*5.366634249353632e-6;
et149 = t8.*t190.*6.903100404659751e-6;
et150 = t5.*t200.*(-3.146556677756745e-13)-t9.*t199.*8.01825475553694e-7+t5.*t3472-t8.*t34.*t191.*1.187475829122392e-22;
et151 = t4.*t9.*t34.*t191.*(-3.937746659416635e-29)-t8.*t9.*t34.*t191.*7.651846806710377e-23;
et152 = t8.*t19.*t34.*t191.*2.379770328738529e-22-t4.*t5.*t7.*t34.*t191.*2.472625392454631e-23;
et153 = t5.*t8.*t9.*t34.*t191.*(-1.564233326885588e-22);
et154 = t190.*1.574726338046804e-4;
et155 = t197.*(-3.463588104400448e-7);
et156 = t199.*(-5.944037271736172e-7);
et157 = t201.*(-3.866895863139296e-7);
et158 = t202.*3.006216708625446e-7+t2798+t2806+t2880+t3369+t3380+t3462+t3511+t3972+t4450+t4598;
et159 = t2.*t190.*4.797002992829487e-5;
et160 = t4.*t190.*1.068174783661001e-5;
et161 = t5.*t190.*(-7.044279371874937e-7);
et162 = t6.*t190.*1.978778980640035e-4;
et163 = t2.*t196.*(-2.246155783606385e-6);
et164 = t8.*t190.*1.373992979347475e-5;
et165 = t2.*t197.*2.477538195427268e-9;
et166 = t9.*t190.*(-3.828725908394669e-7);
et167 = t5.*t196.*(-2.070527159901866e-7);
et168 = t5.*t197.*1.97108120739817e-13;
et169 = t6.*t196.*(-9.265463995930741e-6);
et170 = t2.*t201.*(-1.796566294495167e-6);
et171 = t6.*t197.*1.021992379861453e-8;
et172 = t2.*t202.*1.396693317797299e-6;
et173 = t5.*t199.*2.081808214526309e-7;
et174 = t5.*t200.*(-1.503068317813338e-13);
et175 = t9.*t196.*3.809458318607861e-7;
et176 = t9.*t197.*1.503068317813338e-13;
et177 = t5.*t202.*3.809458318607861e-7;
et178 = t6.*t201.*(-7.410893064247368e-6);
et179 = t7.*t200.*(-1.093188572509221e-6);
et180 = t17.*t190.*(-1.741644317895444e-6);
et181 = t6.*t202.*5.761404326386517e-6;
et182 = t9.*t199.*(-3.830213761093238e-7);
et183 = t18.*t190.*(-5.185406908527248e-7);
et184 = t8.*t201.*2.81948171692439e-7;
et185 = t9.*t200.*1.97108120739817e-13;
et186 = t19.*t190.*(-7.200154966325453e-7);
et187 = t9.*t202.*2.070527159901866e-7;
et188 = t18.*t197.*6.966059600064303e-7;
et189 = t19.*t199.*1.191219491402018e-6;
et190 = t2.*t4.*t190.*2.349236299369594e-6;
et191 = t4.*t5.*t190.*1.353584159009324e-5;
et192 = t2.*t8.*t190.*3.021822113324163e-6;
et193 = t4.*t6.*t190.*9.690674399615436e-6;
et194 = t4.*t8.*t190.*1.281152254279884e-6;
et195 = t2.*t5.*t196.*(-9.619703863182362e-7);
et196 = t4.*t9.*t190.*7.357037484179466e-6;
et197 = t5.*t9.*t190.*(-1.095406603137407e-6);
et198 = t6.*t8.*t190.*1.246511225866906e-5;
et199 = t2.*t9.*t196.*1.769880715106441e-6;
et200 = t5.*t6.*t196.*(-3.96815841743287e-6);
et201 = t2.*t5.*t202.*1.769880715106441e-6;
et202 = t5.*t7.*t199.*2.764345231392299e-13;
et203 = t6.*t9.*t196.*7.30081420113316e-6;
et204 = t5.*t7.*t200.*3.828725908394669e-7;
et205 = t5.*t17.*t190.*7.044279371874937e-7;
et206 = t2.*t9.*t202.*9.619703863182362e-7;
et207 = t5.*t6.*t202.*7.30081420113316e-6;
et208 = t5.*t9.*t199.*(-7.829937223708732e-7);
et209 = t5.*t18.*t190.*1.408855874374987e-6;
et210 = t5.*t8.*t201.*(-7.660427522186475e-7);
et211 = t7.*t9.*t199.*(-3.625084017661248e-13);
et212 = t7.*t9.*t200.*(-7.044279371874937e-7);
et213 = t9.*t17.*t190.*3.828725908394669e-7;
et214 = t6.*t9.*t202.*3.96815841743287e-6;
et215 = t9.*t18.*t190.*7.657451816789338e-7;
et216 = t8.*t9.*t201.*(-4.163616429052617e-7);
et217 = t5.*t18.*t197.*(-3.94216241479634e-13);
et218 = t9.*t18.*t197.*(-3.006136635626675e-13);
et219 = t17.*t18.*t190.*2.592703454263624e-7;
et220 = t7.*t19.*t200.*2.190813206274814e-6;
et221 = t17.*t19.*t190.*1.440030993265091e-6;
et222 = t2.*t34.*t191.*4.965121091065431e-29;
et223 = t18.*t19.*t190.*1.440030993265091e-6;
et224 = t3.*t34.*t191.*4.303986245035329e-23;
et225 = t8.*t19.*t201.*(-7.829937223708732e-7);
et226 = t6.*t34.*t191.*2.048128230484517e-28;
et227 = t8.*t34.*t191.*1.187475829122392e-22;
et228 = t2.*t4.*t5.*t190.*2.976937004352228e-6;
et229 = t2.*t4.*t9.*t190.*1.618032907912407e-6;
et230 = t4.*t5.*t6.*t190.*1.22799597575967e-5;
et231 = t4.*t5.*t8.*t190.*(-7.250168035322496e-13);
et232 = t4.*t6.*t9.*t190.*6.674437170347525e-6;
et233 = t4.*t8.*t9.*t190.*(-5.528690462784599e-13);
et234 = t4.*t8.*t17.*t190.*(-6.405761271399419e-7);
et235 = t5.*t7.*t9.*t200.*(-1.440030993265091e-6);
et236 = t5.*t9.*t17.*t190.*2.190813206274814e-6;
et237 = t5.*t9.*t18.*t190.*2.190813206274814e-6;
et238 = t5.*t8.*t9.*t201.*(-1.191219491402018e-6);
et239 = t2.*t3.*t34.*t191.*5.382450561195517e-25;
et240 = t5.*t17.*t18.*t190.*(-7.044279371874937e-7);
et241 = t3.*t4.*t34.*t191.*(-1.333145329970004e-21);
et242 = t3.*t5.*t34.*t191.*(-2.341111640349547e-29);
et243 = t2.*t7.*t34.*t191.*4.87977238063116e-22;
et244 = t3.*t6.*t34.*t191.*2.220277963292577e-24;
et245 = t4.*t5.*t34.*t191.*(-3.002769355787804e-29);
et246 = t9.*t17.*t18.*t190.*(-3.828725908394669e-7);
et247 = t3.*t7.*t34.*t191.*3.783721459294254e-22;
et248 = t3.*t8.*t34.*t191.*1.036418850630278e-21;
et249 = t4.*t7.*t34.*t191.*(-7.059909452387201e-23)-t3.*t9.*t34.*t191.*1.785238843466173e-29;
et250 = t5.*t7.*t34.*t191.*7.138318981153782e-22;
et251 = t4.*t9.*t34.*t191.*3.937746659416635e-29-t5.*t8.*t34.*t191.*4.158952615208568e-23;
et252 = t6.*t7.*t34.*t191.*2.01292161617043e-21;
et253 = t7.*t9.*t34.*t191.*(-1.313343246602064e-21);
et254 = t8.*t9.*t34.*t191.*7.651846806710377e-23-t17.*t18.*t19.*t190.*7.200154966325453e-7;
et255 = t3.*t18.*t34.*t191.*(-8.273795699471084e-23);
et256 = t8.*t17.*t34.*t191.*(-2.374951658244784e-22)-t8.*t19.*t34.*t191.*2.379770328738529e-22;
et257 = t4.*t5.*t8.*t17.*t190.*3.625084017661248e-13;
et258 = t4.*t8.*t9.*t17.*t190.*2.764345231392299e-13;
et259 = t2.*t3.*t4.*t34.*t191.*(-3.903039427556765e-22);
et260 = t2.*t3.*t8.*t34.*t191.*3.034315574254804e-22;
et261 = t3.*t4.*t6.*t34.*t191.*(-1.610016168721029e-21);
et262 = t2.*t5.*t7.*t34.*t191.*2.089880210625419e-22;
et263 = t5.*t9.*t17.*t18.*t190.*(-1.095406603137407e-6);
et264 = t3.*t4.*t8.*t34.*t191.*(-3.34878210114812e-23)-t3.*t5.*t7.*t34.*t191.*1.530369361342075e-22;
et265 = t3.*t5.*t8.*t34.*t191.*1.313343246602064e-21;
et266 = t4.*t5.*t7.*t34.*t191.*2.472625392454631e-23;
et267 = t3.*t6.*t8.*t34.*t191.*1.251664818208198e-21;
et268 = t2.*t7.*t9.*t34.*t191.*(-3.84506501891928e-22);
et269 = t5.*t6.*t7.*t34.*t191.*8.620822290548326e-22;
et270 = t3.*t7.*t9.*t34.*t191.*(-8.317905230417136e-23);
et271 = t3.*t8.*t9.*t34.*t191.*7.138318981153782e-22;
et272 = t4.*t7.*t9.*t34.*t191.*(-4.549258542705501e-23)-t5.*t7.*t8.*t34.*t191.*1.785238843466173e-29;
et273 = t5.*t8.*t9.*t34.*t191.*1.564233326885588e-22;
et274 = t6.*t7.*t9.*t34.*t191.*(-1.586101540900623e-21);
et275 = t7.*t8.*t9.*t34.*t191.*2.341111640349547e-29+t3.*t5.*t18.*t34.*t191.*4.682223280699094e-29;
et276 = t4.*t5.*t17.*t34.*t191.*6.005538711575609e-29-t3.*t7.*t18.*t34.*t191.*5.632647031707275e-23;
et277 = t3.*t7.*t19.*t34.*t191.*(-3.128466653771177e-22)+t3.*t9.*t18.*t34.*t191.*3.570477686932346e-29;
et278 = t4.*t7.*t19.*t34.*t191.*1.414846738462756e-22-t4.*t9.*t17.*t34.*t191.*7.875493318833269e-29;
et279 = t5.*t8.*t17.*t34.*t191.*8.317905230417136e-23-t8.*t9.*t17.*t34.*t191.*1.530369361342075e-22;
et280 = t8.*t17.*t19.*t34.*t191.*4.759540657477059e-22;
et281 = t2.*t3.*t5.*t8.*t34.*t191.*3.84506501891928e-22;
et282 = t3.*t4.*t5.*t8.*t34.*t191.*9.098517085411002e-23;
et283 = t2.*t3.*t8.*t9.*t34.*t191.*2.089880210625419e-22;
et284 = t3.*t4.*t7.*t8.*t34.*t191.*1.391651334125335e-22;
et285 = t3.*t5.*t6.*t8.*t34.*t191.*1.586101540900623e-21;
et286 = t3.*t4.*t8.*t9.*t34.*t191.*4.945250784909262e-23-t3.*t5.*t7.*t9.*t34.*t191.*4.759540657477059e-22;
et287 = t4.*t5.*t7.*t9.*t34.*t191.*(-9.299848787979342e-23);
et288 = t3.*t6.*t8.*t9.*t34.*t191.*8.620822290548326e-22;
et289 = t3.*t5.*t7.*t18.*t34.*t191.*1.530369361342075e-22+t3.*t4.*t8.*t19.*t34.*t191.*9.299848787979342e-23;
et290 = t3.*t7.*t9.*t18.*t34.*t191.*8.317905230417136e-23-t5.*t8.*t9.*t17.*t34.*t191.*3.128466653771177e-22;
et291 = t3.*t7.*t18.*t19.*t34.*t191.*1.564233326885588e-22-t3.*t4.*t5.*t7.*t8.*t34.*t191.*7.875493318833269e-29;
et292 = t3.*t4.*t5.*t8.*t9.*t34.*t191.*1.414846738462756e-22-t3.*t4.*t7.*t8.*t9.*t34.*t191.*6.005538711575609e-29;
et293 = t3.*t5.*t7.*t9.*t18.*t34.*t191.*2.379770328738529e-22;
et294 = -dq1.*(t7335+t7575+t7578+t7581+dq6.*t7564)-dq5.*(t7574-dq4.*t7364+dq3.*t7528+dq2.*t7573+dq6.*t7588+dq5.*(et146+et147+et148+et149+et150+et151+et152+et153));
et295 = -dq3.*(t7580+dq5.*t7528+dq4.*t7553+dq2.*t7579+dq6.*t7591+dq3.*(et154+et155+et156+et157+et158+et159+et160+et161+et162+et163+et164+et165+et166+et167+et168+et169+et170+et171+et172+et173+et174+et175+et176+et177+et178+et179+et180+et181+et182+et183+et184+et185+et186+et187+et188+et189+et190+et191+et192+et193+et194+et195+et196+et197+et198+et199+et200+et201+et202+et203+et204+et205+et206+et207+et208+et209+et210+et211+et212+et213+et214+et215+et216+et217+et218+et219+et220+et221+et222+et223+et224+et225+et226+et227+et228+et229+et230+et231+et232+et233+et234+et235+et236+et237+et238+et239+et240+et241+et242+et243+et244+et245+et246+et247+et248+et249+et250+et251+et252+et253+et254+et255+et256+et257+et258+et259+et260+et261+et262+et263+et264+et265+et266+et267+et268+et269+et270+et271+et272+et273+et274+et275+et276+et277+et278+et279+et280+et281+et282+et283+et284+et285+et286+et287+et288+et289+et290+et291+et292+et293));
et296 = -dq4.*(t7577+dq4.*(t739+t830+t847+t878+t905+t909+t925+t929+t945+t954+t955+t1020+t1046+t1076+t1165+t1211+t1228+t1446+t1619+t1660+t1756+t1761+t1797+t1836+t1916+t1925+t1937+t1999+t2053+t2070+t2098+t2106+t2128+t2149+t2189+t2217+t2256+t2257+t2304+t2497+t2502+t2544+t3368+t3418+t3445+t3453+t3471+t3480+t3493+t3500+t3506+t3518+t3536+t3557+t3562+t3568+t3611+t3634+t3644+t3656+t3668+t3673+t3682+t3725+t3733+t3765+t3845+t3876+t3884+t3907+t3921+t3923+t3944+t3954+t3969+t3971+t3995+t3997+t4000+t4010+t4014+t4121+t4138+t4146+t4197+t4223+t4251+t4261+t4263+t4285+t4293+t4298+t4306+t4339+t4350+t4380+t4449+t4453+t4471+t4479+t4483+t4510+t4570+t4582+t4629+t4762+t4773+t4775)-dq5.*t7364+dq3.*t7553+dq2.*t7576+dq6.*t7589)-dq2.*(t7334+t7335+t7575+t7578+t7581+dq6.*t7582)-dq6.*(t7565+dq2.*t7582+dq4.*t7589+dq5.*t7588+dq3.*t7591-dq6.*(-t6821.*t7297+t7129.*t7141-t7130.*t7140+t7130.*t7244+t7129.*t7248));
et297 = t4.*(-6.806468937857363e-8);
et298 = t202.*3.820705072696559e-6;
et299 = t7.*t8.*1.144847168350722e-7;
et300 = t4.*t190.*2.218930330581593e-6-t9.*t5657.*8.01825475553694e-7+t113.*t5657+t5.*t7042+t9.*t7045+t6422.*t7012;
et301 = t3.*t8.*t34.*t191.*4.285257977338449e-22;
et302 = t741+t868+t1568+t1834-t3274-t3391-t3440+t3874+t3891+t4348+t5259+t5742+t5757-t5.*t8.*1.133811468776912e-7;
et303 = t5.*t201.*(-6.364473664374288e-6)+t8.*t3365+t8.*t3449;
et304 = t4.*t5.*t7.*(-1.907069379620846e-7);
et305 = t8.*t9.*t190.*(-6.800564119502148e-6);
et306 = t3.*t4.*t5.*t34.*t191.*(-7.138318981153782e-22);
et307 = t741+t868+t1568+t1834-t3274-t3391-t3440+t3874+t3891+t4348+t5259+t5742+t5757-t5.*t8.*1.133811468776912e-7;
et308 = t5.*t201.*(-6.364473664374288e-6)+t8.*t3365+t8.*t3449;
et309 = t4.*t5.*t7.*(-1.907069379620846e-7);
et310 = t8.*t9.*t190.*(-6.800564119502148e-6);
et311 = t3.*t4.*t5.*t34.*t191.*(-7.138318981153782e-22);
et312 = t7550+dq4.*t7583-dq3.*t7592+dq5.*(t4148.*4.00912737776847e-7-t5275+t7034-t7035+t7083-t7086+t7231+t7235-t7271-t7343+t7344+t5.*(t2421-t4158).*4.00912737776847e-7+t9.*(t2421-t4158).*2.179051830709965e-7+(t6821.*(et307+et308+et309+et310+et311))./2.0);
et313 = dq6.*(t6821.*t7098-t7032.*t7129+t7033.*t7130+t7082.*t7130-t7085.*t7129)+dq1.*(t1651+t1736+t1745+t1800+t1913+t2006+t2060+t2066+t2085+t2110+t2118+t2220+t3593+t3678+t3708+t3743+t3759+t3767+t3785+t3824+t3882+t3910+t3913+t3976+t4206+t4226+t4301+t4329+t4332+t4335+t4385+t4526-t7185-t7290-t7291+t7549);
et314 = t5961-t6215-t6473+(t91.*t5824.*(t5670+t4.*(t1458-t5665)))./1.316403645856965e+67+(t5824.*t6103.*(t29-t30))./1.316403645856965e+67;
et315 = (t5822.*t6230.*(t29-t30))./1.316403645856965e+67;
et316 = t190.*1.262246131350684e-4;
et317 = t197.*(-3.463588506402063e-7);
et318 = t199.*1.206018527392003e-9;
et319 = t201.*(-3.866896262962515e-7);
et320 = t202.*1.763242970313842e-7+t2798+t2806+t2880+t3369+t3380+t3462+t3511+t3972+t4450+t4598;
et321 = t6927.*(-t6729+t5784.*(t4148+t5.*(t2421-t4158))+(t5824.*t6468.*(t29-t30))./1.316403645856965e+67);
et322 = -t6926.*(t6313+(t91.*t5824.*(t6218+t5.*(t3136-t5691)))./1.316403645856965e+67+(t5824.*t6470.*(t29-t30))./1.316403645856965e+67);
et323 = t4.*t190.*6.265189309050023e-6;
et324 = t8.*t190.*1.373993121413441e-5;
et325 = t7.*t200.*2.218030628186568e-9;
et326 = t17.*t190.*(-1.136551384161165e-6);
et327 = t18.*t190.*(-1.46668754075197e-6);
et328 = t8.*t201.*7.974877919012681e-7;
et329 = t18.*t197.*6.966060404067533e-7+t318.*t7078+t1427.*t7069+t1429.*t7067-t7027.*t7274-t7026.*t7276;
et330 = t6699.*(t6005-t6486+(t5824.*t6230.*(t29-t30))./1.316403645856965e+67)+t6919.*(et314+et315)+t4.*t8.*t190.*1.281152402146915e-6;
et331 = t17.*t18.*t190.*7.333437703759851e-7;
et332 = t3.*t34.*t191.*4.303986722504577e-23;
et333 = t8.*t34.*t191.*(-2.409335246872506e-25);
et334 = t4.*t8.*t17.*t190.*(-6.405762010734574e-7);
et335 = t3.*t4.*t34.*t191.*(-1.333145467812469e-21);
et336 = t3.*t7.*t34.*t191.*2.469157346109375e-22;
et337 = t3.*t8.*t34.*t191.*6.078930528964336e-22;
et338 = t4.*t7.*t34.*t191.*1.432423992658101e-25-t3.*t18.*t34.*t191.*8.273796654409578e-23;
et339 = t8.*t17.*t34.*t191.*4.818670493745012e-25-t3.*t4.*t8.*t34.*t191.*9.471999152795786e-23;
et340 = t3.*t7.*t18.*t34.*t191.*(-1.593188995307795e-22)+t3.*t4.*t7.*t8.*t34.*t191.*1.391651494745862e-22;
et341 = -dq4.*(t7567+t7568-dq5.*t7544+dq3.*t7586+dq6.*t7583+dq4.*(t739+t830+t847+t878+t905+t909+t925+t929+t945+t954+t955+t1020+t1046+t1076+t1165+t1211+t1228+t1446+t1619+t1660+t1836+t1937+t2053+t2098+t2128+t2502+t3368+t3418+t3445+t3453+t3471+t3480+t3493+t3500+t3506+t3518+t3536+t3557+t3568+t3611+t3644+t3668+t3682+t3733+t3876+t3921+t3969+t3995+t4000+t4010+t4014+t4146+t4285+t4298+t4350+t4449+t4510+t4582+t4629+t4775));
et342 = dq5.*(t7557+t7558+dq4.*t7544+dq3.*t7590-dq5.*(et297+et298+et299+et300+et301)-dq6.*(t4148.*4.00912737776847e-7-t5275+t7034-t7035+t7083-t7086+t7231+t7235-t7271-t7343+t7344+t5.*(t2421-t4158).*4.00912737776847e-7+t9.*(t2421-t4158).*2.179051830709965e-7+(t6821.*(et302+et303+et304+et305+et306))./2.0));
et343 = -dq6.*(et312+et313)-dq1.*(-t7334+t7551+t7560+t7569+dq3.*t7584)-dq2.*(t7551+t7560+t7569+dq3.*t7570)-dq3.*(t7571+dq1.*t7570+dq4.*t7586-dq5.*t7590-dq6.*t7592+dq3.*(et316+et317+et318+et319+et320+et321+et322+et323+et324+et325+et326+et327+et328+et329+et330+et331+et332+et333+et334+et335+et336+et337+et338+et339+et340));
et344 = t5888+t5795.*(t2088-t4743).*8.081970098144003e-70;
et345 = t5683.*(t197.*(t29-t30).*9.007199254740992e+15+t3.*(t2444-t2449)).*8.081970098144003e-70;
et346 = t5842+t5795.*(t2088-t4743).*3.038581678643136e-64;
et347 = t5683.*(t197.*(t29-t30).*9.007199254740992e+15+t3.*(t2444-t2449)).*3.038581678643136e-64;
et348 = t284-t311+t391-t463+t534+t5947-t6009.*1.40259855e-11+t6013.*7.26350610236655e-5-t6194+t6449+t6454-t6513+t6544+t6551;
et349 = t91.*t5684.*(t6218+t5.*(t3136-t5691)).*1.065477564130357e-78-t4.*t7.*t9.*1.07175327657342e-6;
et350 = t5824.*t6222.*(t29-t30).*5.517689141340903e-72;
et351 = t5684.*t6470.*(t29-t30).*1.065477564130357e-78;
et352 = -t378+t450+t5930.*4.36041e-5+t6013.*4.36041e-5+(t6359.*(et344+et345))./2.0-t8.*t9.*4.097607815548108e-7+t8.*t278+t5.*t7421+t5826.*t6422+(t6401.*(et346+et347))./2.0+t9.*(et348+et349+et350+et351);
et353 = t91.*t5684.*t6216.*3.312365484343079e-72;
et354 = t91.*t5824.*t6213.*(-3.312365484343079e-72);
et355 = t5684.*t6230.*(t29-t30).*(-3.312365484343079e-72);
et356 = t5824.*t6222.*(t29-t30).*3.312365484343079e-72;
et357 = -t231+t275+t469+t553+t6074+t6175-t6676+t5.*t6536+t5684.*t6468.*(t29-t30).*5.520609140571798e-70;
et358 = t5.*t91.*t5824.*t6216.*(-5.520609140571798e-70);
et359 = t199.*1.929908622992788e-6+t1614+t2568+t5333+t5370+t5647+t5648+t5958-t5960+t5974+t5978+t6202+t6203+t6209+t6210-t6329+t6330+t7057+t7068+t7070-t7102+t7108+t7156-t7158+t7217+t7277+t7279+t7300+t7321+t7435+t7437+t7455+(t6462.*(et357+et358))./2.0;
et360 = t8.*t34.*t191.*1.231753771525398e-22;
et361 = t4.*t7.*t34.*t191.*(-2.120917371004926e-22);
et362 = -t235+t315+t413+t539+t543+t567+t6081-t6167+t6182+t6521+t6537-t6677+t5704.*t5784+t91.*t5684.*(t6218+t5.*(t3136-t5691)).*1.015171749786156e-71;
et363 = t5684.*t6468.*(t29-t30).*5.517689141340903e-72;
et364 = t5684.*t6470.*(t29-t30).*1.015171749786156e-71;
et365 = t5.*t91.*t5824.*t6216.*(-5.517689141340903e-72);
et366 = t5.*t5824.*t6230.*(t29-t30).*5.517689141340903e-72;
et367 = t284-t311+t391-t463+t534+t5947-t6009.*1.40259855e-11+t6013.*7.26350610236655e-5-t6194+t6449+t6454-t6513+t6544+t6551;
et368 = t91.*t5684.*(t6218+t5.*(t3136-t5691)).*1.065477564130357e-78-t4.*t7.*t9.*1.07175327657342e-6;
et369 = t5824.*t6222.*(t29-t30).*5.517689141340903e-72;
et370 = t5684.*t6470.*(t29-t30).*1.065477564130357e-78;
et371 = -t302-t309-t371-t379-t427-t452+t6118.*2.179051830709965e-7+t6142+t6155+t6158+t6831.*4.00912737776847e-7-t6841-t6842-t6859+t6888+t6891+t6911+t6915-t7127-t7268-t7270+t7414+t7442+t7444+t7504+t7536+(t6821.*(et362+et363+et364+et365+et366))./2.0;
et372 = (t5.*(-t5944+t6118.*1.246862701090643e-6+t6145+t6146+t6152-t6607+t6831.*3.383302988283333e-6-t6838-t6844-t6856+t6884+t6890+t6909+t6914+t6216.*(t5670+t4.*(t1458-t5665)).*6.293113355513489e-13))./2.0;
et373 = (t5.*(t305-t319+t322+t336+t6345+t6807+t6818-t5.*t7.*t8.*2.908151843953269e-6-t7.*t8.*t9.*1.07175327657342e-6))./2.0+(t7130.*(et367+et368+et369+et370))./2.0;
et374 = -dq4.*(t257+t278+t358+t372+t374+t428+t434+t436+t445+t448+t458+t460+t477+t486+t508+t510+t512+t522+t535+t547+t561+t587+t592+t596+t612+t827+t899+t958+t972-t7076-t7310+t7311+t7397+t7469+t7471+t7479+t7494+t7495)+dq1.*(t7015+t7144+t7147+t7238+t7239+t7249+t7251+t7292+t7295-t7303+t7316+t7358+t7360+t7400-t7473+t7474);
et375 = dq6.*(t7453+t7529+t7530+t7552+t7562+t7563+t6821.*t7309-t7124.*t7130-t7130.*t7267-t7129.*t7269+t7129.*(t305-t319+t322+t336+t6345+t6807+t6818-t5.*t7.*t8.*2.908151843953269e-6-t7.*t8.*t9.*1.07175327657342e-6));
et376 = dq2.*(t6427+t7144+t7147+t7155+t7164+t7165+t7166+t7167+t7260+t7265+t7266+t7292+t7295+t7316+t7409+t7412)-dq5.*(t302+t309+t371+t379+t427+t452+t7073+t7127+t7128+t7268+t7270-t7307-t7308+t7415+t7443+t7445+t7478+t7505+t7506)+dq3.*(t724+t825+t874+t903+t926+t957+t968+t970+t984+t1004+t1016+t1061+t1081+t1095+t1101+t1108+t1144+t1152+t1155+t1170+t1171+t1174+t1193+t1203+t1207+t1215+t1224+t1245+t1254+t1258+t1285+t1288+t1300+t1301+t1323+t1333+t1344+t1345+t1365+t1377+t1380+t1383+t1388+t1409+t1428+t1440+t1692+t1731+t1769+t1847+t1977+t1981);
et377 = t5889+t5795.*(t2088-t4743).*5.344156668414146e-72;
et378 = t5683.*(t197.*(t29-t30).*9.007199254740992e+15+t3.*(t2444-t2449)).*5.344156668414146e-72;
et379 = t5888+t5795.*(t2088-t4743).*8.081970098144003e-70;
et380 = t5683.*(t197.*(t29-t30).*9.007199254740992e+15+t3.*(t2444-t2449)).*8.081970098144003e-70;
et381 = t5892+t5795.*(t2088-t4743).*7.671525497590686e-73;
et382 = t5683.*(t197.*(t29-t30).*9.007199254740992e+15+t3.*(t2444-t2449)).*7.671525497590686e-73;
et383 = -t231+t275+t469+t553+t6074+t6175-t6676+t5.*t6536+t5684.*t6468.*(t29-t30).*5.520609140571798e-70;
et384 = t5.*t91.*t5824.*t6216.*(-5.520609140571798e-70);
et385 = t5882+t5795.*(t2088-t4743).*1.879526485671887e-68;
et386 = t5683.*(t197.*(t29-t30).*9.007199254740992e+15+t3.*(t2444-t2449)).*1.879526485671887e-68;
et387 = t5883+t5795.*(t2088-t4743).*4.121912899099809e-68;
et388 = t5683.*(t197.*(t29-t30).*9.007199254740992e+15+t3.*(t2444-t2449)).*4.121912899099809e-68;
et389 = t1517+t1530+t1538+t1578+t1582+t1655+t1674+t1708+t1754+t1766+t1772+t1781+t1812+t1823+t1878+t1899+t1917+t1941+t1951+t1989+t1993+t2026+t2091+t2186+t2199+t2214+t2234+t2291+t2298+t2342+t2396+t2466+t2490+t2555+t2567+t2571+t2575+t2579+t2589+t2597+t2598+t2611+t2612+t2641+t2656+t2684+t2686+t2706+t2726+t2741+t2764+t2802+t2893+t2911+t2941+t2977+t3083+t3268+t4234+t4410+t4482+t5061+t5102+t5114+t5121+t5249+t5285+t5318+t5487+t5917+t5935-t5980-t5981+t6001+t6002+t6003+t6011+t6012-t6064+t6205+t6206-t7099-t7160-t7161+t7179+t7283+t7285-t7298+t7314+t7416+t7419+t7456;
et390 = (t6462.*(-t337-t500-t552+t6128+t6578+t6585-t6616+t4528.*(t4148+t5.*(t2421-t4158)).*7.26735e-3+t4838.*t6468.*(t29-t30).*5.520609140571798e-70))./2.0;
et391 = t257+t278+t358+t372+t374+t428+t434+t436+t445+t448+t458+t460+t477+t486+t508+t510+t512+t522+t535+t547+t561+t587+t592+t596+t612+t827+t899+t958+t972+t7397-t7403+t7469+t7471+t7479+t7494+t7495-t7538;
et392 = (t8.*(-t5943+t6170-t6177+t6179+t6189-t6605+t6831.*3.146556677756745e-13+t6847-t6849+t6865+t6898+t6921-t6922+t6216.*(t5670+t4.*(t1458-t5665)).*8.40184101230148e-6+t6465.*(t5670+t4.*(t1458-t5665)).*4.126305279697715e-13))./2.0;
et393 = t8.*t9.*(-t5942+t6171+t6183-t6604+t6831.*1.40259855e-11-t6851+t6903+t6924+t6216.*(t5670+t4.*(t1458-t5665)).*1.45270122047331e-4).*(3.0./1.0e+3);
et394 = (t4.*t9.*(-t5944+t6118.*1.246862701090643e-6+t6145+t6146+t6152-t6607+t6831.*3.383302988283333e-6-t6838-t6844-t6856+t6884+t6890+t6909+t6914+t6216.*(t5670+t4.*(t1458-t5665)).*6.293113355513489e-13))./2.0;
et395 = t3.*6.334299027523179e-7;
et396 = t7.*2.783427048984746e-6-t378+t401+t450-t472-t527+t572;
et397 = t3.*t4.*(-6.689200410011394e-6);
et398 = t3.*t8.*5.200343311959535e-6-t4.*t7.*1.069583140309415e-6;
et399 = t5.*t7.*3.581728501918121e-6;
et400 = t7.*t9.*(-6.589841321991422e-6)-t3.*t18.*1.253488085959302e-6+t8.*t436;
et401 = t3.*t4.*t8.*(-5.073437414621283e-7)+t3.*t5.*t8.*6.589841321991422e-6;
et402 = t3.*t8.*t9.*3.581728501918121e-6-t5.*t7.*t8.*2.7046541903611e-13;
C_dq = ft_16({dq1,dq2,dq3,dq4,dq5,dq6,et294,et295,et296,et341,et342,et343,et352,et353,et354,et355,et356,et359,et360,et361,et371,et372,et373,et374,et375,et376,et377,et378,et379,et380,et381,et382,et383,et384,et385,et386,et387,et388,et389,et390,et391,et392,et393,et394,et395,et396,et397,et398,et399,et400,et401,et402,t1004,t1016,t1019,t1031,t1039,t1050,t1056,t1061,t1069,t1075,t1077,t1081,t1083,t1088,t1090,t1095,t1099,t1101,t1106,t1108,t112,t1122,t113,t1133,t1144,t1147,t115,t1150,t1152,t1155,t1156,t1158,t116,t1170,t1171,t1174,t1177,t1179,t1184,t1185,t1191,t1193,t1194,t1196,t1201,t1203,t1205,t1207,t121,t1212,t1213,t1215,t1221,t1224,t1225,t1227,t1233,t1245,t125,t1250,t1253,t1254,t1258,t1273,t1274,t1282,t1285,t1288,t1292,t1300,t1301,t1306,t131,t1316,t132,t1322,t1323,t1324,t133,t1330,t1331,t1333,t1337,t1342,t1344,t1345,t1348,t1353,t1365,t1377,t1379,t1380,t1383,t1388,t1391,t1402,t1407,t1409,t1411,t1413,t1419,t1423,t1426,t1427,t1428,t1429,t1436,t144,t1440,t1441,t1443,t1445,t1449,t1454,t1457,t1458,t1460,t1471,t148,t1486,t1487,t1489,t1493,t1494,t1495,t1496,t15,t150,t1503,t1508,t1523,t1530,t1531,t1537,t1540,t1541,t1542,t1548,t1550,t1551,t156,t1568,t1570,t1578,t158,t1587,t1593,t16,t1601,t1607,t1609,t1612,t1615,t1616,t1621,t1622,t1627,t1642,t1648,t1656,t1659,t166,t1661,t1670,t1672,t1674,t1681,t1687,t1692,t17,t1704,t171,t1710,t1715,t1719,t1721,t1731,t1732,t1734,t1740,t1747,t1753,t1758,t1759,t1767,t1769,t1770,t1771,t1772,t1775,t1776,t1777,t1781,t1783,t1784,t1792,t1793,t1794,t1795,t1798,t18,t1805,t1806,t1808,t1811,t1812,t1814,t1816,t1820,t1823,t1827,t1828,t183,t1831,t1833,t1834,t1835,t1847,t185,t1855,t1858,t1870,t1873,t19,t190,t1902,t1908,t191,t1922,t1930,t1938,t1947,t1952,t196,t1968,t197,t1977,t1981,t1983,t1984,t1985,t1986,t199,t1992,t1993,t1995,t1997,t2,t20,t200,t2002,t2004,t201,t2014,t2017,t202,t2028,t2034,t2035,t2038,t2043,t2052,t2062,t2068,t2069,t2075,t2083,t2088,t2096,t21,t2113,t2115,t2121,t2123,t2130,t2132,t2133,t2143,t2150,t2154,t2158,t2164,t2165,t2177,t2178,t2180,t2181,t2184,t2186,t2187,t2192,t2193,t2196,t22,t2200,t2202,t2203,t2211,t2213,t2214,t2236,t2266,t2267,t2289,t2291,t23,t2303,t231,t2312,t2314,t2315,t2320,t2333,t2334,t2338,t2341,t235,t236,t2383,t2390,t2392,t2395,t2397,t2398,t24,t240,t2420,t2421,t2424,t2444,t2449,t2465,t2466,t2474,t2481,t2486,t2524,t2525,t2530,t2539,t2546,t2554,t2556,t2560,t257,t258,t2627,t263,t275,t277,t278,t2795,t2797,t284,t2868,t287,t2881,t29,t290,t3,t30,t300,t302,t305,t309,t310,t311,t3136,t314,t3142,t315,t318,t319,t3219,t322,t3230,t3274,t3321,t3338,t336,t3365,t3375,t3378,t3383,t3390,t3391,t3392,t3397,t34,t3400,t3407,t3409,t3416,t3417,t3420,t3422,t3426,t3429,t3430,t3432,t3435,t3436,t3437,t3439,t3440,t3443,t3444,t3446,t3449,t3450,t3457,t3458,t3463,t3464,t3465,t3468,t3469,t3474,t3475,t3476,t3479,t3483,t3485,t3489,t349,t3490,t3491,t3492,t3496,t3498,t3499,t3501,t3504,t3507,t3510,t3513,t3514,t3515,t3521,t3522,t3523,t3526,t3530,t3531,t3532,t3535,t3540,t3542,t3543,t3547,t3554,t3556,t356,t3569,t357,t3571,t3574,t3577,t3578,t358,t3582,t3583,t3584,t3585,t3592,t3605,t3606,t3607,t361,t3610,t3612,t3618,t3635,t3637,t3658,t3659,t3662,t3666,t3667,t3694,t3706,t371,t3719,t372,t3726,t373,t3732,t3734,t3738,t374,t3753,t3755,t3757,t3761,t3763,t377,t3772,t3783,t3788,t379,t3792,t3819,t3822,t3831,t3843,t3852,t3863,t3869,t3871,t3873,t3874,t3875,t3891,t391,t3922,t395,t3951,t3956,t3957,t3960,t3968,t3978,t3979,t3992,t3993,t4,t4004,t4011,t4015,t402,t403,t406,t4089,t4099,t410,t4100,t4103,t4108,t411,t4115,t4119,t4123,t4126,t413,t4132,t4134,t414,t4143,t4148,t4152,t4153,t4158,t4166,t4173,t4178,t4179,t418,t4181,t4183,t4185,t4190,t4208,t422,t4221,t4228,t423,t4230,t4232,t424,t4249,t425,t4254,t4255,t4259,t427,t4278,t4279,t428,t4286,t429,t4304,t431,t4317,t432,t4327,t433,t4337,t434,t4342,t4344,t4345,t4347,t4348,t4349,t435,t436,t4369,t4370,t4378,t4382,t4388,t4392,t4394,t4395,t4396,t4397,t440,t4402,t4403,t4405,t4406,t441,t4410,t4412,t4413,t4416,t4417,t4419,t442,t4420,t4423,t4425,t4426,t4428,t4429,t4431,t4436,t444,t4440,t4444,t4447,t445,t4462,t4469,t4473,t4478,t448,t4482,t4485,t4486,t4488,t449,t4490,t4495,t4498,t4501,t4502,t4506,t4509,t4518,t4519,t452,t4520,t4522,t4523,t4527,t4528,t453,t4530,t454,t4541,t4543,t4545,t4549,t4551,t4553,t4556,t4557,t4558,t4559,t4568,t457,t4572,t4575,t458,t4581,t4586,t4587,t4588,t4589,t459,t4590,t4591,t4592,t4596,t460,t4600,t4601,t4605,t4606,t4607,t4614,t4616,t4619,t4621,t4622,t4625,t4626,t463,t4633,t4634,t4636,t4648,t4656,t4660,t4666,t4667,t4669,t4674,t4675,t468,t469,t4694,t4695,t4697,t470,t4707,t4708,t4724,t4727,t4728,t4731,t4732,t4733,t4737,t4739,t4742,t4743,t4745,t4747,t475,t4755,t4756,t477,t4780,t4782,t4783,t4785,t4786,t479,t480,t481,t4810,t482,t483,t4838,t485,t486,t488,t489,t4904,t491,t4919,t492,t493,t494,t496,t4983,t4984,t5,t50,t508,t510,t512,t513,t514,t516,t517,t518,t520,t521,t522,t5228,t523,t524,t525,t5259,t5275,t529,t53,t531,t5316,t532,t5323,t533,t534,t535,t5354,t539,t540,t543,t545,t547,t548,t549,t553,t559,t5602,t5605,t561,t5621,t563,t5633,t5634,t5636,t564,t5657,t5658,t5662,t5665,t5666,t567,t5670,t5676,t5679,t568,t5683,t5684,t5688,t5691,t5699,t5702,t5704,t5709,t5718,t5730,t5738,t5742,t5744,t5757,t5769,t5770,t5772,t5775,t5776,t5778,t578,t5784,t5786,t5787,t5790,t5791,t5792,t5794,t5795,t5797,t580,t5808,t581,t5810,t582,t5822,t5823,t5824,t5825,t5826,t5831,t5838,t584,t5841,t5842,t5844,t5845,t5846,t5847,t5849,t5850,t5851,t5852,t586,t5861,t587,t5872,t5878,t5881,t5882,t5883,t5888,t5889,t589,t5892,t5894,t5895,t5897,t5898,t5899,t590,t5905,t5915,t5916,t5918,t592,t5921,t5922,t5925,t5926,t5928,t5930,t5934,t5937,t5938,t5939,t594,t5940,t5942,t5943,t5944,t5947,t5950,t5951,t5952,t5954,t5958,t596,t5960,t5961,t5967,t5968,t597,t5973,t5974,t5977,t5978,t5979,t5982,t5984,t5985,t5986,t5988,t5996,t6,t600,t6005,t6008,t6009,t6013,t6017,t6019,t602,t6026,t603,t6035,t6037,t604,t6042,t6044,t6046,t6047,t6048,t605,t6053,t6056,t6060,t6074,t6081,t609,t6095,t610,t6103,t6108,t6109,t611,t6118,t6119,t612,t6123,t6125,t6127,t613,t6136,t614,t6142,t6145,t6146,t6147,t615,t6152,t6155,t6158,t616,t6162,t6164,t6165,t6167,t6170,t6171,t6175,t6177,t6179,t618,t6182,t6183,t6189,t619,t6191,t6194,t6195,t6196,t6197,t620,t6202,t6203,t6209,t621,t6210,t6213,t6215,t6216,t6218,t622,t6220,t6222,t6225,t6226,t623,t6230,t6231,t6232,t6235,t6239,t624,t6244,t6248,t6249,t625,t6252,t6255,t6271,t6272,t6274,t6276,t6280,t6282,t6289,t6293,t6294,t6296,t6303,t6307,t6312,t6313,t632,t6322,t6329,t6330,t6332,t6345,t6349,t6350,t6351,t6352,t6359,t6360,t6362,t638,t6380,t6382,t6385,t6386,t6391,t6393,t6395,t6396,t6397,t6399,t640,t6400,t6401,t6402,t6405,t6406,t6407,t6412,t6414,t6422,t6426,t6431,t6433,t6434,t6442,t6443,t6445,t6449,t6451,t6454,t6462,t6463,t6465,t6468,t6470,t6473,t6477,t6486,t6487,t6489,t6503,t6504,t6513,t6521,t6536,t6537,t6544,t6546,t6548,t6551,t6557,t6560,t6561,t6562,t6563,t6564,t6571,t6574,t6580,t6593,t6594,t6604,t6605,t6607,t6610,t6648,t6656,t6664,t6669,t6672,t6676,t6677,t6694,t6695,t6699,t6711,t6714,t6715,t6721,t6724,t6727,t6729,t6738,t6743,t6746,t6747,t6753,t6756,t6758,t6774,t6776,t6783,t6807,t681,t6818,t6821,t6831,t6832,t6838,t684,t6841,t6842,t6844,t6847,t6849,t6851,t6856,t6859,t6860,t6865,t6879,t6884,t6888,t6890,t6891,t6892,t6894,t6898,t6903,t6909,t6911,t6914,t6915,t6916,t6918,t6919,t6921,t6922,t6924,t6926,t6927,t6928,t6930,t6935,t6936,t6937,t6939,t6941,t6944,t6946,t6952,t6953,t6954,t6960,t6975,t6977,t6983,t6984,t6985,t6986,t6989,t6990,t6991,t6994,t7,t7000,t7003,t7006,t7008,t7010,t7011,t7012,t7022,t7023,t7026,t7027,t7030,t7031,t7032,t7033,t7035,t7036,t7039,t7040,t7042,t7044,t7045,t7048,t7051,t7052,t7053,t7054,t7055,t7059,t7060,t7061,t7066,t7067,t7069,t7071,t7072,t7074,t7075,t7076,t7077,t7078,t7081,t7082,t7084,t7085,t7086,t7087,t7088,t7089,t7091,t7093,t7095,t7096,t7098,t7100,t7102,t7103,t7104,t7110,t7113,t7114,t7115,t712,t7120,t7122,t7123,t7124,t7127,t7128,t7129,t7130,t7133,t7134,t7136,t7137,t7140,t7141,t7142,t7143,t7148,t7149,t7156,t7158,t7168,t7170,t7174,t7176,t7191,t7192,t7194,t72,t7201,t7203,t7204,t7206,t7207,t7208,t7215,t7217,t7221,t7222,t7223,t7224,t7226,t7231,t7234,t7235,t7237,t724,t7242,t7243,t7244,t7245,t7246,t7247,t7248,t7254,t7255,t7256,t7257,t7258,t7261,t7263,t7267,t7268,t7269,t7270,t7271,t7272,t7273,t7274,t7276,t7277,t7279,t7281,t7284,t7288,t7289,t7296,t7297,t73,t7300,t7304,t7305,t7307,t7308,t7309,t7310,t7312,t7319,t7321,t7322,t7324,t7327,t7331,t7332,t7336,t7337,t7339,t7340,t7341,t7342,t7343,t7344,t7346,t7348,t7349,t7350,t7362,t7363,t7366,t7367,t7368,t7369,t7371,t7372,t7373,t7374,t7375,t7376,t7377,t7378,t7379,t738,t7380,t7381,t7382,t7383,t7384,t7385,t7386,t7387,t7388,t7390,t7391,t7392,t7393,t7394,t7395,t7396,t7398,t7399,t7402,t7403,t7405,t741,t7410,t7413,t7414,t742,t7421,t7423,t7425,t7426,t7427,t7428,t7429,t7430,t7431,t7433,t7434,t7435,t7437,t7439,t7440,t7442,t7444,t7446,t7447,t7448,t7450,t7453,t7455,t7458,t7459,t7461,t7463,t7465,t7468,t7469,t7470,t7476,t7477,t7479,t7480,t7481,t7482,t7483,t7485,t7486,t7487,t7488,t7490,t7491,t7492,t7493,t7494,t7495,t7496,t7498,t7499,t7500,t7501,t7502,t7503,t7504,t7507,t7508,t7509,t7510,t7511,t7512,t7513,t7515,t7516,t7517,t7519,t7521,t7522,t7523,t7524,t7525,t7526,t7527,t7529,t753,t7530,t7531,t7533,t7534,t7536,t7537,t7538,t7541,t7542,t7543,t7546,t7548,t7549,t7550,t7552,t7554,t7555,t7557,t7558,t7562,t7563,t7565,t7567,t7568,t7571,t7572,t7574,t7577,t7580,t7584,t7587,t7593,t7595,t7596,t7597,t7599,t760,t781,t792,t797,t8,t803,t81,t825,t826,t827,t832,t845,t848,t852,t86,t866,t868,t869,t874,t875,t877,t881,t893,t899,t9,t90,t902,t903,t908,t91,t910,t911,t912,t915,t917,t919,t922,t926,t928,t930,t931,t932,t934,t940,t944,t947,t95,t952,t957,t958,t968,t970,t971,t972,t975,t976,t984,t985,t986,t989,t99,t991,t998});
end
function C_dq = ft_16(ct)
dq1 = ct{1};
dq2 = ct{2};
dq3 = ct{3};
dq4 = ct{4};
dq5 = ct{5};
dq6 = ct{6};
et294 = ct{7};
et295 = ct{8};
et296 = ct{9};
et341 = ct{10};
et342 = ct{11};
et343 = ct{12};
et352 = ct{13};
et353 = ct{14};
et354 = ct{15};
et355 = ct{16};
et356 = ct{17};
et359 = ct{18};
et360 = ct{19};
et361 = ct{20};
et371 = ct{21};
et372 = ct{22};
et373 = ct{23};
et374 = ct{24};
et375 = ct{25};
et376 = ct{26};
et377 = ct{27};
et378 = ct{28};
et379 = ct{29};
et380 = ct{30};
et381 = ct{31};
et382 = ct{32};
et383 = ct{33};
et384 = ct{34};
et385 = ct{35};
et386 = ct{36};
et387 = ct{37};
et388 = ct{38};
et389 = ct{39};
et390 = ct{40};
et391 = ct{41};
et392 = ct{42};
et393 = ct{43};
et394 = ct{44};
et395 = ct{45};
et396 = ct{46};
et397 = ct{47};
et398 = ct{48};
et399 = ct{49};
et400 = ct{50};
et401 = ct{51};
et402 = ct{52};
t1004 = ct{53};
t1016 = ct{54};
t1019 = ct{55};
t1031 = ct{56};
t1039 = ct{57};
t1050 = ct{58};
t1056 = ct{59};
t1061 = ct{60};
t1069 = ct{61};
t1075 = ct{62};
t1077 = ct{63};
t1081 = ct{64};
t1083 = ct{65};
t1088 = ct{66};
t1090 = ct{67};
t1095 = ct{68};
t1099 = ct{69};
t1101 = ct{70};
t1106 = ct{71};
t1108 = ct{72};
t112 = ct{73};
t1122 = ct{74};
t113 = ct{75};
t1133 = ct{76};
t1144 = ct{77};
t1147 = ct{78};
t115 = ct{79};
t1150 = ct{80};
t1152 = ct{81};
t1155 = ct{82};
t1156 = ct{83};
t1158 = ct{84};
t116 = ct{85};
t1170 = ct{86};
t1171 = ct{87};
t1174 = ct{88};
t1177 = ct{89};
t1179 = ct{90};
t1184 = ct{91};
t1185 = ct{92};
t1191 = ct{93};
t1193 = ct{94};
t1194 = ct{95};
t1196 = ct{96};
t1201 = ct{97};
t1203 = ct{98};
t1205 = ct{99};
t1207 = ct{100};
t121 = ct{101};
t1212 = ct{102};
t1213 = ct{103};
t1215 = ct{104};
t1221 = ct{105};
t1224 = ct{106};
t1225 = ct{107};
t1227 = ct{108};
t1233 = ct{109};
t1245 = ct{110};
t125 = ct{111};
t1250 = ct{112};
t1253 = ct{113};
t1254 = ct{114};
t1258 = ct{115};
t1273 = ct{116};
t1274 = ct{117};
t1282 = ct{118};
t1285 = ct{119};
t1288 = ct{120};
t1292 = ct{121};
t1300 = ct{122};
t1301 = ct{123};
t1306 = ct{124};
t131 = ct{125};
t1316 = ct{126};
t132 = ct{127};
t1322 = ct{128};
t1323 = ct{129};
t1324 = ct{130};
t133 = ct{131};
t1330 = ct{132};
t1331 = ct{133};
t1333 = ct{134};
t1337 = ct{135};
t1342 = ct{136};
t1344 = ct{137};
t1345 = ct{138};
t1348 = ct{139};
t1353 = ct{140};
t1365 = ct{141};
t1377 = ct{142};
t1379 = ct{143};
t1380 = ct{144};
t1383 = ct{145};
t1388 = ct{146};
t1391 = ct{147};
t1402 = ct{148};
t1407 = ct{149};
t1409 = ct{150};
t1411 = ct{151};
t1413 = ct{152};
t1419 = ct{153};
t1423 = ct{154};
t1426 = ct{155};
t1427 = ct{156};
t1428 = ct{157};
t1429 = ct{158};
t1436 = ct{159};
t144 = ct{160};
t1440 = ct{161};
t1441 = ct{162};
t1443 = ct{163};
t1445 = ct{164};
t1449 = ct{165};
t1454 = ct{166};
t1457 = ct{167};
t1458 = ct{168};
t1460 = ct{169};
t1471 = ct{170};
t148 = ct{171};
t1486 = ct{172};
t1487 = ct{173};
t1489 = ct{174};
t1493 = ct{175};
t1494 = ct{176};
t1495 = ct{177};
t1496 = ct{178};
t15 = ct{179};
t150 = ct{180};
t1503 = ct{181};
t1508 = ct{182};
t1523 = ct{183};
t1530 = ct{184};
t1531 = ct{185};
t1537 = ct{186};
t1540 = ct{187};
t1541 = ct{188};
t1542 = ct{189};
t1548 = ct{190};
t1550 = ct{191};
t1551 = ct{192};
t156 = ct{193};
t1568 = ct{194};
t1570 = ct{195};
t1578 = ct{196};
t158 = ct{197};
t1587 = ct{198};
t1593 = ct{199};
t16 = ct{200};
t1601 = ct{201};
t1607 = ct{202};
t1609 = ct{203};
t1612 = ct{204};
t1615 = ct{205};
t1616 = ct{206};
t1621 = ct{207};
t1622 = ct{208};
t1627 = ct{209};
t1642 = ct{210};
t1648 = ct{211};
t1656 = ct{212};
t1659 = ct{213};
t166 = ct{214};
t1661 = ct{215};
t1670 = ct{216};
t1672 = ct{217};
t1674 = ct{218};
t1681 = ct{219};
t1687 = ct{220};
t1692 = ct{221};
t17 = ct{222};
t1704 = ct{223};
t171 = ct{224};
t1710 = ct{225};
t1715 = ct{226};
t1719 = ct{227};
t1721 = ct{228};
t1731 = ct{229};
t1732 = ct{230};
t1734 = ct{231};
t1740 = ct{232};
t1747 = ct{233};
t1753 = ct{234};
t1758 = ct{235};
t1759 = ct{236};
t1767 = ct{237};
t1769 = ct{238};
t1770 = ct{239};
t1771 = ct{240};
t1772 = ct{241};
t1775 = ct{242};
t1776 = ct{243};
t1777 = ct{244};
t1781 = ct{245};
t1783 = ct{246};
t1784 = ct{247};
t1792 = ct{248};
t1793 = ct{249};
t1794 = ct{250};
t1795 = ct{251};
t1798 = ct{252};
t18 = ct{253};
t1805 = ct{254};
t1806 = ct{255};
t1808 = ct{256};
t1811 = ct{257};
t1812 = ct{258};
t1814 = ct{259};
t1816 = ct{260};
t1820 = ct{261};
t1823 = ct{262};
t1827 = ct{263};
t1828 = ct{264};
t183 = ct{265};
t1831 = ct{266};
t1833 = ct{267};
t1834 = ct{268};
t1835 = ct{269};
t1847 = ct{270};
t185 = ct{271};
t1855 = ct{272};
t1858 = ct{273};
t1870 = ct{274};
t1873 = ct{275};
t19 = ct{276};
t190 = ct{277};
t1902 = ct{278};
t1908 = ct{279};
t191 = ct{280};
t1922 = ct{281};
t1930 = ct{282};
t1938 = ct{283};
t1947 = ct{284};
t1952 = ct{285};
t196 = ct{286};
t1968 = ct{287};
t197 = ct{288};
t1977 = ct{289};
t1981 = ct{290};
t1983 = ct{291};
t1984 = ct{292};
t1985 = ct{293};
t1986 = ct{294};
t199 = ct{295};
t1992 = ct{296};
t1993 = ct{297};
t1995 = ct{298};
t1997 = ct{299};
t2 = ct{300};
t20 = ct{301};
t200 = ct{302};
t2002 = ct{303};
t2004 = ct{304};
t201 = ct{305};
t2014 = ct{306};
t2017 = ct{307};
t202 = ct{308};
t2028 = ct{309};
t2034 = ct{310};
t2035 = ct{311};
t2038 = ct{312};
t2043 = ct{313};
t2052 = ct{314};
t2062 = ct{315};
t2068 = ct{316};
t2069 = ct{317};
t2075 = ct{318};
t2083 = ct{319};
t2088 = ct{320};
t2096 = ct{321};
t21 = ct{322};
t2113 = ct{323};
t2115 = ct{324};
t2121 = ct{325};
t2123 = ct{326};
t2130 = ct{327};
t2132 = ct{328};
t2133 = ct{329};
t2143 = ct{330};
t2150 = ct{331};
t2154 = ct{332};
t2158 = ct{333};
t2164 = ct{334};
t2165 = ct{335};
t2177 = ct{336};
t2178 = ct{337};
t2180 = ct{338};
t2181 = ct{339};
t2184 = ct{340};
t2186 = ct{341};
t2187 = ct{342};
t2192 = ct{343};
t2193 = ct{344};
t2196 = ct{345};
t22 = ct{346};
t2200 = ct{347};
t2202 = ct{348};
t2203 = ct{349};
t2211 = ct{350};
t2213 = ct{351};
t2214 = ct{352};
t2236 = ct{353};
t2266 = ct{354};
t2267 = ct{355};
t2289 = ct{356};
t2291 = ct{357};
t23 = ct{358};
t2303 = ct{359};
t231 = ct{360};
t2312 = ct{361};
t2314 = ct{362};
t2315 = ct{363};
t2320 = ct{364};
t2333 = ct{365};
t2334 = ct{366};
t2338 = ct{367};
t2341 = ct{368};
t235 = ct{369};
t236 = ct{370};
t2383 = ct{371};
t2390 = ct{372};
t2392 = ct{373};
t2395 = ct{374};
t2397 = ct{375};
t2398 = ct{376};
t24 = ct{377};
t240 = ct{378};
t2420 = ct{379};
t2421 = ct{380};
t2424 = ct{381};
t2444 = ct{382};
t2449 = ct{383};
t2465 = ct{384};
t2466 = ct{385};
t2474 = ct{386};
t2481 = ct{387};
t2486 = ct{388};
t2524 = ct{389};
t2525 = ct{390};
t2530 = ct{391};
t2539 = ct{392};
t2546 = ct{393};
t2554 = ct{394};
t2556 = ct{395};
t2560 = ct{396};
t257 = ct{397};
t258 = ct{398};
t2627 = ct{399};
t263 = ct{400};
t275 = ct{401};
t277 = ct{402};
t278 = ct{403};
t2795 = ct{404};
t2797 = ct{405};
t284 = ct{406};
t2868 = ct{407};
t287 = ct{408};
t2881 = ct{409};
t29 = ct{410};
t290 = ct{411};
t3 = ct{412};
t30 = ct{413};
t300 = ct{414};
t302 = ct{415};
t305 = ct{416};
t309 = ct{417};
t310 = ct{418};
t311 = ct{419};
t3136 = ct{420};
t314 = ct{421};
t3142 = ct{422};
t315 = ct{423};
t318 = ct{424};
t319 = ct{425};
t3219 = ct{426};
t322 = ct{427};
t3230 = ct{428};
t3274 = ct{429};
t3321 = ct{430};
t3338 = ct{431};
t336 = ct{432};
t3365 = ct{433};
t3375 = ct{434};
t3378 = ct{435};
t3383 = ct{436};
t3390 = ct{437};
t3391 = ct{438};
t3392 = ct{439};
t3397 = ct{440};
t34 = ct{441};
t3400 = ct{442};
t3407 = ct{443};
t3409 = ct{444};
t3416 = ct{445};
t3417 = ct{446};
t3420 = ct{447};
t3422 = ct{448};
t3426 = ct{449};
t3429 = ct{450};
t3430 = ct{451};
t3432 = ct{452};
t3435 = ct{453};
t3436 = ct{454};
t3437 = ct{455};
t3439 = ct{456};
t3440 = ct{457};
t3443 = ct{458};
t3444 = ct{459};
t3446 = ct{460};
t3449 = ct{461};
t3450 = ct{462};
t3457 = ct{463};
t3458 = ct{464};
t3463 = ct{465};
t3464 = ct{466};
t3465 = ct{467};
t3468 = ct{468};
t3469 = ct{469};
t3474 = ct{470};
t3475 = ct{471};
t3476 = ct{472};
t3479 = ct{473};
t3483 = ct{474};
t3485 = ct{475};
t3489 = ct{476};
t349 = ct{477};
t3490 = ct{478};
t3491 = ct{479};
t3492 = ct{480};
t3496 = ct{481};
t3498 = ct{482};
t3499 = ct{483};
t3501 = ct{484};
t3504 = ct{485};
t3507 = ct{486};
t3510 = ct{487};
t3513 = ct{488};
t3514 = ct{489};
t3515 = ct{490};
t3521 = ct{491};
t3522 = ct{492};
t3523 = ct{493};
t3526 = ct{494};
t3530 = ct{495};
t3531 = ct{496};
t3532 = ct{497};
t3535 = ct{498};
t3540 = ct{499};
t3542 = ct{500};
t3543 = ct{501};
t3547 = ct{502};
t3554 = ct{503};
t3556 = ct{504};
t356 = ct{505};
t3569 = ct{506};
t357 = ct{507};
t3571 = ct{508};
t3574 = ct{509};
t3577 = ct{510};
t3578 = ct{511};
t358 = ct{512};
t3582 = ct{513};
t3583 = ct{514};
t3584 = ct{515};
t3585 = ct{516};
t3592 = ct{517};
t3605 = ct{518};
t3606 = ct{519};
t3607 = ct{520};
t361 = ct{521};
t3610 = ct{522};
t3612 = ct{523};
t3618 = ct{524};
t3635 = ct{525};
t3637 = ct{526};
t3658 = ct{527};
t3659 = ct{528};
t3662 = ct{529};
t3666 = ct{530};
t3667 = ct{531};
t3694 = ct{532};
t3706 = ct{533};
t371 = ct{534};
t3719 = ct{535};
t372 = ct{536};
t3726 = ct{537};
t373 = ct{538};
t3732 = ct{539};
t3734 = ct{540};
t3738 = ct{541};
t374 = ct{542};
t3753 = ct{543};
t3755 = ct{544};
t3757 = ct{545};
t3761 = ct{546};
t3763 = ct{547};
t377 = ct{548};
t3772 = ct{549};
t3783 = ct{550};
t3788 = ct{551};
t379 = ct{552};
t3792 = ct{553};
t3819 = ct{554};
t3822 = ct{555};
t3831 = ct{556};
t3843 = ct{557};
t3852 = ct{558};
t3863 = ct{559};
t3869 = ct{560};
t3871 = ct{561};
t3873 = ct{562};
t3874 = ct{563};
t3875 = ct{564};
t3891 = ct{565};
t391 = ct{566};
t3922 = ct{567};
t395 = ct{568};
t3951 = ct{569};
t3956 = ct{570};
t3957 = ct{571};
t3960 = ct{572};
t3968 = ct{573};
t3978 = ct{574};
t3979 = ct{575};
t3992 = ct{576};
t3993 = ct{577};
t4 = ct{578};
t4004 = ct{579};
t4011 = ct{580};
t4015 = ct{581};
t402 = ct{582};
t403 = ct{583};
t406 = ct{584};
t4089 = ct{585};
t4099 = ct{586};
t410 = ct{587};
t4100 = ct{588};
t4103 = ct{589};
t4108 = ct{590};
t411 = ct{591};
t4115 = ct{592};
t4119 = ct{593};
t4123 = ct{594};
t4126 = ct{595};
t413 = ct{596};
t4132 = ct{597};
t4134 = ct{598};
t414 = ct{599};
t4143 = ct{600};
t4148 = ct{601};
t4152 = ct{602};
t4153 = ct{603};
t4158 = ct{604};
t4166 = ct{605};
t4173 = ct{606};
t4178 = ct{607};
t4179 = ct{608};
t418 = ct{609};
t4181 = ct{610};
t4183 = ct{611};
t4185 = ct{612};
t4190 = ct{613};
t4208 = ct{614};
t422 = ct{615};
t4221 = ct{616};
t4228 = ct{617};
t423 = ct{618};
t4230 = ct{619};
t4232 = ct{620};
t424 = ct{621};
t4249 = ct{622};
t425 = ct{623};
t4254 = ct{624};
t4255 = ct{625};
t4259 = ct{626};
t427 = ct{627};
t4278 = ct{628};
t4279 = ct{629};
t428 = ct{630};
t4286 = ct{631};
t429 = ct{632};
t4304 = ct{633};
t431 = ct{634};
t4317 = ct{635};
t432 = ct{636};
t4327 = ct{637};
t433 = ct{638};
t4337 = ct{639};
t434 = ct{640};
t4342 = ct{641};
t4344 = ct{642};
t4345 = ct{643};
t4347 = ct{644};
t4348 = ct{645};
t4349 = ct{646};
t435 = ct{647};
t436 = ct{648};
t4369 = ct{649};
t4370 = ct{650};
t4378 = ct{651};
t4382 = ct{652};
t4388 = ct{653};
t4392 = ct{654};
t4394 = ct{655};
t4395 = ct{656};
t4396 = ct{657};
t4397 = ct{658};
t440 = ct{659};
t4402 = ct{660};
t4403 = ct{661};
t4405 = ct{662};
t4406 = ct{663};
t441 = ct{664};
t4410 = ct{665};
t4412 = ct{666};
t4413 = ct{667};
t4416 = ct{668};
t4417 = ct{669};
t4419 = ct{670};
t442 = ct{671};
t4420 = ct{672};
t4423 = ct{673};
t4425 = ct{674};
t4426 = ct{675};
t4428 = ct{676};
t4429 = ct{677};
t4431 = ct{678};
t4436 = ct{679};
t444 = ct{680};
t4440 = ct{681};
t4444 = ct{682};
t4447 = ct{683};
t445 = ct{684};
t4462 = ct{685};
t4469 = ct{686};
t4473 = ct{687};
t4478 = ct{688};
t448 = ct{689};
t4482 = ct{690};
t4485 = ct{691};
t4486 = ct{692};
t4488 = ct{693};
t449 = ct{694};
t4490 = ct{695};
t4495 = ct{696};
t4498 = ct{697};
t4501 = ct{698};
t4502 = ct{699};
t4506 = ct{700};
t4509 = ct{701};
t4518 = ct{702};
t4519 = ct{703};
t452 = ct{704};
t4520 = ct{705};
t4522 = ct{706};
t4523 = ct{707};
t4527 = ct{708};
t4528 = ct{709};
t453 = ct{710};
t4530 = ct{711};
t454 = ct{712};
t4541 = ct{713};
t4543 = ct{714};
t4545 = ct{715};
t4549 = ct{716};
t4551 = ct{717};
t4553 = ct{718};
t4556 = ct{719};
t4557 = ct{720};
t4558 = ct{721};
t4559 = ct{722};
t4568 = ct{723};
t457 = ct{724};
t4572 = ct{725};
t4575 = ct{726};
t458 = ct{727};
t4581 = ct{728};
t4586 = ct{729};
t4587 = ct{730};
t4588 = ct{731};
t4589 = ct{732};
t459 = ct{733};
t4590 = ct{734};
t4591 = ct{735};
t4592 = ct{736};
t4596 = ct{737};
t460 = ct{738};
t4600 = ct{739};
t4601 = ct{740};
t4605 = ct{741};
t4606 = ct{742};
t4607 = ct{743};
t4614 = ct{744};
t4616 = ct{745};
t4619 = ct{746};
t4621 = ct{747};
t4622 = ct{748};
t4625 = ct{749};
t4626 = ct{750};
t463 = ct{751};
t4633 = ct{752};
t4634 = ct{753};
t4636 = ct{754};
t4648 = ct{755};
t4656 = ct{756};
t4660 = ct{757};
t4666 = ct{758};
t4667 = ct{759};
t4669 = ct{760};
t4674 = ct{761};
t4675 = ct{762};
t468 = ct{763};
t469 = ct{764};
t4694 = ct{765};
t4695 = ct{766};
t4697 = ct{767};
t470 = ct{768};
t4707 = ct{769};
t4708 = ct{770};
t4724 = ct{771};
t4727 = ct{772};
t4728 = ct{773};
t4731 = ct{774};
t4732 = ct{775};
t4733 = ct{776};
t4737 = ct{777};
t4739 = ct{778};
t4742 = ct{779};
t4743 = ct{780};
t4745 = ct{781};
t4747 = ct{782};
t475 = ct{783};
t4755 = ct{784};
t4756 = ct{785};
t477 = ct{786};
t4780 = ct{787};
t4782 = ct{788};
t4783 = ct{789};
t4785 = ct{790};
t4786 = ct{791};
t479 = ct{792};
t480 = ct{793};
t481 = ct{794};
t4810 = ct{795};
t482 = ct{796};
t483 = ct{797};
t4838 = ct{798};
t485 = ct{799};
t486 = ct{800};
t488 = ct{801};
t489 = ct{802};
t4904 = ct{803};
t491 = ct{804};
t4919 = ct{805};
t492 = ct{806};
t493 = ct{807};
t494 = ct{808};
t496 = ct{809};
t4983 = ct{810};
t4984 = ct{811};
t5 = ct{812};
t50 = ct{813};
t508 = ct{814};
t510 = ct{815};
t512 = ct{816};
t513 = ct{817};
t514 = ct{818};
t516 = ct{819};
t517 = ct{820};
t518 = ct{821};
t520 = ct{822};
t521 = ct{823};
t522 = ct{824};
t5228 = ct{825};
t523 = ct{826};
t524 = ct{827};
t525 = ct{828};
t5259 = ct{829};
t5275 = ct{830};
t529 = ct{831};
t53 = ct{832};
t531 = ct{833};
t5316 = ct{834};
t532 = ct{835};
t5323 = ct{836};
t533 = ct{837};
t534 = ct{838};
t535 = ct{839};
t5354 = ct{840};
t539 = ct{841};
t540 = ct{842};
t543 = ct{843};
t545 = ct{844};
t547 = ct{845};
t548 = ct{846};
t549 = ct{847};
t553 = ct{848};
t559 = ct{849};
t5602 = ct{850};
t5605 = ct{851};
t561 = ct{852};
t5621 = ct{853};
t563 = ct{854};
t5633 = ct{855};
t5634 = ct{856};
t5636 = ct{857};
t564 = ct{858};
t5657 = ct{859};
t5658 = ct{860};
t5662 = ct{861};
t5665 = ct{862};
t5666 = ct{863};
t567 = ct{864};
t5670 = ct{865};
t5676 = ct{866};
t5679 = ct{867};
t568 = ct{868};
t5683 = ct{869};
t5684 = ct{870};
t5688 = ct{871};
t5691 = ct{872};
t5699 = ct{873};
t5702 = ct{874};
t5704 = ct{875};
t5709 = ct{876};
t5718 = ct{877};
t5730 = ct{878};
t5738 = ct{879};
t5742 = ct{880};
t5744 = ct{881};
t5757 = ct{882};
t5769 = ct{883};
t5770 = ct{884};
t5772 = ct{885};
t5775 = ct{886};
t5776 = ct{887};
t5778 = ct{888};
t578 = ct{889};
t5784 = ct{890};
t5786 = ct{891};
t5787 = ct{892};
t5790 = ct{893};
t5791 = ct{894};
t5792 = ct{895};
t5794 = ct{896};
t5795 = ct{897};
t5797 = ct{898};
t580 = ct{899};
t5808 = ct{900};
t581 = ct{901};
t5810 = ct{902};
t582 = ct{903};
t5822 = ct{904};
t5823 = ct{905};
t5824 = ct{906};
t5825 = ct{907};
t5826 = ct{908};
t5831 = ct{909};
t5838 = ct{910};
t584 = ct{911};
t5841 = ct{912};
t5842 = ct{913};
t5844 = ct{914};
t5845 = ct{915};
t5846 = ct{916};
t5847 = ct{917};
t5849 = ct{918};
t5850 = ct{919};
t5851 = ct{920};
t5852 = ct{921};
t586 = ct{922};
t5861 = ct{923};
t587 = ct{924};
t5872 = ct{925};
t5878 = ct{926};
t5881 = ct{927};
t5882 = ct{928};
t5883 = ct{929};
t5888 = ct{930};
t5889 = ct{931};
t589 = ct{932};
t5892 = ct{933};
t5894 = ct{934};
t5895 = ct{935};
t5897 = ct{936};
t5898 = ct{937};
t5899 = ct{938};
t590 = ct{939};
t5905 = ct{940};
t5915 = ct{941};
t5916 = ct{942};
t5918 = ct{943};
t592 = ct{944};
t5921 = ct{945};
t5922 = ct{946};
t5925 = ct{947};
t5926 = ct{948};
t5928 = ct{949};
t5930 = ct{950};
t5934 = ct{951};
t5937 = ct{952};
t5938 = ct{953};
t5939 = ct{954};
t594 = ct{955};
t5940 = ct{956};
t5942 = ct{957};
t5943 = ct{958};
t5944 = ct{959};
t5947 = ct{960};
t5950 = ct{961};
t5951 = ct{962};
t5952 = ct{963};
t5954 = ct{964};
t5958 = ct{965};
t596 = ct{966};
t5960 = ct{967};
t5961 = ct{968};
t5967 = ct{969};
t5968 = ct{970};
t597 = ct{971};
t5973 = ct{972};
t5974 = ct{973};
t5977 = ct{974};
t5978 = ct{975};
t5979 = ct{976};
t5982 = ct{977};
t5984 = ct{978};
t5985 = ct{979};
t5986 = ct{980};
t5988 = ct{981};
t5996 = ct{982};
t6 = ct{983};
t600 = ct{984};
t6005 = ct{985};
t6008 = ct{986};
t6009 = ct{987};
t6013 = ct{988};
t6017 = ct{989};
t6019 = ct{990};
t602 = ct{991};
t6026 = ct{992};
t603 = ct{993};
t6035 = ct{994};
t6037 = ct{995};
t604 = ct{996};
t6042 = ct{997};
t6044 = ct{998};
t6046 = ct{999};
t6047 = ct{1000};
t6048 = ct{1001};
t605 = ct{1002};
t6053 = ct{1003};
t6056 = ct{1004};
t6060 = ct{1005};
t6074 = ct{1006};
t6081 = ct{1007};
t609 = ct{1008};
t6095 = ct{1009};
t610 = ct{1010};
t6103 = ct{1011};
t6108 = ct{1012};
t6109 = ct{1013};
t611 = ct{1014};
t6118 = ct{1015};
t6119 = ct{1016};
t612 = ct{1017};
t6123 = ct{1018};
t6125 = ct{1019};
t6127 = ct{1020};
t613 = ct{1021};
t6136 = ct{1022};
t614 = ct{1023};
t6142 = ct{1024};
t6145 = ct{1025};
t6146 = ct{1026};
t6147 = ct{1027};
t615 = ct{1028};
t6152 = ct{1029};
t6155 = ct{1030};
t6158 = ct{1031};
t616 = ct{1032};
t6162 = ct{1033};
t6164 = ct{1034};
t6165 = ct{1035};
t6167 = ct{1036};
t6170 = ct{1037};
t6171 = ct{1038};
t6175 = ct{1039};
t6177 = ct{1040};
t6179 = ct{1041};
t618 = ct{1042};
t6182 = ct{1043};
t6183 = ct{1044};
t6189 = ct{1045};
t619 = ct{1046};
t6191 = ct{1047};
t6194 = ct{1048};
t6195 = ct{1049};
t6196 = ct{1050};
t6197 = ct{1051};
t620 = ct{1052};
t6202 = ct{1053};
t6203 = ct{1054};
t6209 = ct{1055};
t621 = ct{1056};
t6210 = ct{1057};
t6213 = ct{1058};
t6215 = ct{1059};
t6216 = ct{1060};
t6218 = ct{1061};
t622 = ct{1062};
t6220 = ct{1063};
t6222 = ct{1064};
t6225 = ct{1065};
t6226 = ct{1066};
t623 = ct{1067};
t6230 = ct{1068};
t6231 = ct{1069};
t6232 = ct{1070};
t6235 = ct{1071};
t6239 = ct{1072};
t624 = ct{1073};
t6244 = ct{1074};
t6248 = ct{1075};
t6249 = ct{1076};
t625 = ct{1077};
t6252 = ct{1078};
t6255 = ct{1079};
t6271 = ct{1080};
t6272 = ct{1081};
t6274 = ct{1082};
t6276 = ct{1083};
t6280 = ct{1084};
t6282 = ct{1085};
t6289 = ct{1086};
t6293 = ct{1087};
t6294 = ct{1088};
t6296 = ct{1089};
t6303 = ct{1090};
t6307 = ct{1091};
t6312 = ct{1092};
t6313 = ct{1093};
t632 = ct{1094};
t6322 = ct{1095};
t6329 = ct{1096};
t6330 = ct{1097};
t6332 = ct{1098};
t6345 = ct{1099};
t6349 = ct{1100};
t6350 = ct{1101};
t6351 = ct{1102};
t6352 = ct{1103};
t6359 = ct{1104};
t6360 = ct{1105};
t6362 = ct{1106};
t638 = ct{1107};
t6380 = ct{1108};
t6382 = ct{1109};
t6385 = ct{1110};
t6386 = ct{1111};
t6391 = ct{1112};
t6393 = ct{1113};
t6395 = ct{1114};
t6396 = ct{1115};
t6397 = ct{1116};
t6399 = ct{1117};
t640 = ct{1118};
t6400 = ct{1119};
t6401 = ct{1120};
t6402 = ct{1121};
t6405 = ct{1122};
t6406 = ct{1123};
t6407 = ct{1124};
t6412 = ct{1125};
t6414 = ct{1126};
t6422 = ct{1127};
t6426 = ct{1128};
t6431 = ct{1129};
t6433 = ct{1130};
t6434 = ct{1131};
t6442 = ct{1132};
t6443 = ct{1133};
t6445 = ct{1134};
t6449 = ct{1135};
t6451 = ct{1136};
t6454 = ct{1137};
t6462 = ct{1138};
t6463 = ct{1139};
t6465 = ct{1140};
t6468 = ct{1141};
t6470 = ct{1142};
t6473 = ct{1143};
t6477 = ct{1144};
t6486 = ct{1145};
t6487 = ct{1146};
t6489 = ct{1147};
t6503 = ct{1148};
t6504 = ct{1149};
t6513 = ct{1150};
t6521 = ct{1151};
t6536 = ct{1152};
t6537 = ct{1153};
t6544 = ct{1154};
t6546 = ct{1155};
t6548 = ct{1156};
t6551 = ct{1157};
t6557 = ct{1158};
t6560 = ct{1159};
t6561 = ct{1160};
t6562 = ct{1161};
t6563 = ct{1162};
t6564 = ct{1163};
t6571 = ct{1164};
t6574 = ct{1165};
t6580 = ct{1166};
t6593 = ct{1167};
t6594 = ct{1168};
t6604 = ct{1169};
t6605 = ct{1170};
t6607 = ct{1171};
t6610 = ct{1172};
t6648 = ct{1173};
t6656 = ct{1174};
t6664 = ct{1175};
t6669 = ct{1176};
t6672 = ct{1177};
t6676 = ct{1178};
t6677 = ct{1179};
t6694 = ct{1180};
t6695 = ct{1181};
t6699 = ct{1182};
t6711 = ct{1183};
t6714 = ct{1184};
t6715 = ct{1185};
t6721 = ct{1186};
t6724 = ct{1187};
t6727 = ct{1188};
t6729 = ct{1189};
t6738 = ct{1190};
t6743 = ct{1191};
t6746 = ct{1192};
t6747 = ct{1193};
t6753 = ct{1194};
t6756 = ct{1195};
t6758 = ct{1196};
t6774 = ct{1197};
t6776 = ct{1198};
t6783 = ct{1199};
t6807 = ct{1200};
t681 = ct{1201};
t6818 = ct{1202};
t6821 = ct{1203};
t6831 = ct{1204};
t6832 = ct{1205};
t6838 = ct{1206};
t684 = ct{1207};
t6841 = ct{1208};
t6842 = ct{1209};
t6844 = ct{1210};
t6847 = ct{1211};
t6849 = ct{1212};
t6851 = ct{1213};
t6856 = ct{1214};
t6859 = ct{1215};
t6860 = ct{1216};
t6865 = ct{1217};
t6879 = ct{1218};
t6884 = ct{1219};
t6888 = ct{1220};
t6890 = ct{1221};
t6891 = ct{1222};
t6892 = ct{1223};
t6894 = ct{1224};
t6898 = ct{1225};
t6903 = ct{1226};
t6909 = ct{1227};
t6911 = ct{1228};
t6914 = ct{1229};
t6915 = ct{1230};
t6916 = ct{1231};
t6918 = ct{1232};
t6919 = ct{1233};
t6921 = ct{1234};
t6922 = ct{1235};
t6924 = ct{1236};
t6926 = ct{1237};
t6927 = ct{1238};
t6928 = ct{1239};
t6930 = ct{1240};
t6935 = ct{1241};
t6936 = ct{1242};
t6937 = ct{1243};
t6939 = ct{1244};
t6941 = ct{1245};
t6944 = ct{1246};
t6946 = ct{1247};
t6952 = ct{1248};
t6953 = ct{1249};
t6954 = ct{1250};
t6960 = ct{1251};
t6975 = ct{1252};
t6977 = ct{1253};
t6983 = ct{1254};
t6984 = ct{1255};
t6985 = ct{1256};
t6986 = ct{1257};
t6989 = ct{1258};
t6990 = ct{1259};
t6991 = ct{1260};
t6994 = ct{1261};
t7 = ct{1262};
t7000 = ct{1263};
t7003 = ct{1264};
t7006 = ct{1265};
t7008 = ct{1266};
t7010 = ct{1267};
t7011 = ct{1268};
t7012 = ct{1269};
t7022 = ct{1270};
t7023 = ct{1271};
t7026 = ct{1272};
t7027 = ct{1273};
t7030 = ct{1274};
t7031 = ct{1275};
t7032 = ct{1276};
t7033 = ct{1277};
t7035 = ct{1278};
t7036 = ct{1279};
t7039 = ct{1280};
t7040 = ct{1281};
t7042 = ct{1282};
t7044 = ct{1283};
t7045 = ct{1284};
t7048 = ct{1285};
t7051 = ct{1286};
t7052 = ct{1287};
t7053 = ct{1288};
t7054 = ct{1289};
t7055 = ct{1290};
t7059 = ct{1291};
t7060 = ct{1292};
t7061 = ct{1293};
t7066 = ct{1294};
t7067 = ct{1295};
t7069 = ct{1296};
t7071 = ct{1297};
t7072 = ct{1298};
t7074 = ct{1299};
t7075 = ct{1300};
t7076 = ct{1301};
t7077 = ct{1302};
t7078 = ct{1303};
t7081 = ct{1304};
t7082 = ct{1305};
t7084 = ct{1306};
t7085 = ct{1307};
t7086 = ct{1308};
t7087 = ct{1309};
t7088 = ct{1310};
t7089 = ct{1311};
t7091 = ct{1312};
t7093 = ct{1313};
t7095 = ct{1314};
t7096 = ct{1315};
t7098 = ct{1316};
t7100 = ct{1317};
t7102 = ct{1318};
t7103 = ct{1319};
t7104 = ct{1320};
t7110 = ct{1321};
t7113 = ct{1322};
t7114 = ct{1323};
t7115 = ct{1324};
t712 = ct{1325};
t7120 = ct{1326};
t7122 = ct{1327};
t7123 = ct{1328};
t7124 = ct{1329};
t7127 = ct{1330};
t7128 = ct{1331};
t7129 = ct{1332};
t7130 = ct{1333};
t7133 = ct{1334};
t7134 = ct{1335};
t7136 = ct{1336};
t7137 = ct{1337};
t7140 = ct{1338};
t7141 = ct{1339};
t7142 = ct{1340};
t7143 = ct{1341};
t7148 = ct{1342};
t7149 = ct{1343};
t7156 = ct{1344};
t7158 = ct{1345};
t7168 = ct{1346};
t7170 = ct{1347};
t7174 = ct{1348};
t7176 = ct{1349};
t7191 = ct{1350};
t7192 = ct{1351};
t7194 = ct{1352};
t72 = ct{1353};
t7201 = ct{1354};
t7203 = ct{1355};
t7204 = ct{1356};
t7206 = ct{1357};
t7207 = ct{1358};
t7208 = ct{1359};
t7215 = ct{1360};
t7217 = ct{1361};
t7221 = ct{1362};
t7222 = ct{1363};
t7223 = ct{1364};
t7224 = ct{1365};
t7226 = ct{1366};
t7231 = ct{1367};
t7234 = ct{1368};
t7235 = ct{1369};
t7237 = ct{1370};
t724 = ct{1371};
t7242 = ct{1372};
t7243 = ct{1373};
t7244 = ct{1374};
t7245 = ct{1375};
t7246 = ct{1376};
t7247 = ct{1377};
t7248 = ct{1378};
t7254 = ct{1379};
t7255 = ct{1380};
t7256 = ct{1381};
t7257 = ct{1382};
t7258 = ct{1383};
t7261 = ct{1384};
t7263 = ct{1385};
t7267 = ct{1386};
t7268 = ct{1387};
t7269 = ct{1388};
t7270 = ct{1389};
t7271 = ct{1390};
t7272 = ct{1391};
t7273 = ct{1392};
t7274 = ct{1393};
t7276 = ct{1394};
t7277 = ct{1395};
t7279 = ct{1396};
t7281 = ct{1397};
t7284 = ct{1398};
t7288 = ct{1399};
t7289 = ct{1400};
t7296 = ct{1401};
t7297 = ct{1402};
t73 = ct{1403};
t7300 = ct{1404};
t7304 = ct{1405};
t7305 = ct{1406};
t7307 = ct{1407};
t7308 = ct{1408};
t7309 = ct{1409};
t7310 = ct{1410};
t7312 = ct{1411};
t7319 = ct{1412};
t7321 = ct{1413};
t7322 = ct{1414};
t7324 = ct{1415};
t7327 = ct{1416};
t7331 = ct{1417};
t7332 = ct{1418};
t7336 = ct{1419};
t7337 = ct{1420};
t7339 = ct{1421};
t7340 = ct{1422};
t7341 = ct{1423};
t7342 = ct{1424};
t7343 = ct{1425};
t7344 = ct{1426};
t7346 = ct{1427};
t7348 = ct{1428};
t7349 = ct{1429};
t7350 = ct{1430};
t7362 = ct{1431};
t7363 = ct{1432};
t7366 = ct{1433};
t7367 = ct{1434};
t7368 = ct{1435};
t7369 = ct{1436};
t7371 = ct{1437};
t7372 = ct{1438};
t7373 = ct{1439};
t7374 = ct{1440};
t7375 = ct{1441};
t7376 = ct{1442};
t7377 = ct{1443};
t7378 = ct{1444};
t7379 = ct{1445};
t738 = ct{1446};
t7380 = ct{1447};
t7381 = ct{1448};
t7382 = ct{1449};
t7383 = ct{1450};
t7384 = ct{1451};
t7385 = ct{1452};
t7386 = ct{1453};
t7387 = ct{1454};
t7388 = ct{1455};
t7390 = ct{1456};
t7391 = ct{1457};
t7392 = ct{1458};
t7393 = ct{1459};
t7394 = ct{1460};
t7395 = ct{1461};
t7396 = ct{1462};
t7398 = ct{1463};
t7399 = ct{1464};
t7402 = ct{1465};
t7403 = ct{1466};
t7405 = ct{1467};
t741 = ct{1468};
t7410 = ct{1469};
t7413 = ct{1470};
t7414 = ct{1471};
t742 = ct{1472};
t7421 = ct{1473};
t7423 = ct{1474};
t7425 = ct{1475};
t7426 = ct{1476};
t7427 = ct{1477};
t7428 = ct{1478};
t7429 = ct{1479};
t7430 = ct{1480};
t7431 = ct{1481};
t7433 = ct{1482};
t7434 = ct{1483};
t7435 = ct{1484};
t7437 = ct{1485};
t7439 = ct{1486};
t7440 = ct{1487};
t7442 = ct{1488};
t7444 = ct{1489};
t7446 = ct{1490};
t7447 = ct{1491};
t7448 = ct{1492};
t7450 = ct{1493};
t7453 = ct{1494};
t7455 = ct{1495};
t7458 = ct{1496};
t7459 = ct{1497};
t7461 = ct{1498};
t7463 = ct{1499};
t7465 = ct{1500};
t7468 = ct{1501};
t7469 = ct{1502};
t7470 = ct{1503};
t7476 = ct{1504};
t7477 = ct{1505};
t7479 = ct{1506};
t7480 = ct{1507};
t7481 = ct{1508};
t7482 = ct{1509};
t7483 = ct{1510};
t7485 = ct{1511};
t7486 = ct{1512};
t7487 = ct{1513};
t7488 = ct{1514};
t7490 = ct{1515};
t7491 = ct{1516};
t7492 = ct{1517};
t7493 = ct{1518};
t7494 = ct{1519};
t7495 = ct{1520};
t7496 = ct{1521};
t7498 = ct{1522};
t7499 = ct{1523};
t7500 = ct{1524};
t7501 = ct{1525};
t7502 = ct{1526};
t7503 = ct{1527};
t7504 = ct{1528};
t7507 = ct{1529};
t7508 = ct{1530};
t7509 = ct{1531};
t7510 = ct{1532};
t7511 = ct{1533};
t7512 = ct{1534};
t7513 = ct{1535};
t7515 = ct{1536};
t7516 = ct{1537};
t7517 = ct{1538};
t7519 = ct{1539};
t7521 = ct{1540};
t7522 = ct{1541};
t7523 = ct{1542};
t7524 = ct{1543};
t7525 = ct{1544};
t7526 = ct{1545};
t7527 = ct{1546};
t7529 = ct{1547};
t753 = ct{1548};
t7530 = ct{1549};
t7531 = ct{1550};
t7533 = ct{1551};
t7534 = ct{1552};
t7536 = ct{1553};
t7537 = ct{1554};
t7538 = ct{1555};
t7541 = ct{1556};
t7542 = ct{1557};
t7543 = ct{1558};
t7546 = ct{1559};
t7548 = ct{1560};
t7549 = ct{1561};
t7550 = ct{1562};
t7552 = ct{1563};
t7554 = ct{1564};
t7555 = ct{1565};
t7557 = ct{1566};
t7558 = ct{1567};
t7562 = ct{1568};
t7563 = ct{1569};
t7565 = ct{1570};
t7567 = ct{1571};
t7568 = ct{1572};
t7571 = ct{1573};
t7572 = ct{1574};
t7574 = ct{1575};
t7577 = ct{1576};
t7580 = ct{1577};
t7584 = ct{1578};
t7587 = ct{1579};
t7593 = ct{1580};
t7595 = ct{1581};
t7596 = ct{1582};
t7597 = ct{1583};
t7599 = ct{1584};
t760 = ct{1585};
t781 = ct{1586};
t792 = ct{1587};
t797 = ct{1588};
t8 = ct{1589};
t803 = ct{1590};
t81 = ct{1591};
t825 = ct{1592};
t826 = ct{1593};
t827 = ct{1594};
t832 = ct{1595};
t845 = ct{1596};
t848 = ct{1597};
t852 = ct{1598};
t86 = ct{1599};
t866 = ct{1600};
t868 = ct{1601};
t869 = ct{1602};
t874 = ct{1603};
t875 = ct{1604};
t877 = ct{1605};
t881 = ct{1606};
t893 = ct{1607};
t899 = ct{1608};
t9 = ct{1609};
t90 = ct{1610};
t902 = ct{1611};
t903 = ct{1612};
t908 = ct{1613};
t91 = ct{1614};
t910 = ct{1615};
t911 = ct{1616};
t912 = ct{1617};
t915 = ct{1618};
t917 = ct{1619};
t919 = ct{1620};
t922 = ct{1621};
t926 = ct{1622};
t928 = ct{1623};
t930 = ct{1624};
t931 = ct{1625};
t932 = ct{1626};
t934 = ct{1627};
t940 = ct{1628};
t944 = ct{1629};
t947 = ct{1630};
t95 = ct{1631};
t952 = ct{1632};
t957 = ct{1633};
t958 = ct{1634};
t968 = ct{1635};
t970 = ct{1636};
t971 = ct{1637};
t972 = ct{1638};
t975 = ct{1639};
t976 = ct{1640};
t984 = ct{1641};
t985 = ct{1642};
t986 = ct{1643};
t989 = ct{1644};
t99 = ct{1645};
t991 = ct{1646};
t998 = ct{1647};
et403 = t3.*t5.*t18.*7.093613755211269e-13+t3.*t9.*t18.*5.4093083807222e-13;
et404 = t4.*t7.*t19.*2.143506553146841e-6+t3.*t4.*t5.*t8.*1.378434177095879e-6;
et405 = t3.*t4.*t8.*t9.*7.492102979241942e-7-t4.*t5.*t7.*t9.*1.408936125616489e-6;
et406 = t3.*t4.*t8.*t19.*1.408936125616489e-6;
et407 = t5961-t6215-t6473+(t91.*t5824.*(t5670+t4.*(t1458-t5665)))./1.316403645856965e+67+(t5824.*t6103.*(t29-t30))./1.316403645856965e+67;
et408 = (t5822.*t6230.*(t29-t30))./1.316403645856965e+67;
et409 = t5985-t6274-t6503+t91.*t5824.*(t5670+t4.*(t1458-t5665)).*5.520609140571798e-70;
et410 = t5824.*t6103.*(t29-t30).*5.520609140571798e-70;
et411 = t5822.*t6230.*(t29-t30).*5.520609140571798e-70;
et412 = t190.*2.410558945879715e-5;
et413 = t197.*(-1.741515101016883e-7);
et414 = t199.*6.030092636960013e-10;
et415 = t201.*(-1.933448131481258e-7);
et416 = t202.*8.816214851569211e-8+t2797+t2881+t3378+t3397+t3532+t3772+t4392+t6017+t6125+t6127+t7288+t7289+t7319+t7458+t7461+t7483;
et417 = (t6927.*(-t6729+t5784.*(t4148+t5.*(t2421-t4158))+(t5824.*t6468.*(t29-t30))./1.316403645856965e+67))./2.0;
et418 = t6926.*(t6313+(t91.*t5824.*(t6218+t5.*(t3136-t5691)))./1.316403645856965e+67+(t5824.*t6470.*(t29-t30))./1.316403645856965e+67).*(-1.0./2.0);
et419 = t4.*t190.*3.132594654525011e-6;
et420 = t8.*t190.*6.869965607067206e-6;
et421 = t7.*t200.*1.109015314093284e-9;
et422 = t17.*t190.*8.839415756040337e-8;
et423 = t18.*t190.*(-7.333437703759851e-7);
et424 = t8.*t201.*3.987438959506341e-7;
et425 = t18.*t197.*3.483030202033766e-7+(t318.*t7078)./2.0+(t1427.*t7069)./2.0+(t1429.*t7067)./2.0-(t5636.*t5688)./2.0-(t5633.*t5850)./2.0+(t5634.*t5851)./2.0-(t5979.*t7075)./2.0-(t6391.*t7123)./2.0-(t6395.*t7122)./2.0+(t6462.*t7281)./2.0-(t6463.*t7284)./2.0-(t7027.*t7274)./2.0-(t7026.*t7276)./2.0;
et426 = (t6699.*(t6005-t6486+(t5824.*t6230.*(t29-t30))./1.316403645856965e+67))./2.0+(t6919.*(et407+et408))./2.0-(t6136.*(et409+et410+et411))./2.0;
et427 = t4.*t8.*t190.*6.405762010734574e-7;
et428 = t17.*t18.*t190.*3.666718851879926e-7+t3.*t34.*t191.*2.068449163602394e-23;
et429 = t8.*t34.*t191.*(-1.204667623436253e-25);
et430 = t4.*t8.*t17.*t190.*(-3.202881005367287e-7);
et431 = t3.*t4.*t34.*t191.*(-6.665727339062343e-22);
et432 = t3.*t7.*t34.*t191.*(-1.920362656146042e-23);
et433 = t3.*t8.*t34.*t191.*3.039465264482168e-22;
et434 = t4.*t7.*t34.*t191.*7.162119963290503e-26-t3.*t18.*t34.*t191.*4.136898327204789e-23;
et435 = t8.*t17.*t34.*t191.*2.409335246872506e-25-t3.*t4.*t8.*t34.*t191.*4.735999576397893e-23;
et436 = t3.*t7.*t18.*t34.*t191.*(-7.965944976538977e-23)+t3.*t4.*t7.*t8.*t34.*t191.*6.95825747372931e-23;
et437 = t5986-t6272+t6294+t6397-t6504+t6664+t6669-t6774+t91.*t5824.*(t5670+t4.*(t1458-t5665)).*1.015171749786156e-71;
et438 = t5824.*t6103.*(t29-t30).*1.015171749786156e-71;
et439 = t5822.*t6230.*(t29-t30).*1.015171749786156e-71;
et440 = t5822.*t6468.*(t29-t30).*1.065477564130357e-78;
et441 = t5961-t6215-t6473+(t91.*t5824.*(t5670+t4.*(t1458-t5665)))./1.316403645856965e+67+(t5824.*t6103.*(t29-t30))./1.316403645856965e+67;
et442 = (t5822.*t6230.*(t29-t30))./1.316403645856965e+67;
et443 = t922+t934+t940+t989+t1039+t1050+t1056+t1069+t1083+t1099+t1106+t1133+t1150+t1177+t1179+t1185+t1191+t1196+t1205+t1221+t1225+t1233+t1250+t1253+t1273+t1274+t1306+t1316+t1322+t1330+t1331+t1337+t1342+t1348+t1353+t1379+t1391+t1402+t1407+t1411+t1413+t1419+t1423+t1436+t1443+t1445+t1454+t1457+t1486+t1487+t1767+t1827+t1873+t1992+t2130+t2180+t2474+t2481-t5961.*2.180205e-5+t6215.*2.180205e-5+t5.*t7274.*7.01299275e-12;
et444 = t9.*t7276.*(-7.01299275e-12)+(t9.*t7450)./2.0-(t5894.*(t5772+t5861.*((t197.*(t29-t30))./9.007199254740992e+15+t3.*(t3219-t3230)).*2.0+t5810.*(t3136-t5691).*2.0))./2.0-(t5.*(et437+et438+et439+et440))./2.0+(t1426.*(et441+et442))./2.0;
et445 = t91.*t5824.*(t5670+t4.*(t1458-t5665)).*(-1.656182742171539e-72);
et446 = t91.*t5822.*t6216.*1.656182742171539e-72;
et447 = t5824.*t6103.*(t29-t30).*(-1.656182742171539e-72);
et448 = t5822.*t6230.*(t29-t30).*(-1.656182742171539e-72);
et449 = t236+t314+t410+t468-t529+t531+t6332-t6783+t5784.*(t4148+t5.*(t2421-t4158)).*7.26350610236655e-5+t91.*t5824.*(t6218+t5.*(t3136-t5691)).*1.015171749786156e-71;
et450 = t5.*t7.*t8.*(-3.546806877605634e-13)-t7.*t8.*t9.*2.7046541903611e-13;
et451 = t5824.*t6468.*(t29-t30).*5.517689141340903e-72;
et452 = t5824.*t6470.*(t29-t30).*1.015171749786156e-71;
et453 = t5986-t6272+t6294+t6397-t6504+t6664+t6669-t6774+t91.*t5824.*(t5670+t4.*(t1458-t5665)).*1.015171749786156e-71;
et454 = t5824.*t6103.*(t29-t30).*1.015171749786156e-71;
et455 = t5822.*t6230.*(t29-t30).*1.015171749786156e-71;
et456 = t5822.*t6468.*(t29-t30).*1.065477564130357e-78;
et457 = -t6729+t5784.*(t4148+t5.*(t2421-t4158))+(t5824.*t6468.*(t29-t30))./1.316403645856965e+67;
et458 = (-t5942+t6171+t6183-t6604+t6831.*1.40259855e-11-t6851+t6903+t6924+t6216.*(t5670+t4.*(t1458-t5665)).*1.45270122047331e-4).*(-1.0./2.0);
et459 = t5961-t6215-t6473+(t91.*t5824.*(t5670+t4.*(t1458-t5665)))./1.316403645856965e+67+(t5824.*t6103.*(t29-t30))./1.316403645856965e+67;
et460 = (t5822.*t6230.*(t29-t30))./1.316403645856965e+67;
et461 = t724+t825+t874+t903+t926+t957+t968+t970+t984+t1004+t1016+t1061+t1081+t1095+t1101+t1108+t1144+t1152+t1155+t1170+t1171+t1174+t1193+t1203+t1207+t1215+t1224+t1245+t1254+t1258+t1285+t1288+t1300+t1301+t1323+t1333+t1344+t1345+t1365+t1377+t1380+t1383+t1388+t1409+t1428+t1440+t1692+t1731+t1769+t1847+t1977+t1981;
et462 = (t7402.*(t6313+(t91.*t5824.*(t6218+t5.*(t3136-t5691)))./1.316403645856965e+67+(t5824.*t6470.*(t29-t30))./1.316403645856965e+67))./2.0;
et463 = t1429.*(-t5944+t6118.*1.246862701090643e-6+t6145+t6146+t6152-t6607+t6831.*3.383302988283333e-6-t6838-t6844-t6856+t6884+t6890+t6909+t6914+t6216.*(t5670+t4.*(t1458-t5665)).*6.293113355513489e-13).*(-1.0./2.0)-(t1427.*t7534)./2.0-(t6821.*t7480)./2.0+(t7204.*t7276)./2.0+(t7267.*t7305)./2.0;
et464 = t7269.*t7304.*(-1.0./2.0)-(t7130.*t7450)./2.0-(t7500.*(t6005-t6486+(t5824.*t6230.*(t29-t30))./1.316403645856965e+67))./2.0-(t7072.*(et449+et450+et451+et452))./2.0+(t7129.*(et453+et454+et455+et456))./2.0+et457.*et458-(t7327.*(et459+et460))./2.0;
et465 = t318.*(-t5943+t6170-t6177+t6179+t6189-t6605+t6831.*3.146556677756745e-13+t6847-t6849+t6865+t6898+t6921-t6922+t6216.*(t5670+t4.*(t1458-t5665)).*8.40184101230148e-6+t6465.*(t5670+t4.*(t1458-t5665)).*4.126305279697715e-13).*(-1.0./2.0);
et466 = (t7274.*(t5709-t6255+t6282+t6296-t7003+t6216.*(t6218+t5.*(t3136-t5691)).*1.40259855e-11))./2.0;
et467 = t6391-t2.*t5.*t200.*2.591581422298263e-2+t2.*t9.*t197.*2.591581422298263e-2;
et468 = t5.*t6.*t200.*(-1.069035573404174e-1)+t6.*t9.*t197.*1.069035573404174e-1;
et469 = t2.*t4.*t5.*t34.*t191.*2.473154649626116e-18;
et470 = t2.*t3.*t9.*t34.*t191.*1.470366592725919e-18;
et471 = t4.*t5.*t6.*t34.*t191.*1.020184153286453e-17;
et472 = t3.*t6.*t9.*t34.*t191.*6.065308926991484e-18;
et473 = t2.*t5.*t7.*t8.*t34.*t191.*1.470366592725919e-18;
et474 = t5.*t6.*t7.*t8.*t34.*t191.*6.065308926991484e-18;
et475 = t6395+t2.*t5.*t197.*2.591581422298263e-2+t5.*t6.*t197.*1.069035573404174e-1;
et476 = t2.*t9.*t200.*2.591581422298263e-2+t6.*t9.*t200.*1.069035573404174e-1;
et477 = t2.*t3.*t5.*t34.*t191.*1.470366592725919e-18;
et478 = t3.*t5.*t6.*t34.*t191.*6.065308926991484e-18;
et479 = t2.*t4.*t9.*t34.*t191.*(-2.473154649626116e-18);
et480 = t4.*t6.*t9.*t34.*t191.*(-1.020184153286453e-17);
et481 = t2.*t7.*t8.*t9.*t34.*t191.*(-1.470366592725919e-18);
et482 = t6.*t7.*t8.*t9.*t34.*t191.*(-6.065308926991484e-18);
et483 = t5851-t2.*t200.*2.591581422298263e-2-t6.*t200.*1.069035573404174e-1;
et484 = t2.*t4.*t34.*t191.*2.473154649626116e-18;
et485 = t4.*t6.*t34.*t191.*1.020184153286453e-17;
et486 = t2.*t7.*t8.*t34.*t191.*1.470366592725919e-18;
et487 = t6.*t7.*t8.*t34.*t191.*6.065308926991484e-18;
et488 = t5636+t2.*t197.*2.591581422298263e-2+t6.*t197.*1.069035573404174e-1;
et489 = t2.*t3.*t34.*t191.*1.470366592725919e-18;
et490 = t3.*t6.*t34.*t191.*6.065308926991484e-18;
et491 = t5985-t6274-t6503+t91.*t5824.*(t5670+t4.*(t1458-t5665)).*5.520609140571798e-70;
et492 = t5824.*t6103.*(t29-t30).*5.520609140571798e-70;
et493 = t5822.*t6230.*(t29-t30).*5.520609140571798e-70;
et494 = t190.*3.972959979360314e-5;
et495 = t197.*(-1.741514900016076e-7);
et496 = t199.*(-2.972018635868086e-7);
et497 = t201.*(-1.933447931569648e-7);
et498 = t202.*1.503108354312723e-7+t2797+t2881+t3378+t3397+t3532+t3772+t4392+t6017+t6125+t6127+t7288+t7289+t7319+t7458+t7461+t7483-(t7123.*(et467+et468+et469+et470+et471+et472+et473+et474))./2.0-(t7122.*(et475+et476+et477+et478+et479+et480+et481+et482))./2.0;
et499 = t2.*t190.*1.159365147749227e-5;
et500 = t4.*t190.*5.340873918305004e-6;
et501 = t5.*t190.*(-3.522139685937468e-7);
et502 = t6.*t190.*4.782418082044221e-5;
et503 = t2.*t196.*(-4.669183776451438e-9);
et504 = t8.*t190.*6.869964896737376e-6;
et505 = t9.*t190.*(-1.914362954197335e-7);
et506 = t5.*t196.*(-1.035263579950933e-7);
et507 = t5.*t197.*9.85540603699085e-14;
et508 = t6.*t196.*(-1.926053147642049e-8);
et509 = t2.*t201.*(-8.982831472475836e-7);
et510 = t2.*t202.*6.983466588986496e-7;
et511 = t5.*t199.*1.040904107263154e-7;
et512 = t5.*t200.*(-7.515341589066688e-14);
et513 = t9.*t196.*1.904729159303931e-7;
et514 = t9.*t197.*7.515341589066688e-14;
et515 = t5.*t202.*1.904729159303931e-7;
et516 = t6.*t201.*(-3.705446532123684e-6);
et517 = t7.*t200.*(-5.465942862546103e-7);
et518 = t17.*t190.*(-2.141523093067362e-7);
et519 = t6.*t202.*2.880702163193259e-6;
et520 = t9.*t199.*(-1.915106880546619e-7);
et521 = t18.*t190.*(-2.592703454263624e-7);
et522 = t8.*t201.*1.409740858462195e-7;
et523 = t9.*t200.*9.85540603699085e-14;
et524 = t19.*t190.*(-3.600077483162727e-7);
et525 = t9.*t202.*1.035263579950933e-7;
et526 = t18.*t197.*3.483029800032151e-7;
et527 = t19.*t199.*5.956097457010092e-7+t199.*t1081+(t7060.*t7281)./2.0-(t7061.*t7284)./2.0-(t5633.*(t1493+t1495+t4143+t4152+t4166+t4173+t5850))./2.0-(t7075.*(t1493+t1495+t4143+t4152+t4166+t4173+t5979))./2.0+(t5634.*(et483+et484+et485+et486+et487))./2.0-(t5688.*(et488+et489+et490))./2.0-(t6832.*(et491+et492+et493))./2.0;
et528 = t2.*t4.*t190.*1.174618149684797e-6;
et529 = t4.*t5.*t190.*6.767920795046621e-6;
et530 = t2.*t8.*t190.*1.510911056662081e-6;
et531 = t4.*t6.*t190.*4.845337199807718e-6;
et532 = t4.*t8.*t190.*6.405761271399419e-7;
et533 = t2.*t5.*t196.*(-4.809851931591181e-7);
et534 = t4.*t9.*t190.*3.678518742089733e-6;
et535 = t5.*t9.*t190.*(-5.477033015687036e-7);
et536 = t6.*t8.*t190.*6.232556129334532e-6;
et537 = t2.*t9.*t196.*8.849403575532205e-7;
et538 = t5.*t6.*t196.*(-1.984079208716435e-6);
et539 = t2.*t5.*t202.*8.849403575532205e-7;
et540 = t6.*t9.*t196.*3.65040710056658e-6;
et541 = t5.*t7.*t200.*1.914362954197335e-7;
et542 = t5.*t17.*t190.*3.522139685937468e-7;
et543 = t2.*t9.*t202.*4.809851931591181e-7;
et544 = t5.*t6.*t202.*3.65040710056658e-6;
et545 = t5.*t9.*t199.*(-3.914968611854366e-7);
et546 = t5.*t18.*t190.*7.044279371874937e-7;
et547 = t5.*t8.*t201.*(-3.830213761093238e-7);
et548 = t7.*t9.*t199.*(-1.812542008830624e-13);
et549 = t7.*t9.*t200.*(-3.522139685937468e-7);
et550 = t9.*t17.*t190.*1.914362954197335e-7;
et551 = t6.*t9.*t202.*1.984079208716435e-6;
et552 = t9.*t18.*t190.*3.828725908394669e-7;
et553 = t8.*t9.*t201.*(-2.081808214526309e-7);
et554 = t5.*t18.*t197.*(-1.97108120739817e-13);
et555 = t9.*t18.*t197.*(-1.503068317813338e-13);
et556 = t17.*t18.*t190.*1.296351727131812e-7;
et557 = t7.*t19.*t200.*1.095406603137407e-6;
et558 = t17.*t19.*t190.*7.200154966325453e-7;
et559 = t18.*t19.*t190.*7.200154966325453e-7;
et560 = t3.*t34.*t191.*2.068448924867771e-23;
et561 = t8.*t19.*t201.*(-3.914968611854366e-7);
et562 = t8.*t34.*t191.*5.937379145611961e-23;
et563 = t2.*t4.*t5.*t190.*1.488468502176114e-6;
et564 = t2.*t4.*t9.*t190.*8.090164539562037e-7;
et565 = t4.*t5.*t6.*t190.*6.139979878798348e-6;
et566 = t4.*t5.*t8.*t190.*(-3.625084017661248e-13);
et567 = t4.*t6.*t9.*t190.*3.337218585173762e-6;
et568 = t4.*t8.*t9.*t190.*(-2.764345231392299e-13);
et569 = t4.*t8.*t17.*t190.*(-3.20288063569971e-7);
et570 = t5.*t7.*t9.*t200.*(-7.200154966325453e-7);
et571 = t5.*t9.*t17.*t190.*1.095406603137407e-6;
et572 = t5.*t9.*t18.*t190.*1.095406603137407e-6;
et573 = t5.*t8.*t9.*t201.*(-5.956097457010092e-7);
et574 = t5.*t17.*t18.*t190.*(-3.522139685937468e-7);
et575 = t3.*t4.*t34.*t191.*(-6.665726649850018e-22);
et576 = t3.*t5.*t34.*t191.*(-1.170555820174774e-29);
et577 = t2.*t7.*t34.*t191.*1.014379955242302e-24;
et578 = t4.*t5.*t34.*t191.*(-1.501384677893902e-29);
et579 = t9.*t17.*t18.*t190.*(-1.914362954197335e-7);
et580 = t3.*t7.*t34.*t191.*4.652457909778354e-23;
et581 = t3.*t8.*t34.*t191.*5.182094253151392e-22;
et582 = t4.*t7.*t34.*t191.*(-3.5299547261936e-23)-t3.*t9.*t34.*t191.*8.926194217330866e-30;
et583 = t5.*t7.*t34.*t191.*3.569159490576891e-22;
et584 = t4.*t9.*t34.*t191.*1.968873329708317e-29-t5.*t8.*t34.*t191.*2.079476307604284e-23;
et585 = t6.*t7.*t34.*t191.*4.184349554954289e-24;
et586 = t7.*t9.*t34.*t191.*(-6.566716233010319e-22);
et587 = t8.*t9.*t34.*t191.*3.825923403355188e-23-t17.*t18.*t19.*t190.*3.600077483162727e-7;
et588 = t3.*t18.*t34.*t191.*(-4.136897849735542e-23);
et589 = t8.*t17.*t34.*t191.*(-1.187475829122392e-22)-t8.*t19.*t34.*t191.*1.189885164369265e-22;
et590 = t4.*t5.*t8.*t17.*t190.*1.812542008830624e-13;
et591 = t4.*t8.*t9.*t17.*t190.*1.38217261569615e-13;
et592 = t2.*t3.*t4.*t34.*t191.*(-1.951519713778382e-22);
et593 = t2.*t3.*t8.*t34.*t191.*1.517157787127402e-22;
et594 = t3.*t4.*t6.*t34.*t191.*(-8.050080843605144e-22);
et595 = t2.*t5.*t7.*t34.*t191.*1.044940105312709e-22;
et596 = t5.*t9.*t17.*t18.*t190.*(-5.477033015687036e-7);
et597 = t3.*t4.*t8.*t34.*t191.*(-1.67439105057406e-23)-t3.*t5.*t7.*t34.*t191.*7.651846806710377e-23;
et598 = t3.*t5.*t8.*t34.*t191.*6.566716233010319e-22;
et599 = t4.*t5.*t7.*t34.*t191.*1.236312696227316e-23;
et600 = t3.*t6.*t8.*t34.*t191.*6.258324091040992e-22;
et601 = t2.*t7.*t9.*t34.*t191.*(-1.92253250945964e-22);
et602 = t5.*t6.*t7.*t34.*t191.*4.310411145274163e-22;
et603 = t3.*t7.*t9.*t34.*t191.*(-4.158952615208568e-23);
et604 = t3.*t8.*t9.*t34.*t191.*3.569159490576891e-22;
et605 = t4.*t7.*t9.*t34.*t191.*(-2.27462927135275e-23)-t5.*t7.*t8.*t34.*t191.*8.926194217330866e-30;
et606 = t5.*t8.*t9.*t34.*t191.*7.821166634427942e-23;
et607 = t6.*t7.*t9.*t34.*t191.*(-7.930507704503114e-22);
et608 = t7.*t8.*t9.*t34.*t191.*1.170555820174774e-29+t3.*t5.*t18.*t34.*t191.*2.341111640349547e-29;
et609 = t4.*t5.*t17.*t34.*t191.*3.002769355787804e-29-t3.*t7.*t18.*t34.*t191.*2.816323515853638e-23;
et610 = t3.*t7.*t19.*t34.*t191.*(-1.564233326885588e-22)+t3.*t9.*t18.*t34.*t191.*1.785238843466173e-29;
et611 = t4.*t7.*t19.*t34.*t191.*7.074233692313782e-23-t4.*t9.*t17.*t34.*t191.*3.937746659416635e-29;
et612 = t5.*t8.*t17.*t34.*t191.*4.158952615208568e-23-t8.*t9.*t17.*t34.*t191.*7.651846806710377e-23;
et613 = t8.*t17.*t19.*t34.*t191.*2.379770328738529e-22;
et614 = t2.*t3.*t5.*t8.*t34.*t191.*1.92253250945964e-22;
et615 = t3.*t4.*t5.*t8.*t34.*t191.*4.549258542705501e-23;
et616 = t2.*t3.*t8.*t9.*t34.*t191.*1.044940105312709e-22;
et617 = t3.*t4.*t7.*t8.*t34.*t191.*6.958256670626673e-23;
et618 = t3.*t5.*t6.*t8.*t34.*t191.*7.930507704503114e-22;
et619 = t3.*t4.*t8.*t9.*t34.*t191.*2.472625392454631e-23-t3.*t5.*t7.*t9.*t34.*t191.*2.379770328738529e-22;
et620 = t4.*t5.*t7.*t9.*t34.*t191.*(-4.649924393989671e-23);
et621 = t3.*t6.*t8.*t9.*t34.*t191.*4.310411145274163e-22;
et622 = t3.*t5.*t7.*t18.*t34.*t191.*7.651846806710377e-23+t3.*t4.*t8.*t19.*t34.*t191.*4.649924393989671e-23;
et623 = t3.*t7.*t9.*t18.*t34.*t191.*4.158952615208568e-23-t5.*t8.*t9.*t17.*t34.*t191.*1.564233326885588e-22;
et624 = t3.*t7.*t18.*t19.*t34.*t191.*7.821166634427942e-23-t3.*t4.*t5.*t7.*t8.*t34.*t191.*3.937746659416635e-29;
et625 = t3.*t4.*t5.*t8.*t9.*t34.*t191.*7.074233692313782e-23-t3.*t4.*t7.*t8.*t9.*t34.*t191.*3.002769355787804e-29;
et626 = t3.*t5.*t7.*t9.*t18.*t34.*t191.*1.189885164369265e-22;
et627 = -dq5.*(dq5.*(et352+et353+et354+et355+et356)+dq1.*t7595+dq2.*(et359+et360+et361)+dq6.*(et371+et372+et373)-dq3.*(t922+t934+t940+t989+t1039+t1050+t1056+t1069+t1083+t1099+t1106+t1133+t1150+t1177+t1179+t1185+t1191+t1196+t1205+t1221+t1225+t1233+t1250+t1253+t1273+t1274+t1306+t1316+t1322+t1330+t1331+t1337+t1342+t1348+t1353+t1379+t1391+t1402+t1407+t1411+t1413+t1419+t1423+t1436+t1443+t1445+t1454+t1457+t1486+t1487+t1767+t1827+t1873+t1992+t2130+t2180+t2474+t2481)-dq4.*(t300+t310+t373+t402+t403+t425+t441+t454+t457+t459+t470+t481+t489+t494+t513+t518+t521+t523+t525+t540+t548+t549+t568+t578+t582+t589+t590+t602+t609+t618+t625+t911+t971+t1158+t1449+t5916+t5934+t6386+t6396+t6426+t6434+t6580+t7010+t7031+t7410+t7413))-dq6.*(et374+et375+et376);
et628 = -dq2.*(-t7571-dq1.*t7584+dq4.*t7593+dq6.*t7599+dq5.*(-t5769+t5921+t5922+t5958-t5960+t5974+t5978+t6119+t6202+t6203+t6209+t6210-t6329+t6330+t6406-t6407+t6443-t6477+t6489+t6593-t6594-t7102+t7156-t7158+t7217+t7277+t7279+t7300+t7321+t7435+t7437+t7455+(t4119.*(et379+et380))./2.0+(t5658.*(et377+et378))./2.0+(t5662.*(et381+et382))./2.0+(t5940.*(et385+et386))./2.0+(t5939.*(et387+et388))./2.0+(t6462.*(et383+et384))./2.0));
et629 = dq4.*(t7149+dq2.*(et389+et390)+dq1.*t7596+dq6.*(et391+et392+et393+et394)+dq4.*(et395+et396+et397+et398+et399+et400+et401+et402+et403+et404+et405+et406)+dq5.*(t300+t310+t373+t402+t403+t425+t441+t454+t457+t459+t470+t481+t489+t494+t513+t518+t521+t523+t525+t540+t548+t549+t568+t578+t582+t589+t590+t602+t609+t618+t625+t911+t971+t1158+t1449+t5916+t5934+t6386+t6396+t6426+t6434+t6580+t7031+t7410+t7413))+dq1.*(t7580+dq2.*t7584+dq6.*t7587+dq4.*t7596-dq5.*t7595);
et630 = dq3.*(dq2.*(et412+et413+et414+et415+et416+et417+et418+et419+et420+et421+et422+et423+et424+et425+et426+et427+et428+et429+et430+et431+et432+et433+et434+et435+et436)+dq4.*t7148+dq5.*(et443+et444+et445+et446+et447+et448)-dq6.*(et461+et462+et463+et464+et465+et466)+dq1.*(et494+et495+et496+et497+et498+et499+et500+et501+et502+et503+et504+et505+et506+et507+et508+et509+et510+et511+et512+et513+et514+et515+et516+et517+et518+et519+et520+et521+et522+et523+et524+et525+et526+et527+et528+et529+et530+et531+et532+et533+et534+et535+et536+et537+et538+et539+et540+et541+et542+et543+et544+et545+et546+et547+et548+et549+et550+et551+et552+et553+et554+et555+et556+et557+et558+et559+et560+et561+et562+et563+et564+et565+et566+et567+et568+et569+et570+et571+et572+et573+et574+et575+et576+et577+et578+et579+et580+et581+et582+et583+et584+et585+et586+et587+et588+et589+et590+et591+et592+et593+et594+et595+et596+et597+et598+et599+et600+et601+et602+et603+et604+et605+et606+et607+et608+et609+et610+et611+et612+et613+et614+et615+et616+et617+et618+et619+et620+et621+et622+et623+et624+et625+et626));
et631 = -t121+(t6401.*(t5808-t6019+t5679.*(t2088-t4743).*3.038581678643136e-64))./2.0+t5.*t8.*4.35810366141993e-7+t5.*t3443-t9.*t3514-t615.*t6422;
et632 = (t6359.*(t5831-t6095+t5679.*(t2088-t4743).*8.081970098144003e-70))./2.0;
et633 = -t310+t357-t403+t411+t423+t425+t429+t440+t479+t480+t483+t488+t492+t532+t540+t545+t580+t581+t590+t604+t611+t618+t623+t911+t971+t1158+t1449+t5915-t5934+t6382+t6393-t6426-t6580+t7011-t7410-t7413+t3.*t8.*1.085068132002562e-9;
et634 = (t5894.*(t5770+t5852.*(t3136-t5691).*2.0+t5861.*(t7.*(t3719-t3788)+(t3.*t34.*t191.*(t29-t30))./8.112963841460668e+31).*2.0))./2.0+t3.*t5.*t8.*3.746051489620971e-7;
et635 = t3.*t8.*t9.*(-6.892170885479394e-7)+t4838.*t6230.*(t29-t30).*1.656182742171539e-72;
et636 = t199.*1.910352536348279e-6+t760+t3436+t5228+t5316+t5323+t5354+t5602+t5790+t5791+t5792+t5794+t5838+t5844+t5846+t5895+t5897+t5968+t5977+t5996+t6280+t6380+t6385+t6560+t6561+t7030+t7044+t7048+t7113;
et637 = t3.*t4.*5.724235841753608e-8;
et638 = t4.*t7.*t34.*t191.*(-2.142628988669224e-22);
et639 = -t5905+t6048+t6053-t6056+t6060-t6487+t6724+t6727-t6738+t6756+t6758+t6230.*(t5878+t9.*(t7.*(t3719-t3788)+(t3.*t34.*t191.*(t29-t30))./8.112963841460668e+31)).*4.126305279697715e-13-t150.*t5861.*t6468+t4.*t6216.*(t3136-t5691).*8.40184101230148e-6;
et640 = t4.*t6465.*(t3136-t5691).*4.126305279697715e-13;
et641 = t3.*(-3.133720214898255e-7)+t3.*t5.*1.773403438802817e-13;
et642 = t4.*t7.*5.358766382867102e-7+t3.*t9.*1.35232709518055e-13;
et643 = t3.*t15.*(-3.133720214898255e-7)+t3.*t18.*6.267440429796511e-7;
et644 = t3.*t20.*4.928108033652911e-8+t3.*t4.*t8.*2.536718707310641e-7;
et645 = t3.*t5.*t15.*1.773403438802817e-13-t3.*t5.*t18.*3.546806877605634e-13;
et646 = t3.*t9.*t15.*1.35232709518055e-13+t4.*t7.*t16.*5.358766382867102e-7;
et647 = t3.*t5.*t20.*3.446085442739697e-7-t3.*t9.*t18.*2.7046541903611e-13;
et648 = t4.*t7.*t19.*(-1.07175327657342e-6)+t3.*t9.*t20.*1.873025744810486e-7;
et649 = t4.*t7.*t21.*(-3.522340314041224e-7)+t3.*t16.*t20.*1.761170157020612e-7;
et650 = t3.*t20.*t21.*2.679383191433551e-7+t4.*t9.*t414-t3.*t4.*t5.*t8.*6.892170885479394e-7;
et651 = t3.*t4.*t8.*t9.*(-3.746051489620971e-7)+t4.*t5.*t7.*t9.*7.044680628082447e-7;
et652 = t3.*t4.*t8.*t19.*(-7.044680628082447e-7);
et653 = t3.*(-9.256477678042799e-10);
et654 = t196.*(-3.089169646176406e-8)+t197.*3.645726061228158e-7;
et655 = t199.*6.221689975285323e-7-t200.*8.79383415291399e-9;
et656 = t201.*(-5.943113753937517e-6);
et657 = t202.*4.620317820983189e-6+t738+t910+t930+t1019+t1077+t1212+t1659+t1835+t1938+t2052+t3457+t3479+t3542+t3584+t3612+t3667+t3732+t3875+t3922+t3968+t4286+t4349+t4370+t4553;
et658 = (t5925.*(t95-t4.*t9.*1.33637579258949e-4))./2.0-t4.*t7.*1.780811871872521e-7;
et659 = t7.*t8.*1.384445455377623e-7-t8.*t201.*2.951182896698924e-7;
et660 = t18.*t197.*(-7.291452122456316e-7)-t19.*t199.*1.246862701090643e-6+t116.*t202+t133.*t202+t166.*t197+t183.*t197+t8.*t866+t8.*t3383+t8.*t3450+t8.*t3476+t18.*t3492+t18.*t3582+(t613.*t4126)./2.0+t4.*t5787.*3.52553938621e-7;
et661 = t8.*t5786.*3.52553938621e-7-(t1531.*t6351)./2.0-(t1587.*t6352)./2.0-(t3444.*t5776)./2.0+(t3515.*t5775)./2.0-(t5778.*(t50-t53))./2.0+t5.*t9.*t199.*8.195682446929358e-7;
et662 = t3.*t34.*t191.*2.068448924867771e-23;
et663 = t7.*t34.*t191.*3.464776426798696e-24+t9.*t99.*t202+(t8.*t597.*t4119)./2.0-(t4.*t4119.*t4742)./2.0-(t4.*t4119.*(t81-t86))./2.0;
et664 = t3.*t4.*t34.*t191.*(-6.665726649850018e-22);
et665 = t3.*t8.*t34.*t191.*5.182094253151392e-22;
et666 = t4.*t7.*t34.*t191.*(-3.5299547261936e-23)+t7.*t8.*t34.*t191.*4.989293351605466e-25;
et667 = t3.*t18.*t34.*t191.*(-4.136897849735542e-23);
et668 = t3.*t4.*t8.*t34.*t191.*(-1.67439105057406e-23)+t4.*t7.*t19.*t34.*t191.*7.074233692313782e-23;
et669 = t4.*t5.*t7.*t9.*t34.*t191.*(-4.649924393989671e-23)+t3.*t4.*t5.*t8.*t9.*t34.*t191.*7.074233692313782e-23;
et670 = dq5.*(t5823+(t613.*(t5770+t5852.*(t3136-t5691).*2.0+t5861.*(t7.*(t3719-t3788)+(t3.*t34.*t191.*(t29-t30))./8.112963841460668e+31).*2.0))./2.0);
et671 = dq6.*(t90+t113+t131+t144+t148+t156+t158+t171+t185+(t3515.*(t5984+t5988-t6694-t6695+t6230.*(t5878+t9.*(t7.*(t3719-t3788)+(t3.*t34.*t191.*(t29-t30))./8.112963841460668e+31))+t4.*t6465.*(t3136-t5691)))./2.0+(t3444.*t7263)./2.0-(t4742.*t7053)./2.0-(t8.*(et639+et640))./2.0+t5.*t8.*t7362.*(3.0./1.0e+3)-t8.*t9.*t7363.*(3.0./1.0e+3)+(t4.*t5.*t7511)./2.0-(t4.*t9.*t7510)./2.0)+dq3.*(et641+et642+et643+et644+et645+et646+et647+et648+et649+et650+et651+et652)+dq2.*(et653+et654+et655+et656+et657+et658+et659+et660+et661+et662+et663+et664+et665+et666+et667+et668+et669);
et672 = t258+t277+t287+t356+t361+t372+t422+t433+t444+t448+t453+t475+t485+t493+t514+t524+t533+t561+t586+t592+t603+t610+t827+t899+t958+t972+t7076+t7310+t7312-t7373-t7375-t7378-t7429-t7430+t7440+t7463-t7515-t7516+t7517+t7519;
et673 = (t7362.*(t6313+(t91.*t5824.*(t6218+t5.*(t3136-t5691)))./1.316403645856965e+67+(t5824.*t6470.*(t29-t30))./1.316403645856965e+67))./2.0;
et674 = t197.*(-1.863093376486912e-7)+t199.*6.45106415957158e-10;
et675 = t201.*6.003953432070899e-6;
et676 = t202.*(-2.737706926505492e-6)-t1494+t1548-t1550+t1601+t1753+t1781+t1784-t1793-t1795+t1808-t1952+t2868-t4178+t4402+t4410+t4444+t4482-t4486+t4488-t4498+t4518-t5605-t5699+t5702-t5841-t5898+t5899+t5950-t5952-t6108+t6431+t6433-t7052+t7055-t7071+t7089+t7093+t7110+t7120+t7168+t7170+t7324;
et677 = (t6919.*(-t5881+t5918+t6412+t6414+(t4.*t5824.*t5861.*(t29-t30))./1.316403645856965e+67+(t4.*t91.*t5824.*(t3136-t5691))./1.316403645856965e+67))./2.0;
et678 = t8.*t201.*4.265809185498476e-7+t18.*t197.*3.726186752973823e-7;
et679 = (t7027.*(t6109+t6571+t6574-t6610+t4528.*(t4148+t5.*(t2421-t4158))+(t4838.*t6468.*(t29-t30))./1.316403645856965e+67))./2.0+(t5636.*(t50-t53))./2.0;
et680 = t3.*t34.*t191.*1.99727354193496e-23;
et681 = t7.*t34.*t191.*2.621936887592592e-22;
et682 = t3.*t4.*t34.*t191.*2.146558632488979e-23;
et683 = t3.*t8.*t34.*t191.*(-9.787964718254394e-24);
et684 = t4.*t7.*t34.*t191.*6.694747686175631e-26;
et685 = t7.*t8.*t34.*t191.*4.663711344199015e-25;
et686 = t3.*t18.*t34.*t191.*(-3.866940325762698e-23);
et687 = t3.*t4.*t8.*t34.*t191.*(-4.426946542131316e-23);
et688 = t1530+t1578+t1615+t1674+t1753-t1771+t1772+t1776+t1781+t1794-t1811+t1812+t1820+t1823+t1828+t1902-t1983+t1985+t1993-t2075+t2154-t2158+t2164+t2178+t2186-t2193+t2200+t2211+t2214+t2291+t2315+t2320+t2334+t2398+t2466+t2525+t4278+t4378+t4394+t4405+t4410+t4425+t4444+t4482+t4518+t4523+t4543+t4586+t4600-t4601-t4606-t4621-t4633-t4634+t4636+t4674+t4707+t4728-t4731+t4737-t4783+t18.*t1681+t18.*t1930+t17.*t2214+t17.*t2291-t5.*t17.*t190.*6.892170885479394e-7;
et689 = t9.*t17.*t190.*(-3.746051489620971e-7)-t17.*t18.*t190.*2.536718707310641e-7;
et690 = t3.*t34.*t191.*6.04484233343072e-23;
et691 = t7.*t34.*t191.*2.656233560274174e-22;
et692 = t4.*t8.*t22.*t190.*(-6.267440429796511e-7);
et693 = t3.*t4.*t34.*t191.*(-6.383525886533628e-22);
et694 = t3.*t5.*t34.*t191.*(-3.384729434006076e-29);
et695 = t3.*t8.*t34.*t191.*4.962704675595027e-22;
et696 = t4.*t7.*t34.*t191.*(-1.020706698179709e-22);
et697 = t3.*t9.*t34.*t191.*(-2.581060362977273e-29);
et698 = t5.*t7.*t34.*t191.*3.418055254602648e-22;
et699 = t7.*t8.*t34.*t191.*1.442682849549919e-24;
et700 = t7.*t9.*t34.*t191.*(-6.288707183017346e-22);
et701 = t3.*t18.*t34.*t191.*(-1.196207790875422e-22);
et702 = t18.*t19.*t22.*t190.*(-7.044680628082447e-7);
et703 = t3.*t4.*t8.*t34.*t191.*(-4.841597961614674e-23);
et704 = t3.*t5.*t8.*t34.*t191.*6.288707183017346e-22;
et705 = t4.*t5.*t7.*t34.*t191.*3.57486922061625e-23;
et706 = t5.*t9.*t18.*t22.*t190.*(-1.07175327657342e-6);
et707 = t3.*t8.*t9.*t34.*t191.*3.418055254602648e-22;
et708 = t4.*t7.*t9.*t34.*t191.*(-6.577221276854549e-23);
et709 = t5.*t7.*t8.*t34.*t191.*(-2.581060362977273e-29);
et710 = t7.*t8.*t9.*t34.*t191.*3.384729434006076e-29;
et711 = t3.*t5.*t18.*t34.*t191.*6.769458868012152e-29;
et712 = t3.*t9.*t18.*t34.*t191.*5.162120725954547e-29;
et713 = t4.*t7.*t19.*t34.*t191.*2.045555332665541e-22;
et714 = t5.*t8.*t17.*t34.*t191.*(-2.125369829239315e-23);
et715 = t8.*t9.*t22.*t34.*t191.*(-3.910360575273795e-23);
et716 = t8.*t17.*t19.*t34.*t191.*(-1.216145632129581e-22);
et717 = t3.*t4.*t5.*t8.*t34.*t191.*1.31544425537091e-22;
et718 = t3.*t4.*t8.*t9.*t34.*t191.*7.149738441232499e-23;
et719 = t4.*t5.*t7.*t9.*t34.*t191.*(-1.344552364866272e-22);
et720 = t3.*t5.*t7.*t18.*t34.*t191.*(-7.82072115054759e-23);
et721 = t3.*t4.*t8.*t19.*t34.*t191.*1.344552364866272e-22;
et722 = t3.*t7.*t9.*t18.*t34.*t191.*(-4.25073965847863e-23);
et723 = t5.*t8.*t9.*t22.*t34.*t191.*(-7.993777824483687e-23);
et724 = t3.*t4.*t5.*t8.*t9.*t34.*t191.*2.045555332665541e-22;
et725 = t236+t314+t410+t468-t529+t531+t6332-t6783+t5784.*(t4148+t5.*(t2421-t4158)).*7.26350610236655e-5+t91.*t5824.*(t6218+t5.*(t3136-t5691)).*1.015171749786156e-71;
et726 = t5.*t7.*t8.*(-3.546806877605634e-13)-t7.*t8.*t9.*2.7046541903611e-13;
et727 = t5824.*t6468.*(t29-t30).*5.517689141340903e-72;
et728 = t5824.*t6470.*(t29-t30).*1.015171749786156e-71;
et729 = dq4.*(t90+t113+t131+t144+t148+t156+t158+t171+t185)+dq6.*(t7439+t7521+t7522+t7531+t7554+t7555-t2096.*t7130-t2121.*t7129+t3523.*t6821+t3444.*t7130+t3515.*t7129)+dq2.*(t5845-t5951+t5954+t5973-t6276+t6546+t6548-t6557-t6562+t7142+t7226+t7234+t7237+t7386+t7388+(t3444.*(t4148+t5.*(t2421-t4158)))./2.0)+dq3.*(t258+t277+t287+t356+t361+t372+t422+t433+t444+t448+t453+t475+t485+t493+t514+t524+t533+t561+t586+t592+t603+t610+t827+t899+t958+t972+t7076+t7310+t7312-t7469+t7470-t7479-t7494-t7495+(t7053.*(et725+et726+et727+et728))./2.0);
et730 = -dq1.*(t742+t845+t866+t869+t877+t881+t919+t932+t947+t985+t998+t1031+t1075+t1184+t1213+t1227+t1661+t1758+t1798+t1831+t1858+t1995+t2038+t2068+t2083+t2113+t2132+t2266+t3321+t3407+t3409+t3430+t3450+t3463+t3468+t3475+t3485+t3490+t3496+t3499+t3507+t3513+t3522+t3526+t3531+t3543+t3569+t3583+t3585+t3592+t3618+t3635+t3658+t3734+t3738+t3753+t3761+t3783+t3819+t3843+t3869+t3871+t3956+t3978+t3992+t4183+t4208+t4232+t4259+t4327+t4337+t4369+t4382+t4388+t4436+t4473+t4556-t7296+t7337-t7339-t7387+t7465+(t7248.*(t5984+t5988-t6694-t6695+t6230.*(t5878+t9.*(t7.*(t3719-t3788)+(t3.*t34.*t191.*(t29-t30))./8.112963841460668e+31))+t4.*t6465.*(t3136-t5691)))./2.0);
et731 = dq5.*(-t115-t132+t2420+t2424+t3606+t3757+t6941+t7059+t7081+t7136+t7137+t7201+t7203+t7272+t7273);
et732 = dq5.*(t5825+t7258+dq6.*(-t115-t132-t2390+t2424+t3606+t3757+t6026+t6042+t6044+t6047+t6711+t6714+t6715+t6721+t6743+t6746+t6747+t6753+t6941+t7081+t7136+t7137+t7201+t7203+t7512+t7513)-dq5.*(et631+et632)+dq3.*(et633+et634+et635)-dq2.*(et636+et637+et638))+dq1.*(t7568+t7577+dq6.*t7087+dq5.*t7256-dq3.*t7596);
et733 = dq2.*(t7567+t7568-dq5.*t7572+dq3.*t7593+dq6.*(t5845-t5951+t5954+t5973-t6276+t6546+t6548-t6557-t6562+t7245-t7332+t7383-t7393-t7394-t7398-t7399+t7481+t7523+t7525+(t3444.*(t4148+t5.*(t2421-t4158)))./2.0+(t7511.*(t4148+t5.*(t2421-t4158)))./2.0+(t6352.*(t5709-t6255+t6282+t6296-t7003+t6216.*(t6218+t5.*(t3136-t5691)).*1.40259855e-11))./2.0))+dq4.*(et670+et671);
et734 = -dq3.*(t7149-dq5.*(t290+t357+t406+t411+t418+t423+t424+t429+t440+t449+t479+t480+t483+t488+t492+t532+t540+t545+t580+t581+t590+t604+t611+t618+t623+t911+t971+t986+t1324+t1670+t4100+t4132+t7011+t7143+t7222+t7224)+dq2.*(et674+et675+et676+et677+et678+et679+et680+et681+et682+et683+et684+et685+et686+et687)+dq1.*(et688+et689+et690+et691+et692+et693+et694+et695+et696+et697+et698+et699+et700+et701+et702+et703+et704+et705+et706+et707+et708+et709+et710+et711+et712+et713+et714+et715+et716+et717+et718+et719+et720+et721+et722+et723+et724)-dq6.*(et672+et673))+dq6.*(et729+et730+et731);
et735 = t72+t125-t616-t619+t1489+t1508-t5676.*2.179051830709965e-7+t6195.*2.179051830709965e-7+t6196.*4.00912737776847e-7-t6226.*2.179051830709965e-7;
et736 = t6252.*(-2.179051830709965e-7)+t6928.*2.179051830709965e-7+t6935.*2.179051830709965e-7+t6936.*4.00912737776847e-7;
et737 = t6213.*(t6218+t5.*(t3136-t5691)).*(-4.00912737776847e-7)+t72.*t5666+t72.*t6220+t72.*t6239+(t9.*t7486)./2.0+(t640.*t7077)./2.0-(t1460.*t7191)./2.0+(t1471.*t7192)./2.0+(t5.*(t5676.*(-1.246862701090643e-6)+t5730+t5967+t6244+t6249+t6289+t6293+t6307+t6312+t6648+t6656+t6946+t6953+t6977+t6984))./2.0;
et738 = t5888+t5795.*(t2088-t4743).*8.081970098144003e-70;
et739 = t5683.*(t197.*(t29-t30).*9.007199254740992e+15+t3.*(t2444-t2449)).*8.081970098144003e-70;
et740 = t5842+t5795.*(t2088-t4743).*3.038581678643136e-64;
et741 = t5683.*(t197.*(t29-t30).*9.007199254740992e+15+t3.*(t2444-t2449)).*3.038581678643136e-64;
et742 = t6008+t6123-t6672+(t5684.*t6468.*(t29-t30))./1.316403645856965e+67-(t5.*t91.*t5824.*t6216)./1.316403645856965e+67;
et743 = (t5.*t5824.*t6230.*(t29-t30))./1.316403645856965e+67;
et744 = t284-t311+t391-t463+t534+t5947-t6009.*1.40259855e-11+t6013.*7.26350610236655e-5-t6194+t6449+t6454-t6513+t6544+t6551;
et745 = t91.*t5684.*(t6218+t5.*(t3136-t5691)).*1.065477564130357e-78-t4.*t7.*t9.*1.07175327657342e-6;
et746 = t5824.*t6222.*(t29-t30).*5.517689141340903e-72;
et747 = t5684.*t6470.*(t29-t30).*1.065477564130357e-78;
et748 = t4.*4.493955935826494e-9-t8.*6.45106415957158e-10+t5930.*2.180205e-5;
et749 = t6013.*2.180205e-5+(t6359.*(et738+et739))./2.0-t3.*t4.*3.344600550825411e-6;
et750 = t3.*t8.*1.525084462760484e-6-t4.*t7.*1.085068132002562e-9;
et751 = t7.*t8.*(-7.558827895633446e-9)-t8.*t9.*2.048803907774054e-7+t8.*t277-(t349.*t640)./2.0+(t435.*t1460)./2.0-(t432.*t1471)./2.0;
et752 = t9.*t7215.*7.01299275e-12+(t5.*t7421)./2.0-(t1426.*t7176)./2.0+(t5826.*t6422)./2.0+(t6401.*(et740+et741))./2.0+t5.*(et742+et743).*7.01299275e-12+(t9.*(et744+et745+et746+et747))./2.0;
